simulink model "model1"  (R2024a)
settings: Solver=VariableStepAuto  StartTime=0.0  StopTime=simulation_time  RelTol=1e-3
values from neighbouring files (symbols this model uses):
  dq_0 = zeros(n, 1)    [example.m]
  path = @(t) circle_center + u_circle_plane*radius*cos((t/T) * (2*pi)) + v_circle_plane*radius*sin((t/T) * (2*pi))    [example.m]
  path_ddot = @(t) -u_circle_plane*radius*(2*pi/T)*(2*pi/T)*cos((t/T) * (2*pi)) - v_circle_plane*radius*(2*pi/T)*(2*pi/T)*sin((t/T) * (2*pi))    [example.m]
  path_dot = @(t) -u_circle_plane*radius*(2*pi/T)*sin((t/T) * (2*pi)) + v_circle_plane*radius*(2*pi/T)*cos((t/T) * (2*pi))    [example.m]
  q_0 = randn(n, 1)    [example.m]
  robot_model = importrobot("../robot_model/kuka-lwr-4plus/model1.urdf", 'DataFormat', 'column')    [example.m]
undefined symbols (not defined in the file or in its folder): torque_low_bound, torque_up_bound, X, Y, Z
libraries: sm_lib x74, nesl_utility x8, robotmaniplib x4
(part 4 of 5)

== matlab function model1/MATLAB Function5 ==
  data: currJointPos input; c_num output; currJointVel input
function c_num = c_num1(currJointPos, currJointVel)
%C_NUM1
%    C_NUM = C_NUM1(Q2,Q3,Q4,Q5,Q6,Q7,Q_DOT1,Q_DOT2,Q_DOT3,Q_DOT4,Q_DOT5,Q_DOT6,Q_DOT7)

%    This function was generated by the Symbolic Math Toolbox version 24.1.
%    01-Jul-2024 12:17:30

q_dot1 = currJointVel(1);
q2 = currJointPos(2);
q_dot2 = currJointVel(2);
q3 = currJointPos(3);
q_dot3 = currJointVel(3);
q4 = currJointPos(4);
q_dot4 = currJointVel(4);
q5 = currJointPos(5);
q_dot5 = currJointVel(5);
q6 = currJointPos(6);
q_dot6 = currJointVel(6);
q7 = currJointPos(7);
q_dot7 = currJointVel(7);


t2 = cos(q2);
t3 = cos(q3);
t4 = cos(q4);
t5 = cos(q5);
t6 = cos(q6);
t7 = cos(q7);
t8 = sin(q2);
t9 = sin(q3);
t10 = sin(q4);
t11 = sin(q5);
t12 = sin(q6);
t13 = sin(q7);
t14 = t3.^2;
t15 = t4.^2;
t16 = t5.^2;
t17 = t6.^2;
t18 = t7.^2;
t19 = t8.^2;
t20 = t9.^2;
t21 = t10.^2;
t22 = t11.^2;
t23 = t12.^2;
t24 = t13.^2;
t25 = t2.*t4;
t26 = t3.*t5;
t27 = t4.*t6;
t28 = t5.*t7;
t29 = t2.*t10;
t30 = t4.*t8;
t31 = t3.*t11;
t32 = t5.*t9;
t33 = t4.*t12;
t34 = t6.*t10;
t35 = t5.*t13;
t36 = t7.*t11;
t37 = t8.*t10;
t38 = t9.*t11;
t39 = t10.*t12;
t40 = t11.*t13;
t41 = t3.*(2.0./5.0);
t42 = t9.*(2.0./5.0);
t88 = t3.*(7.0./1.0e+2);
t89 = t9.*(7.0./1.0e+2);
t91 = t3.*t4.*(3.0./5.0e+1);
t92 = t3.*t10.*(-2.0./5.0);
t95 = t3.*t10.*(3.0./5.0e+1);
t96 = t4.*t9.*(3.0./5.0e+1);
t97 = t9.*t10.*(-2.0./5.0);
t100 = t9.*t10.*(3.0./5.0e+1);
t101 = t2.*(1.3e+1./1.0e+2);
t102 = t4.*(3.1e+1./2.5e+2);
t103 = t8.*(1.3e+1./1.0e+2);
t104 = t10.*(3.1e+1./2.5e+2);
t135 = t2.*t9.*(2.3e+1./5.0e+1);
t140 = t4.*t9.*(7.0./2.5e+2);
t142 = t8.*t9.*(2.3e+1./5.0e+1);
t145 = t3.*4.2e-3;
t146 = t2.*7.8e-3;
t147 = t9.*4.2e-3;
t148 = t8.*7.8e-3;
t182 = t4.*t11.*(3.9e+1./1.0e+2);
t194 = t10.*t11.*(3.9e+1./1.0e+2);
t198 = q_dot5.*t12.*6.0e-5;
t199 = q_dot6.*t12.*6.0e-5;
t200 = q_dot7.*t12.*6.0e-5;
t226 = t3.*t10.*(-3.1e+1./2.5e+2);
t228 = t3.*t10.*1.05e-2;
t236 = t6.*t12.*1.2e-4;
t275 = t2.*t9.*7.15e-2;
t278 = t2.*t9.*(-7.8e-3);
t279 = t2.*t9.*5.1e-3;
t282 = t3.*t10.*5.1e-3;
t283 = t3.*t10.*6.3e-3;
t285 = t9.*t10.*(-4.2e-3);
t286 = t8.*t9.*5.1e-3;
t287 = t9.*t10.*5.1e-3;
t296 = q_dot4.*t5.*t12.*6.0e-5;
t297 = q_dot4.*t6.*t11.*6.0e-5;
t299 = q_dot6.*t6.*t11.*6.0e-5;
t301 = q_dot7.*t6.*t11.*6.0e-5;
t393 = t2.*t9.*6.37e-2;
t394 = t4.*t11.*9.672e-2;
t395 = t5.*t10.*9.672e-2;
t422 = t3.*t4.*t9.*(-4.2e-3);
t752 = t2.*2.283333333335e-2;
t753 = t8.*2.283333333335e-2;
t754 = t3.*1.083333333335e-2;
t756 = t9.*1.083333333335e-2;
t867 = t11.*1.33541666666835e-3;
t868 = t9.*1.573333333335e-2;
t897 = t8.*3.973333333335e-2;
t918 = t5.*t10.*1.33541666666835e-3;
t922 = t3.*t8.*1.573333333335e-2;
t936 = t3.*t9.*7.82666666667e-2;
t951 = t2.*t8.*3.02666666667e-2;
t964 = t4.*t10.*1.133599999999999e-2;
t1081 = t5.*t11.*2.2065050000003e-1;
t1114 = t10.*3.751275000001835e-2;
t1208 = t4.*t9.*3.751275000001835e-2;
t1271 = t3.*t10.*(-3.751275000001835e-2);
t43 = t8.*t38;
t44 = t9.*t39;
t45 = t10.*t40;
t46 = t3.*t25;
t47 = t4.*t26;
t48 = t5.*t27;
t49 = t6.*t28;
t50 = t3.*t29;
t51 = t3.*t30;
t52 = t2.*t32;
t53 = t8.*t26;
t54 = t4.*t31;
t55 = t4.*t32;
t56 = t3.*t34;
t57 = t9.*t27;
t58 = t5.*t33;
t59 = t5.*t34;
t60 = t4.*t36;
t61 = t10.*t28;
t62 = t6.*t35;
t63 = t6.*t36;
t64 = t3.*t37;
t65 = t2.*t38;
t66 = t8.*t31;
t67 = t8.*t32;
t68 = t4.*t38;
t69 = t3.*t39;
t70 = t9.*t33;
t71 = t9.*t34;
t72 = t5.*t39;
t73 = t4.*t40;
t74 = t10.*t35;
t75 = t10.*t36;
t76 = t6.*t40;
t77 = t2.*t41;
t78 = t4.*t41;
t79 = t26.*(2.0./5.0);
t80 = t8.*t41;
t81 = t10.*t41;
t82 = t4.*t42;
t83 = t31.*(2.0./5.0);
t84 = t32.*(2.0./5.0);
t85 = t8.*t42;
t86 = t10.*t42;
t87 = t38.*(2.0./5.0);
t90 = t25.*(3.0./5.0e+1);
t93 = t29.*(3.0./5.0e+1);
t94 = t30.*(3.0./5.0e+1);
t99 = t37.*(3.0./5.0e+1);
t105 = t30.*t32;
t106 = t32.*t34;
t107 = t34.*t36;
t110 = t30.*t38;
t112 = t32.*t39;
t114 = t34.*t40;
t119 = t9.*t12.*t37;
t120 = t10.*t13.*t38;
t129 = t25.*(7.0./1.0e+2);
t130 = t4.*t88;
t131 = t37.*t42;
t133 = t39.*t42;
t136 = t2.*t89;
t137 = t8.*t88;
t138 = t29.*(7.0./1.0e+2);
t139 = t4.*t89;
t141 = -t100;
t143 = t8.*t89;
t144 = t37.*(7.0./1.0e+2);
t151 = t27.*t41;
t152 = t25.*t42;
t153 = t30.*t41;
t159 = t33.*t41;
t160 = t34.*t41;
t161 = t29.*t42;
t162 = t37.*t41;
t163 = t30.*t42;
t168 = t39.*t41;
t169 = t34.*t42;
t170 = t26.*(3.9e+1./1.0e+2);
t171 = t28.*(3.9e+1./1.0e+2);
t172 = t25.*(3.1e+1./2.5e+2);
t173 = t26.*(3.1e+1./2.5e+2);
t174 = t26.*1.5e-3;
t175 = t9.*t37.*(-2.0./5.0);
t178 = -t135;
t180 = t31.*(3.9e+1./1.0e+2);
t181 = t32.*(3.9e+1./1.0e+2);
t183 = t35.*(3.9e+1./1.0e+2);
t184 = t36.*(3.9e+1./1.0e+2);
t186 = t29.*(3.1e+1./2.5e+2);
t187 = t30.*(3.1e+1./2.5e+2);
t189 = t9.*t102;
t190 = t31.*(3.1e+1./2.5e+2);
t191 = t31.*1.5e-3;
t192 = t32.*1.5e-3;
t193 = t38.*(3.9e+1./1.0e+2);
t195 = t40.*(3.9e+1./1.0e+2);
t196 = t9.*t104;
t197 = t38.*(3.1e+1./2.5e+2);
t209 = t10.*t26.*(-2.0./5.0);
t213 = t9.*t29.*(-2.0./5.0);
t215 = t9.*t30.*(-2.0./5.0);
t221 = t25.*4.2e-3;
t222 = t27.*6.0e-5;
t223 = t9.*t37.*(-3.0./5.0e+1);
t224 = -t182;
t227 = t31.*(3.1e+1./6.25e+2);
t229 = t30.*8.4e-3;
t230 = t2.*t147;
t231 = t8.*t145;
t232 = t29.*4.2e-3;
t233 = t30.*4.2e-3;
t234 = t10.*t145;
t237 = t33.*6.0e-5;
t238 = t34.*6.0e-5;
t241 = t8.*t147;
t243 = t9.*t148;
t261 = t9.*t25.*(7.0./2.5e+2);
t266 = t30.*t89;
t267 = t25.*5.1e-3;
t271 = t9.*t37.*(3.1e+1./2.5e+2);
t280 = t29.*5.1e-3;
t281 = t30.*5.1e-3;
t284 = -t236;
t298 = t5.*t198;
t300 = t5.*t200;
t343 = t32.*t104;
t347 = t9.*t37.*1.05e-2;
t350 = t12.*t38.*6.0e-5;
t351 = -t275;
t352 = -t279;
t354 = -t283;
t355 = -t287;
t360 = t10.*t26.*(3.1e+1./6.25e+2);
t366 = t3.*t8.*t146;
t367 = t12.*t25.*6.0e-5;
t368 = t6.*t29.*6.0e-5;
t372 = t12.*t26.*6.0e-5;
t373 = t6.*t31.*6.0e-5;
t390 = t9.*t37.*(-4.2e-3);
t391 = t9.*t37.*5.1e-3;
t392 = t9.*t37.*6.3e-3;
t396 = t32.*4.836e-2;
t405 = q_dot3.*t11.*t39.*6.0e-5;
t406 = q_dot5.*t11.*t39.*6.0e-5;
t407 = q_dot7.*t11.*t39.*6.0e-5;
t423 = t9.*t25.*2.1e-3;
t433 = -t393;
t434 = -t394;
t449 = t28.*t34.*(-3.9e+1./1.0e+2);
t450 = t25.*t32.*(3.1e+1./6.25e+2);
t451 = t26.*t30.*(3.1e+1./6.25e+2);
t461 = t32.*t37.*(3.1e+1./6.25e+2);
t469 = t11.*t12.*t29.*6.0e-5;
t470 = t5.*t12.*t37.*6.0e-5;
t475 = t11.*t37.*4.836e-2;
t476 = t10.*t38.*4.836e-2;
t480 = t20.*t30.*2.1e-3;
t485 = t5.*t6.*t29.*(-6.0e-5);
t486 = t26.*t33.*(-6.0e-5);
t492 = t33.*t38.*(-6.0e-5);
t495 = t11.*t25.*4.836e-2;
t519 = t12.*t30.*t31.*6.0e-5;
t528 = t6.*t12.*t16.*3.042e-2;
t530 = t91+t97;
t531 = t25.*t31.*4.836e-2;
t532 = t31.*t37.*4.836e-2;
t542 = t101+t142;
t547 = t102+t194;
t564 = t4.*t10.*t17.*t22.*1.521e-1;
t565 = t5.*t11.*t17.*t21.*1.521e-1;
t568 = t4.*t10.*t22.*t23.*1.8252e-1;
t569 = t5.*t11.*t21.*t23.*1.8252e-1;
t570 = t6.*t12.*t21.*t22.*3.042e-2;
t586 = t147+t282;
t587 = t146+t286;
t779 = t29.*2.080133333335e-2;
t780 = t30.*2.080133333335e-2;
t785 = t2.*t756;
t786 = t8.*t754;
t787 = t8.*t756;
t789 = t25.*1.533333333335e-2;
t791 = t29.*1.533333333335e-2;
t794 = t37.*1.533333333335e-2;
t796 = t26.*2.170133333335e-2;
t797 = t31.*2.170133333335e-2;
t799 = t25.*2.080133333335e-2;
t800 = t38.*2.170133333335e-2;
t804 = t26.*1.302083333335e-3;
t805 = t27.*1.302083333335e-3;
t806 = t31.*1.302083333335e-3;
t807 = t32.*1.302083333335e-3;
t808 = t33.*1.302083333335e-3;
t809 = t34.*1.302083333335e-3;
t810 = t39.*1.302083333335e-3;
t870 = t28.*3.333333333335e-5;
t873 = t35.*3.333333333335e-5;
t874 = t36.*3.333333333335e-5;
t875 = t40.*3.333333333335e-5;
t890 = t3.*t9.*t21.*4.16026666667e-2;
t896 = -t868;
t900 = t3.*t9.*t15.*3.06666666667e-2;
t915 = t31.*1.33541666666835e-3;
t916 = t32.*1.33541666666835e-3;
t917 = t4.*t867;
t921 = t2.*t868;
t949 = t8.*t15.*t20.*1.533333333335e-2;
t954 = t9.*t16.*t21.*2.170133333335e-2;
t962 = t8.*t20.*t21.*2.080133333335e-2;
t963 = -t936;
t969 = t8.*t14.*3.913333333335e-2;
t972 = t8.*t20.*2.5328333333335e-1;
t975 = t25.*t867;
t976 = t5.*t29.*1.33541666666835e-3;
t979 = t9.*t21.*3.117999999999997e-3;
t982 = t37.*t867;
t983 = t10.*t38.*1.33541666666835e-3;
t984 = -t951;
t992 = t6.*t12.*t18.*6.66666666667e-5;
t997 = t6.*t12.*t24.*6.66666666667e-5;
t1007 = t9.*t15.*1.0568e-2;
t1025 = t2.*t8.*t14.*5.116666666667e-1;
t1040 = t3.*t9.*t19.*5.065666666667e-1;
t1042 = t26.*t30.*1.33541666666835e-3;
t1063 = t4.*t10.*t22.*5.60416666667e-3;
t1065 = t4.*t10.*t20.*1.603599999999999e-2;
t1089 = t10.*t17.*2.666666666665e-5;
t1090 = t11.*t17.*2.666666666665e-5;
t1091 = t11.*t23.*2.666666666665e-5;
t1094 = -t1081;
t1099 = t9.*t21.*t22.*2.802083333335e-3;
t1101 = t12.*t27.*5.33333333333e-5;
t1103 = t278+t753;
t1107 = t285+t754;
t1113 = t5.*t11.*t23.*1.7979583333333e-1;
t1125 = t5.*t11.*t17.*1.4949583333333e-1;
t1128 = t23.*t31.*2.666666666665e-5;
t1130 = t5.*t10.*t23.*2.666666666665e-5;
t1145 = t6.*t12.*t25.*5.33333333333e-5;
t1149 = t6.*t12.*t38.*2.666666666665e-5;
t1150 = t11.*t12.*t34.*5.33333333333e-5;
t1151 = t4.*t10.*t16.*5.304546666667e-1;
t1165 = t17.*t29.*2.666666666665e-5;
t1166 = t17.*t30.*2.666666666665e-5;
t1168 = t4.*t9.*t17.*2.666666666665e-5;
t1169 = t17.*t31.*2.666666666665e-5;
t1177 = t4.*t11.*t23.*(-2.666666666665e-5);
t1205 = t29.*3.751275000001835e-2;
t1206 = t30.*3.751275000001835e-2;
t1207 = t3.*t1114;
t1213 = t4.*t11.*t17.*(-2.666666666665e-5);
t1214 = t5.*t10.*t17.*(-2.666666666665e-5);
t1230 = t5.*t6.*t12.*t25.*2.666666666665e-5;
t1231 = t12.*t26.*t27.*2.666666666665e-5;
t1248 = t5.*t11.*t21.*5.2485050000003e-1;
t1266 = t5.*t23.*t29.*2.666666666665e-5;
t1268 = t9.*t17.*t37.*2.666666666665e-5;
t1284 = t10.*t16.*t17.*(-2.666666666665e-5);
t1290 = t10.*t17.*t22.*(-2.666666666665e-5);
t1291 = t10.*t16.*3.560400000001665e-2;
t1292 = t10.*t22.*3.560400000001665e-2;
t1307 = t5.*t17.*t29.*(-2.666666666665e-5);
t1313 = t9.*t37.*3.751275000001835e-2;
t1320 = t6.*t12.*t25.*t26.*2.666666666665e-5;
t1338 = t23.*t26.*t30.*2.666666666665e-5;
t98 = -t87;
t108 = -t47;
t109 = -t49;
t111 = t8.*t71;
t113 = t9.*t75;
t115 = -t50;
t116 = -t51;
t117 = -t58;
t118 = -t59;
t123 = -t68;
t128 = -t76;
t132 = t43.*(2.0./5.0);
t134 = -t94;
t150 = t47.*(2.0./5.0);
t154 = t2.*t83;
t155 = t53.*(2.0./5.0);
t156 = t54.*(2.0./5.0);
t157 = t10.*t79;
t158 = t55.*(2.0./5.0);
t164 = t66.*(2.0./5.0);
t165 = t67.*(2.0./5.0);
t166 = t10.*t83;
t167 = t68.*(2.0./5.0);
t179 = -t138;
t201 = -t106;
t203 = t46.*(3.0./5.0e+1);
t204 = -t110;
t207 = -t114;
t211 = t50.*(3.0./5.0e+1);
t212 = t51.*(3.0./5.0e+1);
t214 = t64.*(-2.0./5.0);
t219 = t64.*(3.0./5.0e+1);
t220 = t9.*t94;
t225 = -t186;
t239 = -t193;
t240 = -t197;
t244 = t25.*t84;
t245 = t30.*t79;
t246 = t25.*t87;
t247 = t30.*t83;
t248 = t30.*t84;
t251 = t27.*t85;
t252 = t46.*(7.0./1.0e+2);
t253 = t30.*t87;
t254 = t37.*t84;
t255 = t12.*t161;
t256 = t12.*t162;
t260 = t51.*(7.0./1.0e+2);
t262 = t51.*(7.0./2.5e+2);
t264 = t12.*t131;
t265 = t64.*(7.0./1.0e+2);
t268 = t43.*(3.9e+1./1.0e+2);
t269 = t10.*t193;
t270 = t45.*(3.9e+1./1.0e+2);
t272 = t43.*(3.1e+1./2.5e+2);
t273 = t43.*1.5e-3;
t274 = -t227;
t276 = -t229;
t277 = -t233;
t288 = t25+t64;
t289 = t37+t46;
t290 = t31+t55;
t291 = t32+t54;
t292 = t27+t72;
t293 = t39+t48;
t294 = t35+t63;
t295 = t36+t62;
t304 = t105.*(-2.0./5.0);
t305 = t6.*t213;
t306 = t47.*(3.9e+1./1.0e+2);
t307 = t4.*t171;
t308 = t49.*(3.9e+1./1.0e+2);
t309 = t47.*(3.1e+1./2.5e+2);
t311 = t12.*t215;
t313 = t52.*(3.9e+1./1.0e+2);
t314 = t53.*(3.9e+1./1.0e+2);
t315 = t54.*(3.9e+1./1.0e+2);
t316 = t55.*(3.9e+1./1.0e+2);
t317 = t4.*t183;
t318 = t61.*(3.9e+1./1.0e+2);
t319 = t62.*(3.9e+1./1.0e+2);
t320 = t63.*(3.9e+1./1.0e+2);
t322 = t50.*(3.1e+1./2.5e+2);
t323 = t51.*(3.1e+1./2.5e+2);
t324 = t55.*(3.1e+1./2.5e+2);
t325 = t52.*1.5e-3;
t326 = t53.*1.5e-3;
t327 = t54.*1.5e-3;
t328 = t55.*1.5e-3;
t330 = t65.*(3.9e+1./1.0e+2);
t331 = t66.*(3.9e+1./1.0e+2);
t332 = t67.*(3.9e+1./1.0e+2);
t333 = t68.*(3.9e+1./1.0e+2);
t334 = t10.*t181;
t335 = t74.*(3.9e+1./1.0e+2);
t336 = t75.*(3.9e+1./1.0e+2);
t337 = t76.*(3.9e+1./1.0e+2);
t338 = t64.*(3.1e+1./2.5e+2);
t339 = t65.*(3.1e+1./2.5e+2);
t340 = t66.*(3.1e+1./2.5e+2);
t341 = t67.*(3.1e+1./2.5e+2);
t342 = t68.*(3.1e+1./2.5e+2);
t344 = t67.*1.5e-3;
t345 = t68.*1.5e-3;
t346 = t43.*(3.1e+1./6.25e+2);
t349 = t44.*6.0e-5;
t353 = -t281;
t359 = t2.*t227;
t361 = t55.*(3.1e+1./6.25e+2);
t362 = t50.*8.4e-3;
t363 = t50.*4.2e-3;
t364 = t51.*4.2e-3;
t369 = t8.*t222;
t370 = t56.*6.0e-5;
t371 = t57.*6.0e-5;
t374 = t58.*6.0e-5;
t375 = t59.*6.0e-5;
t385 = t64.*4.2e-3;
t386 = t71.*6.0e-5;
t387 = t72.*6.0e-5;
t389 = -t347;
t408 = t27.*t184;
t410 = t105.*(3.9e+1./1.0e+2);
t411 = t27.*t195;
t412 = t34.*t183;
t413 = t107.*(3.9e+1./1.0e+2);
t414 = t105.*(3.1e+1./2.5e+2);
t415 = t110.*(3.9e+1./1.0e+2);
t416 = t114.*(3.9e+1./1.0e+2);
t417 = t110.*1.5e-3;
t418 = -t360;
t424 = t50.*5.1e-3;
t425 = t51.*5.1e-3;
t426 = -t368;
t429 = t64.*5.1e-3;
c_num = ft_1({q_dot1,q_dot2,q_dot3,q_dot4,q_dot5,q_dot6,q_dot7,t10,t1007,t102,t1025,t103,t104,t1040,t1042,t105,t106,t1063,t1065,t107,t108,t1089,t109,t1090,t1091,t1094,t1099,t11,t110,t1101,t1103,t1107,t111,t1113,t1114,t112,t1125,t1128,t113,t1130,t114,t1145,t1149,t115,t1150,t1151,t116,t1165,t1166,t1168,t1169,t117,t1177,t118,t119,t12,t120,t1205,t1206,t1207,t1208,t1213,t1214,t123,t1230,t1231,t1248,t1266,t1268,t1271,t128,t1284,t129,t1290,t1291,t1292,t13,t130,t1307,t131,t1313,t132,t1320,t133,t1338,t134,t136,t137,t139,t140,t141,t143,t144,t145,t147,t148,t150,t151,t152,t153,t154,t155,t156,t157,t158,t159,t16,t160,t161,t162,t163,t164,t165,t166,t167,t168,t169,t17,t170,t171,t172,t173,t174,t175,t178,t179,t180,t181,t183,t184,t187,t189,t190,t191,t192,t195,t196,t198,t199,t2,t200,t201,t203,t204,t207,t209,t211,t212,t213,t214,t219,t22,t220,t221,t222,t223,t224,t225,t226,t227,t228,t23,t230,t231,t232,t234,t237,t238,t239,t240,t241,t243,t244,t245,t246,t247,t248,t25,t251,t252,t253,t254,t255,t256,t26,t260,t261,t262,t264,t265,t266,t267,t268,t269,t27,t270,t271,t272,t273,t274,t276,t277,t28,t280,t284,t288,t289,t29,t290,t291,t292,t293,t294,t295,t296,t297,t298,t299,t3,t30,t300,t301,t304,t305,t306,t307,t308,t309,t31,t311,t313,t314,t315,t316,t317,t318,t319,t32,t320,t322,t323,t324,t325,t326,t327,t328,t33,t330,t331,t332,t333,t334,t335,t336,t337,t338,t339,t34,t340,t341,t342,t343,t344,t345,t346,t349,t35,t350,t351,t352,t353,t354,t355,t359,t36,t361,t362,t363,t364,t366,t367,t369,t37,t370,t371,t372,t373,t374,t375,t38,t385,t386,t387,t389,t39,t390,t391,t392,t395,t396,t4,t40,t405,t406,t407,t408,t41,t410,t411,t412,t413,t414,t415,t416,t417,t418,t42,t422,t423,t424,t425,t426,t429,t43,t433,t434,t44,t449,t45,t450,t451,t46,t461,t469,t47,t470,t475,t476,t48,t480,t485,t486,t49,t492,t495,t5,t50,t51,t519,t52,t528,t53,t530,t531,t532,t54,t542,t547,t55,t56,t564,t565,t568,t569,t57,t570,t58,t586,t587,t59,t6,t60,t61,t62,t63,t64,t65,t66,t67,t68,t69,t7,t70,t71,t72,t73,t74,t75,t752,t756,t76,t77,t779,t78,t780,t785,t786,t787,t789,t79,t791,t794,t796,t797,t799,t8,t80,t800,t804,t805,t806,t807,t808,t809,t81,t810,t82,t83,t84,t85,t86,t867,t868,t870,t873,t874,t875,t88,t89,t890,t896,t897,t9,t90,t900,t915,t916,t917,t918,t92,t921,t922,t93,t949,t95,t954,t96,t962,t963,t964,t969,t972,t975,t976,t979,t98,t982,t983,t984,t99,t992,t997});
end
function c_num = ft_1(ct)
[q_dot1,q_dot2,q_dot3,q_dot4,q_dot5,q_dot6,q_dot7,t10,t1007,t102,t1025,t103,t104,t1040,t1042,t105,t106,t1063,t1065,t107,t108,t1089,t109,t1090,t1091,t1094,t1099,t11,t110,t1101,t1103,t1107,t111,t1113,t1114,t112,t1125,t1128,t113,t1130,t114,t1145,t1149,t115,t1150,t1151,t116,t1165,t1166,t1168,t1169,t117,t1177,t118,t119,t12,t120,t1205,t1206,t1207,t1208,t1213,t1214,t123,t1230,t1231,t1248,t1266,t1268,t1271,t128,t1284,t129,t1290,t1291,t1292,t13,t130,t1307,t131,t1313,t132,t1320,t133,t1338,t134,t136,t137,t139,t140,t141,t143,t144,t145,t147,t148,t150,t151,t152,t153,t154,t155,t156,t157,t158,t159,t16,t160,t161,t162,t163,t164,t165,t166,t167,t168,t169,t17,t170,t171,t172,t173,t174,t175,t178,t179,t180,t181,t183,t184,t187,t189,t190,t191,t192,t195,t196,t198,t199,t2,t200,t201,t203,t204,t207,t209,t211,t212,t213,t214,t219,t22,t220,t221,t222,t223,t224,t225,t226,t227,t228,t23,t230,t231,t232,t234,t237,t238,t239,t240,t241,t243,t244,t245,t246,t247,t248,t25,t251,t252,t253,t254,t255,t256,t26,t260,t261,t262,t264,t265,t266,t267,t268,t269,t27,t270,t271,t272,t273,t274,t276,t277,t28,t280,t284,t288,t289,t29,t290,t291,t292,t293,t294,t295,t296,t297,t298,t299,t3,t30,t300,t301,t304,t305,t306,t307,t308,t309,t31,t311,t313,t314,t315,t316,t317,t318,t319,t32,t320,t322,t323,t324,t325,t326,t327,t328,t33,t330,t331,t332,t333,t334,t335,t336,t337,t338,t339,t34,t340,t341,t342,t343,t344,t345,t346,t349,t35,t350,t351,t352,t353,t354,t355,t359,t36,t361,t362,t363,t364,t366,t367,t369,t37,t370,t371,t372,t373,t374,t375,t38,t385,t386,t387,t389,t39,t390,t391,t392,t395,t396,t4,t40,t405,t406,t407,t408,t41,t410,t411,t412,t413,t414,t415,t416,t417,t418,t42,t422,t423,t424,t425,t426,t429,t43,t433,t434,t44,t449,t45,t450,t451,t46,t461,t469,t47,t470,t475,t476,t48,t480,t485,t486,t49,t492,t495,t5,t50,t51,t519,t52,t528,t53,t530,t531,t532,t54,t542,t547,t55,t56,t564,t565,t568,t569,t57,t570,t58,t586,t587,t59,t6,t60,t61,t62,t63,t64,t65,t66,t67,t68,t69,t7,t70,t71,t72,t73,t74,t75,t752,t756,t76,t77,t779,t78,t780,t785,t786,t787,t789,t79,t791,t794,t796,t797,t799,t8,t80,t800,t804,t805,t806,t807,t808,t809,t81,t810,t82,t83,t84,t85,t86,t867,t868,t870,t873,t874,t875,t88,t89,t890,t896,t897,t9,t90,t900,t915,t916,t917,t918,t92,t921,t922,t93,t949,t95,t954,t96,t962,t963,t964,t969,t972,t975,t976,t979,t98,t982,t983,t984,t99,t992,t997] = ct{:};
t431 = -t391;
t432 = -t392;
t435 = -t396;
t452 = t6.*t50.*6.0e-5;
t454 = t5.*t367;
t457 = t32.*t222;
t463 = t12.*t64.*6.0e-5;
t465 = t12.*t65.*6.0e-5;
t466 = t12.*t66.*6.0e-5;
t467 = t12.*t67.*6.0e-5;
t468 = t6.*t43.*6.0e-5;
t472 = t112.*6.0e-5;
t473 = -t423;
t477 = t66+t105;
t478 = t57+t112;
t479 = t74+t107;
t481 = t41+t130;
t482 = t42+t139;
t483 = -t451;
t491 = -t469;
t493 = t52.*4.836e-2;
t494 = t53.*4.836e-2;
t496 = t54.*4.836e-2;
t502 = t81+t96;
t503 = t26.*t367;
t504 = t53.*t222;
t520 = t37.*t372;
t521 = t12.*t105.*6.0e-5;
t529 = t78+t141;
t533 = t110.*4.836e-2;
t545 = t85+t266;
t546 = t103+t178;
t551 = t78+t343;
t562 = t104+t224;
t600 = t145+t355;
t601 = t148+t352;
t612 = t82+t89+t95;
t637 = t9.*t542.*(2.3e+1./5.0e+1);
t649 = t2.*t9.*t587;
t650 = t3.*t8.*t587;
t651 = t9.*t10.*t586;
t665 = t3.*t8.*t542.*(2.3e+1./2.5e+1);
t669 = (t9.*t587)./2.0;
t680 = t5.*t10.*t547.*(3.9e+1./5.0e+1);
t685 = t372+t492;
t699 = t137+t153+t223;
t824 = t46.*1.533333333335e-2;
t827 = t51.*1.533333333335e-2;
t828 = t64.*1.533333333335e-2;
t830 = t47.*2.170133333335e-2;
t831 = t55.*2.170133333335e-2;
t832 = t65.*2.170133333335e-2;
t833 = t66.*2.170133333335e-2;
t834 = t67.*2.170133333335e-2;
t835 = t68.*2.170133333335e-2;
t836 = t50.*2.080133333335e-2;
t837 = t51.*2.080133333335e-2;
t838 = t43.*2.170133333335e-2;
t839 = t64.*2.080133333335e-2;
t844 = t48.*1.302083333335e-3;
t845 = t52.*1.302083333335e-3;
t846 = t53.*1.302083333335e-3;
t847 = t54.*1.302083333335e-3;
t848 = t55.*1.302083333335e-3;
t849 = t56.*1.302083333335e-3;
t850 = t57.*1.302083333335e-3;
t851 = t58.*1.302083333335e-3;
t852 = t59.*1.302083333335e-3;
t855 = t67.*1.302083333335e-3;
t856 = t68.*1.302083333335e-3;
t857 = t69.*1.302083333335e-3;
t858 = t70.*1.302083333335e-3;
t859 = t71.*1.302083333335e-3;
t860 = t72.*1.302083333335e-3;
t861 = t43.*1.302083333335e-3;
t862 = t44.*1.302083333335e-3;
t898 = t105.*2.170133333335e-2;
t906 = t106.*1.302083333335e-3;
t908 = t110.*1.302083333335e-3;
t910 = t112.*1.302083333335e-3;
t912 = t119.*1.302083333335e-3;
t914 = -t890;
t923 = t49.*3.333333333335e-5;
t925 = t60.*3.333333333335e-5;
t926 = t61.*3.333333333335e-5;
t927 = t62.*3.333333333335e-5;
t928 = t63.*3.333333333335e-5;
t929 = t73.*3.333333333335e-5;
t930 = t74.*3.333333333335e-5;
t931 = t75.*3.333333333335e-5;
t932 = t76.*3.333333333335e-5;
t934 = t45.*3.333333333335e-5;
t938 = -t900;
t973 = t52.*1.33541666666835e-3;
t974 = t53.*1.33541666666835e-3;
t977 = t54.*1.33541666666835e-3;
t978 = t55.*1.33541666666835e-3;
t980 = -t949;
t981 = t43.*1.33541666666835e-3;
t985 = t107.*3.333333333335e-5;
t987 = t114.*3.333333333335e-5;
t988 = t120.*3.333333333335e-5;
t990 = -t962;
t1004 = -t969;
t1008 = -t972;
t1011 = -t976;
t1014 = -t979;
t1041 = t25.*t915;
t1048 = t37.*t915;
t1049 = t110.*1.33541666666835e-3;
t1053 = -t1025;
t1062 = -t1040;
t1064 = -t1042;
t1080 = -t1063;
t1086 = t243+t752;
t1087 = t234+t756;
t1115 = -t1090;
t1116 = -t1091;
t1123 = -t1101;
t1129 = t4.*t1091;
t1146 = t12.*t48.*5.33333333333e-5;
t1148 = t12.*t71.*5.33333333333e-5;
t1167 = t3.*t1089;
t1170 = t4.*t1090;
t1171 = t5.*t1089;
t1176 = -t1128;
t1178 = -t1130;
t1181 = t9.*t1107;
t1197 = -t1151;
t1209 = -t1165;
t1212 = -t1169;
t1217 = t2.*t1103;
t1236 = t16.*t1089;
t1238 = t8.*t12.*t56.*5.33333333333e-5;
t1239 = t6.*t12.*t65.*2.666666666665e-5;
t1240 = t6.*t12.*t66.*2.666666666665e-5;
t1241 = t8.*t12.*t59.*2.666666666665e-5;
t1242 = t12.*t106.*2.666666666665e-5;
t1243 = t11.*t12.*t59.*5.33333333333e-5;
t1245 = t22.*t1089;
t1251 = t390+t786;
t1260 = t17.*t50.*2.666666666665e-5;
t1261 = t17.*t51.*2.666666666665e-5;
t1263 = t17.*t55.*2.666666666665e-5;
t1267 = t23.*t55.*2.666666666665e-5;
t1269 = t17.*t43.*2.666666666665e-5;
t1270 = -t1205;
t1273 = t23.*t43.*2.666666666665e-5;
t1279 = -t1230;
t1280 = -t1231;
t1297 = t50.*3.751275000001835e-2;
t1298 = t51.*3.751275000001835e-2;
t1314 = -t1268;
t1323 = t12.*t34.*t53.*2.666666666665e-5;
t1324 = t12.*t27.*t67.*2.666666666665e-5;
t1331 = -t1291;
t1332 = -t1292;
t1336 = t26.*t1166;
t1352 = -t1313;
t1370 = -t1338;
t1378 = (t3.*t8.*t1107)./2.0;
t1980 = t284+t992+t997;
t2571 = t918+t1101+t1130+t1214;
t176 = -t132;
t208 = -t155;
t216 = -t164;
t217 = -t167;
t259 = -t212;
t356 = -t308;
t358 = -t322;
t377 = -t332;
t378 = -t333;
t379 = -t337;
t380 = -t339;
t382 = -t342;
t384 = -t345;
t388 = -t346;
t397 = t29+t116;
t398 = t30+t115;
t399 = t26+t123;
t400 = t38+t108;
t401 = t33+t118;
t402 = t34+t117;
t403 = t28+t128;
t404 = t40+t109;
t419 = -t361;
t421 = -t364;
t427 = -t374;
t428 = -t375;
t437 = t5.*t289;
t438 = t6.*t288;
t439 = t6.*t290;
t440 = t7.*t290;
t441 = t7.*t291;
t442 = t7.*t293;
t443 = t11.*t289;
t444 = t12.*t288;
t445 = t12.*t290;
t446 = t13.*t290;
t447 = t13.*t291;
t448 = t13.*t293;
t453 = t3.*t369;
t459 = -t415;
t460 = -t416;
t462 = -t417;
t464 = t111.*6.0e-5;
t474 = -t425;
t484 = -t452;
t489 = -t465;
t490 = -t468;
t500 = t36.*t288;
t501 = t40.*t288;
t522 = -t494;
t524 = -t496;
t525 = t53+t204;
t526 = t70+t201;
t527 = t61+t207;
t534 = t6.*t477;
t536 = t12.*t477;
t544 = -t533;
t548 = t162+t220;
t555 = t5.*t288.*(3.9e+1./1.0e+2);
t557 = t5.*t288.*(3.1e+1./2.5e+2);
t559 = t11.*t288.*(3.9e+1./1.0e+2);
t563 = t129+t265;
t574 = t166+t334;
t590 = t209+t269;
t591 = t183+t320;
t592 = t184+t319;
t593 = t191+t328;
t594 = t192+t327;
t602 = t4.*t482.*(7.0./1.0e+2);
t611 = t10.*t529.*(3.0./5.0e+1);
t613 = t9.*t10.*t482.*(7.0./5.0e+1);
t622 = t222+t387;
t626 = t88+t529;
t634 = -t6.*(t157-t10.*t38.*(3.9e+1./1.0e+2));
t638 = t317+t408;
t640 = t335+t413;
t641 = t336+t412;
t647 = t231+t431;
t652 = -t637;
t654 = t270+t449;
t666 = t3.*t10.*t600;
t667 = t4.*t9.*t600;
t668 = t8.*t9.*t601;
t671 = t371+t472;
t675 = t90+t163+t219;
t676 = t77+t144+t252;
t682 = -t651;
t683 = (t10.*t600)./2.0;
t684 = -t669;
t686 = t99+t203+t213;
t688 = t80+t179+t260;
t701 = t5.*t104.*t551;
t712 = t92+t190+t324;
t715 = t86+t240+t309;
t720 = q_dot2.*t685;
t721 = q_dot5.*t685;
t722 = q_dot7.*t685;
t726 = (t9.*t37.*t600)./2.0;
t736 = t481.*t482.*2.0;
t771 = t502.*t529.*2.0;
t772 = t502.*t530.*2.0;
t774 = t482.*t545;
t784 = t214+t340+t414;
t812 = (t288.*t586)./2.0;
t814 = t241+t267+t429;
t823 = t134+t136+t152+t211;
t825 = t230+t353+t424;
t863 = t83+t158+t181+t315;
t864 = t84+t156+t180+t316;
t866 = -t827;
t871 = -t830;
t876 = -t832;
t877 = -t834;
t878 = -t835;
t880 = t542.*t546.*2.0;
t881 = -t836;
t882 = -t837;
t888 = -t851;
t889 = -t852;
t891 = -t855;
t892 = -t856;
t893 = -t857;
t894 = -t859;
t904 = t349+t373+t457;
t909 = t111.*1.302083333335e-3;
t937 = t547.*t562.*2.0;
t940 = t350+t370+t486;
t941 = -t906;
t945 = -t908;
t952 = -t923;
t955 = -t929;
t956 = -t931;
t957 = -t932;
t986 = t113.*3.333333333335e-5;
t1009 = -t974;
t1016 = -t981;
t1019 = -t987;
t1068 = -t1049;
t1088 = t165+t247+t331+t410;
t1092 = t10.*t289.*7.666666666675001e-3;
t1106 = t467+t491+t519;
t1118 = t3.*t10.*t288.*1.0400666666675e-2;
t1131 = t8.*t1086;
t1132 = t3.*t1087;
t1138 = t4.*t5.*t290.*1.0850666666675e-2;
t1160 = t11.*t39.*(t151+t12.*(t157-t10.*t38.*(3.9e+1./1.0e+2))).*(-1.17e+2./5.0e+2);
t1182 = t10.*t32.*t290.*2.170133333335e-2;
t1185 = t9.*t37.*t288.*2.080133333335e-2;
t1188 = -t1146;
t1192 = -t1148;
t1201 = t10.*t16.*t288.*2.170133333335e-2;
t1233 = t11.*t477.*1.0850666666675e-2;
t1285 = -t1239;
t1286 = -t1240;
t1288 = -t1243;
t1289 = t10.*t288.*5.283999999999999e-3;
t1305 = -t1260;
t1306 = -t1261;
t1308 = -t1263;
t1311 = -t1267;
t1315 = -t1269;
t1328 = t5.*t291.*1.4010416666675e-3;
t1342 = -t1297;
t1343 = -t1298;
t1355 = (t8.*t9.*t1087)./2.0;
t1356 = -t1323;
t1357 = -t1324;
t1358 = t4.*t9.*t288.*5.283999999999999e-3;
t1364 = t5.*t290.*9.4496250000075e-3;
t1377 = t12.*t36.*t294.*(-3.333333333335e-5);
t1398 = -t1378;
t1403 = t10.*t11.*t290.*9.4496250000075e-3;
t1409 = t10.*t22.*t288.*2.802083333335e-3;
t1414 = t8.*t9.*t1251;
t1423 = (t3.*t1251)./2.0;
t1441 = t11.*t39.*t292.*1.362083333335e-3;
t1463 = t5.*t288.*t290.*1.0850666666675e-2;
t1490 = t221+t385+t787;
t1502 = t277+t363+t785;
t1671 = t797+t831;
t1673 = t799+t839;
t1677 = t789+t828;
t1678 = t794+t824;
t1693 = t806+t848;
t1694 = t807+t847;
t1695 = t805+t860;
t1696 = t810+t844;
t1719 = t833+t898;
t1735 = t873+t928;
t1736 = t874+t927;
t1741 = t850+t910;
t1828 = t930+t985;
t2005 = q_dot5.*t1980;
t2348 = t867+t1091+t1115;
t2349 = t867+t1090+t1116;
t2572 = t918+t1123+t1171+t1178;
t2577 = t917+t1170+t1177+t1243;
t2655 = t1089+t1114+t1245+t1284+t1291+t1332;
t488 = -t464;
t498 = t5.*t438;
t499 = t5.*t444;
t505 = t5.*t397;
t506 = t6.*t397;
t507 = t6.*t398;
t508 = t6.*t400;
t509 = t7.*t399;
t511 = t7.*t401;
t512 = t11.*t397;
t513 = t12.*t397;
t514 = t12.*t398;
t516 = t12.*t400;
t517 = t13.*t399;
t518 = t13.*t401;
t549 = t7.*t525;
t550 = t7.*t526;
t553 = t13.*t525;
t554 = t13.*t526;
t556 = t437.*(3.9e+1./1.0e+2);
t558 = t437.*(3.1e+1./2.5e+2);
t560 = t443.*(3.9e+1./1.0e+2);
t561 = t443.*1.5e-3;
t566 = t438.*6.0e-5;
t567 = t439.*6.0e-5;
t571 = t444.*6.0e-5;
t572 = t445.*6.0e-5;
t573 = t44+t439;
t588 = t52+t443;
t589 = t60+t448;
t606 = t171+t379;
t607 = t195+t356;
t608 = t173+t382;
t609 = t174+t384;
t614 = -t602;
t623 = t536.*6.0e-5;
t624 = t7.*t574;
t625 = t13.*t574;
t627 = -t611;
t628 = -t613;
t631 = t232+t421;
t632 = t237+t428;
t633 = t238+t427;
t643 = -t12.*(t65-t437);
t655 = t318+t460;
t656 = t326+t462;
t663 = t280+t474;
t664 = t119+t534;
t677 = (t5.*t593)./2.0;
t678 = (t5.*t594)./2.0;
t679 = t10.*t563.*(7.0./1.0e+2);
t687 = t93+t131+t259;
t696 = -t667;
t702 = (t10.*t11.*t593)./2.0;
t707 = q_dot2.*t671;
t708 = q_dot4.*t671;
t709 = q_dot7.*t671;
t710 = t10.*t626.*(3.0./5.0e+1);
t711 = t11.*t39.*t622;
t727 = t254+t559;
t730 = t12.*(t65-t437).*(-6.0e-5);
t733 = t189+t590;
t734 = t5.*t10.*t574.*(1.17e+2./2.0e+2);
t737 = -t726;
t745 = (t9.*t10.*t647)./2.0;
t746 = -t736;
t755 = t12.*t35.*t592.*(3.9e+1./5.0e+2);
t759 = t10.*t675.*(3.0./5.0e+1);
t764 = t7.*(t555-t37.*t38.*(2.0./5.0));
t765 = t6.*t11.*(t71-t445).*(-3.0e-5);
t766 = t13.*(t555-t37.*t38.*(2.0./5.0));
t776 = t10.*t686.*(3.0./5.0e+1);
t777 = t10.*t676.*(7.0./1.0e+2);
t778 = t159+t634;
t781 = t6.*t11.*(t71-t445).*3.0e-5;
t788 = -t772;
t792 = t4.*t688.*(7.0./1.0e+2);
t801 = t399.*t593;
t802 = t399.*t594;
t803 = t502.*t548;
t811 = t482.*t563;
t813 = t143+t675;
t815 = -t774;
t826 = -t812;
t829 = t10.*t89.*t688;
t842 = t401.*t622;
t843 = t402.*t622;
t854 = t288.*t647;
t869 = t9.*t10.*t688.*(-7.0./1.0e+2);
t872 = t5.*t712.*(3.1e+1./2.5e+2);
t879 = t11.*t715.*(3.1e+1./2.5e+2);
t883 = t36.*t39.*t640.*(3.9e+1./5.0e+2);
t895 = (t397.*t600)./2.0;
t919 = t79+t217+t239+t306;
t920 = t98+t150+t170+t378;
t924 = t5.*t102.*t712;
t933 = t11.*t104.*t712;
t939 = t5.*t10.*(t163-t557).*(3.1e+1./2.5e+2);
t946 = -t909;
t953 = t4.*t5.*t712.*(-3.1e+1./2.5e+2);
t958 = t6.*t863;
t959 = t7.*t864;
t960 = t12.*t863;
t961 = t13.*t864;
t989 = t502.*t626.*2.0;
t991 = (t10.*t814)./2.0;
t993 = q_dot2.*t904;
t994 = q_dot6.*t904;
t995 = q_dot7.*t904;
t998 = t5.*t10.*(t555-t37.*t38.*(2.0./5.0)).*(1.17e+2./2.0e+2);
t999 = (t12.*t399.*t622)./2.0;
t1018 = -t986;
t1021 = t9.*t37.*t814;
t1030 = (t4.*t825)./2.0;
t1034 = q_dot2.*t940;
t1035 = q_dot3.*t940;
t1036 = q_dot7.*t940;
t1037 = (t478.*t622)./2.0;
t1038 = (t292.*t671)./2.0;
t1051 = t11.*t784.*(3.1e+1./2.5e+2);
t1052 = t4.*t823.*(3.0./5.0e+1);
t1055 = (t4.*t9.*t814)./2.0;
t1071 = t502.*t675;
t1072 = t481.*t688;
t1077 = t3.*t10.*t814.*(-1.0./2.0);
t1083 = t437.*2.170133333335e-2;
t1102 = t5.*t864.*(3.9e+1./2.0e+2);
t1108 = t438.*1.302083333335e-3;
t1109 = t439.*1.302083333335e-3;
t1110 = t443.*1.302083333335e-3;
t1111 = t444.*1.302083333335e-3;
t1112 = t445.*1.302083333335e-3;
t1133 = t7.*t1088;
t1134 = t440.*3.333333333335e-5;
t1135 = t441.*3.333333333335e-5;
t1136 = t442.*3.333333333335e-5;
t1137 = t13.*t1088;
t1139 = t446.*3.333333333335e-5;
t1140 = t447.*3.333333333335e-5;
c_num = ft_2({q_dot1,q_dot2,q_dot3,q_dot4,q_dot5,q_dot6,q_dot7,t10,t1004,t1007,t1008,t1009,t1011,t1014,t1016,t1018,t1019,t1021,t1030,t1034,t1035,t1036,t1037,t1038,t104,t1041,t1042,t1048,t1049,t1051,t1052,t1053,t1055,t1062,t1064,t1065,t1068,t1071,t1072,t1077,t1080,t1083,t1088,t1089,t1092,t1094,t1099,t11,t110,t1101,t1102,t1106,t1108,t1109,t111,t1110,t1111,t1112,t1113,t1114,t1118,t1125,t1128,t1129,t113,t1131,t1132,t1133,t1134,t1135,t1136,t1137,t1138,t1139,t1140,t1145,t1148,t1149,t1150,t1160,t1165,t1166,t1167,t1168,t1169,t1176,t1181,t1182,t1185,t1188,t1192,t1197,t12,t120,t1201,t1205,t1206,t1207,t1208,t1209,t1212,t1213,t1217,t1230,t1231,t1233,t1236,t1238,t1240,t1241,t1242,t1248,t1261,t1263,t1266,t1267,t1268,t1270,t1271,t1273,t1279,t1280,t1285,t1286,t1288,t1289,t1290,t1292,t1298,t13,t1305,t1306,t1307,t1308,t1311,t1313,t1314,t1315,t1320,t1323,t1324,t1328,t133,t1331,t1336,t1342,t1343,t1352,t1355,t1356,t1357,t1358,t1364,t1370,t1377,t1378,t1398,t140,t1403,t1409,t1414,t1423,t1441,t1463,t147,t1490,t1502,t151,t154,t157,t160,t161,t163,t164,t1671,t1673,t1677,t1678,t168,t169,t1693,t1694,t1695,t1696,t17,t1719,t172,t1735,t1736,t1741,t175,t176,t1828,t187,t196,t198,t199,t2,t200,t2005,t208,t216,t22,t225,t226,t227,t228,t23,t2348,t2349,t244,t245,t246,t248,t251,t253,t255,t256,t2571,t2572,t2577,t26,t261,t262,t264,t2655,t268,t27,t271,t272,t273,t274,t276,t28,t288,t289,t29,t290,t291,t292,t293,t294,t295,t296,t297,t298,t299,t3,t30,t300,t301,t304,t305,t307,t31,t311,t313,t314,t32,t323,t325,t33,t330,t332,t338,t34,t341,t344,t346,t349,t35,t351,t354,t358,t359,t36,t361,t362,t366,t367,t369,t37,t370,t377,t38,t380,t386,t388,t389,t39,t395,t396,t397,t398,t399,t4,t40,t400,t401,t402,t403,t404,t405,t406,t407,t411,t418,t419,t421,t422,t426,t43,t432,t433,t434,t435,t437,t438,t440,t441,t442,t444,t445,t446,t447,t448,t45,t450,t451,t453,t454,t459,t461,t463,t464,t466,t470,t473,t475,t476,t477,t478,t479,t480,t481,t482,t483,t484,t485,t488,t489,t490,t493,t494,t495,t496,t498,t499,t5,t500,t501,t502,t503,t504,t505,t506,t507,t508,t509,t51,t511,t512,t513,t514,t516,t517,t518,t520,t521,t522,t524,t525,t526,t527,t528,t529,t53,t530,t531,t532,t533,t534,t536,t54,t544,t545,t546,t547,t548,t549,t55,t550,t551,t553,t554,t555,t556,t557,t558,t56,t560,t561,t562,t563,t564,t565,t566,t567,t568,t569,t570,t571,t572,t573,t574,t586,t588,t589,t59,t591,t592,t593,t594,t6,t600,t601,t606,t607,t608,t609,t612,t614,t622,t623,t624,t625,t626,t627,t628,t631,t632,t633,t637,t638,t640,t641,t643,t647,t649,t65,t650,t652,t654,t655,t656,t66,t663,t664,t665,t666,t668,t669,t67,t671,t675,t676,t677,t678,t679,t680,t682,t683,t684,t686,t687,t688,t69,t696,t699,t7,t701,t702,t707,t708,t709,t71,t710,t711,t712,t715,t72,t720,t721,t722,t726,t727,t73,t730,t733,t734,t737,t745,t746,t75,t755,t759,t764,t765,t766,t771,t774,t776,t777,t778,t779,t780,t781,t784,t788,t791,t792,t796,t8,t800,t801,t802,t803,t804,t808,t809,t811,t812,t813,t814,t815,t823,t825,t826,t829,t838,t842,t843,t845,t846,t849,t854,t858,t861,t862,t863,t864,t866,t868,t869,t870,t871,t872,t875,t876,t877,t878,t879,t880,t881,t882,t883,t888,t889,t891,t892,t893,t894,t895,t896,t897,t9,t912,t914,t915,t916,t917,t919,t920,t921,t922,t924,t925,t926,t933,t934,t937,t938,t939,t941,t945,t946,t949,t952,t953,t954,t955,t956,t957,t958,t959,t960,t961,t962,t963,t964,t969,t972,t973,t974,t975,t976,t977,t978,t980,t981,t982,t983,t984,t988,t989,t990,t991,t993,t994,t995,t998,t999});
end
function c_num = ft_2(ct)
[q_dot1,q_dot2,q_dot3,q_dot4,q_dot5,q_dot6,q_dot7,t10,t1004,t1007,t1008,t1009,t1011,t1014,t1016,t1018,t1019,t1021,t1030,t1034,t1035,t1036,t1037,t1038,t104,t1041,t1042,t1048,t1049,t1051,t1052,t1053,t1055,t1062,t1064,t1065,t1068,t1071,t1072,t1077,t1080,t1083,t1088,t1089,t1092,t1094,t1099,t11,t110,t1101,t1102,t1106,t1108,t1109,t111,t1110,t1111,t1112,t1113,t1114,t1118,t1125,t1128,t1129,t113,t1131,t1132,t1133,t1134,t1135,t1136,t1137,t1138,t1139,t1140,t1145,t1148,t1149,t1150,t1160,t1165,t1166,t1167,t1168,t1169,t1176,t1181,t1182,t1185,t1188,t1192,t1197,t12,t120,t1201,t1205,t1206,t1207,t1208,t1209,t1212,t1213,t1217,t1230,t1231,t1233,t1236,t1238,t1240,t1241,t1242,t1248,t1261,t1263,t1266,t1267,t1268,t1270,t1271,t1273,t1279,t1280,t1285,t1286,t1288,t1289,t1290,t1292,t1298,t13,t1305,t1306,t1307,t1308,t1311,t1313,t1314,t1315,t1320,t1323,t1324,t1328,t133,t1331,t1336,t1342,t1343,t1352,t1355,t1356,t1357,t1358,t1364,t1370,t1377,t1378,t1398,t140,t1403,t1409,t1414,t1423,t1441,t1463,t147,t1490,t1502,t151,t154,t157,t160,t161,t163,t164,t1671,t1673,t1677,t1678,t168,t169,t1693,t1694,t1695,t1696,t17,t1719,t172,t1735,t1736,t1741,t175,t176,t1828,t187,t196,t198,t199,t2,t200,t2005,t208,t216,t22,t225,t226,t227,t228,t23,t2348,t2349,t244,t245,t246,t248,t251,t253,t255,t256,t2571,t2572,t2577,t26,t261,t262,t264,t2655,t268,t27,t271,t272,t273,t274,t276,t28,t288,t289,t29,t290,t291,t292,t293,t294,t295,t296,t297,t298,t299,t3,t30,t300,t301,t304,t305,t307,t31,t311,t313,t314,t32,t323,t325,t33,t330,t332,t338,t34,t341,t344,t346,t349,t35,t351,t354,t358,t359,t36,t361,t362,t366,t367,t369,t37,t370,t377,t38,t380,t386,t388,t389,t39,t395,t396,t397,t398,t399,t4,t40,t400,t401,t402,t403,t404,t405,t406,t407,t411,t418,t419,t421,t422,t426,t43,t432,t433,t434,t435,t437,t438,t440,t441,t442,t444,t445,t446,t447,t448,t45,t450,t451,t453,t454,t459,t461,t463,t464,t466,t470,t473,t475,t476,t477,t478,t479,t480,t481,t482,t483,t484,t485,t488,t489,t490,t493,t494,t495,t496,t498,t499,t5,t500,t501,t502,t503,t504,t505,t506,t507,t508,t509,t51,t511,t512,t513,t514,t516,t517,t518,t520,t521,t522,t524,t525,t526,t527,t528,t529,t53,t530,t531,t532,t533,t534,t536,t54,t544,t545,t546,t547,t548,t549,t55,t550,t551,t553,t554,t555,t556,t557,t558,t56,t560,t561,t562,t563,t564,t565,t566,t567,t568,t569,t570,t571,t572,t573,t574,t586,t588,t589,t59,t591,t592,t593,t594,t6,t600,t601,t606,t607,t608,t609,t612,t614,t622,t623,t624,t625,t626,t627,t628,t631,t632,t633,t637,t638,t640,t641,t643,t647,t649,t65,t650,t652,t654,t655,t656,t66,t663,t664,t665,t666,t668,t669,t67,t671,t675,t676,t677,t678,t679,t680,t682,t683,t684,t686,t687,t688,t69,t696,t699,t7,t701,t702,t707,t708,t709,t71,t710,t711,t712,t715,t72,t720,t721,t722,t726,t727,t73,t730,t733,t734,t737,t745,t746,t75,t755,t759,t764,t765,t766,t771,t774,t776,t777,t778,t779,t780,t781,t784,t788,t791,t792,t796,t8,t800,t801,t802,t803,t804,t808,t809,t811,t812,t813,t814,t815,t823,t825,t826,t829,t838,t842,t843,t845,t846,t849,t854,t858,t861,t862,t863,t864,t866,t868,t869,t870,t871,t872,t875,t876,t877,t878,t879,t880,t881,t882,t883,t888,t889,t891,t892,t893,t894,t895,t896,t897,t9,t912,t914,t915,t916,t917,t919,t920,t921,t922,t924,t925,t926,t933,t934,t937,t938,t939,t941,t945,t946,t949,t952,t953,t954,t955,t956,t957,t958,t959,t960,t961,t962,t963,t964,t969,t972,t973,t974,t975,t976,t977,t978,t980,t981,t982,t983,t984,t988,t989,t990,t991,t993,t994,t995,t998,t999] = ct{:};
t1141 = t448.*3.333333333335e-5;
t1144 = -t1118;
t1147 = t11.*t400.*1.0850666666675e-2;
t1153 = q_dot1.*t1106;
t1155 = q_dot5.*t1106;
t1157 = q_dot7.*t1106;
t1184 = -t1138;
t1186 = t545.*t688.*2.0;
t1189 = t4.*t5.*t864.*(1.17e+2./2.0e+2);
t1191 = t226+t863;
t1195 = t10.*t11.*t864.*(1.17e+2./2.0e+2);
t1215 = t612.*t626.*2.0;
t1218 = t3.*t4.*t397.*7.666666666675001e-3;
t1219 = t500.*3.333333333335e-5;
t1223 = t501.*3.333333333335e-5;
t1225 = -t1182;
t1229 = -t12.*(t176+t314+t459+t26.*t30.*(2.0./5.0));
t1232 = t288.*t825;
t1237 = -t1185;
t1250 = -t1201;
t1253 = t534.*1.302083333335e-3;
t1254 = t536.*1.302083333335e-3;
t1265 = t9.*t10.*t397.*2.733999999999999e-3;
t1281 = t563.*t688.*2.0;
t1282 = t397.*t814;
t1283 = t398.*t814;
t1309 = t5.*t17.*t864.*(-3.9e+1./2.0e+2);
t1312 = t5.*t23.*t864.*(1.17e+2./5.0e+2);
t1316 = t9.*t30.*t397.*1.533333333335e-2;
t1322 = t11.*t17.*t399.*1.302083333335e-3;
t1326 = t551.*t712.*2.0;
t1330 = -t1289;
t1340 = t11.*t401.*t809;
t1341 = t10.*t11.*t17.*t864.*(3.9e+1./2.0e+2);
t1360 = -t1328;
t1362 = t4.*t397.*5.283999999999999e-3;
t1369 = t4.*t398.*1.2950666666675e-2;
t1375 = t10.*t11.*t23.*t864.*(1.17e+2./5.0e+2);
t1381 = t12.*t403.*t875;
t1382 = -t1355;
t1390 = t671.*(t71-t445);
t1400 = t11.*t1088.*(1.17e+2./2.0e+2);
t1404 = t11.*t399.*9.4496250000075e-3;
t1407 = t626.*t699;
t1416 = t4.*t11.*t399.*1.4010416666675e-3;
t1421 = -t1409;
t1422 = (t638.*t640)./5.0;
t1424 = t10.*t38.*t399.*2.802083333335e-3;
t1425 = t5.*t10.*t399.*9.4496250000075e-3;
t1429 = (t640.*t654)./5.0;
t1432 = -t1423;
t1437 = t5.*t525.*1.4010416666675e-3;
t1449 = t676.*t688.*2.0;
t1455 = t547.*t864;
t1457 = t12.*(t65-t437).*(-1.302083333335e-3);
t1469 = t176+t245+t271+t314+t459;
t1470 = t11.*(t65-t437).*1.0850666666675e-2;
t1479 = t426+t453+t454+t520;
t1480 = t11.*t23.*t399.*1.362083333335e-3;
t1481 = -t1463;
t1493 = t5.*t10.*(t65-t437).*(-1.0850666666675e-2);
t1507 = t574.*t864.*3.0;
t1512 = -t712.*(t163-t557);
t1526 = t6.*t399.*t401.*6.510416666674999e-4;
t1529 = t712.*t715.*2.0;
t1547 = t712.*(t163-t557);
t1559 = t2.*t9.*t1490;
t1560 = t3.*t8.*t1490;
t1569 = -t7.*(t256+t6.*(t176+t314+t459+t26.*t30.*(2.0./5.0)));
t1571 = t11.*t288.*t399.*1.4010416666675e-3;
t1572 = t8.*t9.*t1502;
t1576 = (t9.*t1490)./2.0;
t1591 = t712.*t784;
t1600 = t13.*(t256+t6.*(t176+t314+t459+t26.*t30.*(2.0./5.0)));
t1601 = t12.*t292.*t399.*6.810416666674999e-4;
t1603 = t5.*t12.*(t71-t445).*(-6.810416666674999e-4);
t1649 = t7.*t294.*(t71-t445).*(-1.6666666666675e-5);
t1653 = t7.*t294.*(t71-t445).*1.6666666666675e-5;
t1655 = t11.*t12.*(t111-t536).*(-6.810416666674999e-4);
t1663 = t13.*t403.*(t71-t445).*(-1.6666666666675e-5);
t1665 = t5.*t6.*(t256+t6.*(t176+t314+t459+t26.*t30.*(2.0./5.0))).*(3.9e+1./2.0e+2);
t1674 = t13.*t403.*(t71-t445).*1.6666666666675e-5;
t1675 = t367+t463+t485+t490+t504;
t1676 = t369+t470+t484+t489+t503;
t1680 = t864.*(t555-t37.*t38.*(2.0./5.0)).*(3.0./2.0);
t1685 = t796+t878;
t1686 = t800+t871;
t1687 = t779+t882;
t1688 = t780+t881;
t1689 = t791+t866;
t1709 = t804+t892;
t1710 = t808+t889;
t1711 = t809+t888;
t1730 = (t5.*t1671)./2.0;
t1733 = (t10.*t1673)./2.0;
t1739 = (t10.*t1677)./2.0;
t1740 = (t10.*t1678)./2.0;
t1742 = t10.*t32.*t1671;
t1748 = t9.*t37.*t1673;
t1760 = t870+t957;
t1761 = t875+t952;
t1764 = t846+t945;
t1765 = t858+t941;
t1770 = (t10.*t11.*t1671)./2.0;
t1771 = (t5.*t1693)./2.0;
t1772 = (t5.*t1694)./2.0;
t1776 = (t4.*t9.*t1673)./2.0;
t1788 = (t4.*t9.*t1677)./2.0;
t1793 = t4.*t5.*t1671.*(-1.0./2.0);
t1794 = t11.*t39.*t1695;
t1804 = t3.*t10.*t1673.*(-1.0./2.0);
t1819 = (t11.*t1719)./2.0;
t1822 = (t10.*t11.*t1693)./2.0;
t1842 = t926+t1019;
t1854 = t12.*t36.*t1735;
t1878 = t864.*t1088.*(3.0./2.0);
t1882 = t397.*t1673;
t1883 = t398.*t1673;
t1887 = t397.*t1677;
t1888 = t397.*t1678;
t1893 = t399.*t1671;
t1894 = t400.*t1671;
t1911 = t399.*t1693;
t1912 = t399.*t1694;
t1913 = t402.*t1695;
t1914 = t401.*t1696;
t1933 = t5.*t288.*t1671.*(-1.0./2.0);
t1943 = (t477.*t1671)./2.0;
t1944 = (t290.*t1719)./2.0;
t1951 = t403.*t1736;
t1952 = t404.*t1735;
t1963 = (t478.*t1695)./2.0;
t1964 = (t292.*t1741)./2.0;
t1967 = (t12.*t399.*t1695)./2.0;
t2021 = -t2005;
t2078 = t1741.*(t71-t445);
t2101 = t7.*t1735.*(t71-t445).*(-1.0./2.0);
t2109 = (t7.*t1735.*(t71-t445))./2.0;
t2359 = q_dot4.*t2349;
t2575 = q_dot3.*t2572;
t2582 = t917+t1129+t1213+t1288;
t2657 = t915+t978+t1148+t1169+t1176+t1263+t1311;
t2658 = t915+t978+t1128+t1192+t1212+t1267+t1308;
t2661 = t434+t1089+t1114+t1188+t1236+t1290+t1292+t1331;
t2667 = t976+t981+t1064+t1145+t1238+t1266+t1273+t1307+t1315+t1336+t1370;
t2668 = t1011+t1016+t1042+t1145+t1238+t1266+t1273+t1307+t1315+t1336+t1370;
t535 = t6.*t509;
t538 = t6.*t517;
t577 = t505.*(3.9e+1./1.0e+2);
t578 = t505.*(3.1e+1./2.5e+2);
t579 = t505.*1.5e-3;
t582 = t512.*(3.9e+1./1.0e+2);
t583 = t512.*(3.1e+1./2.5e+2);
t584 = t512.*1.5e-3;
t595 = t499.*6.0e-5;
t596 = t506.*6.0e-5;
t597 = t507.*6.0e-5;
t599 = t516.*6.0e-5;
t603 = t43+t505;
t605 = t45+t511;
t616 = t56+t516;
t618 = t7.*t588;
t619 = t13.*t588;
t620 = t7.*t573;
t621 = t13.*t573;
t657 = q_dot3.*t632;
t658 = q_dot3.*t633;
t659 = q_dot4.*t633;
t660 = q_dot6.*t632;
t661 = q_dot7.*t632;
t662 = q_dot7.*t633;
t670 = -t7.*(t69-t508);
t672 = -t7.*(t67-t512);
t689 = -t677;
t690 = -t678;
t691 = -t679;
t692 = (t11.*t609)./2.0;
t694 = t120+t550;
t700 = t10.*t38.*t609;
t703 = t8.*t9.*t631;
t705 = t7.*t664;
t706 = t13.*t664;
t714 = (t5.*t10.*t609)./2.0;
t717 = (t3.*t631)./2.0;
t723 = t6.*t13.*(t67-t512);
t725 = t11.*t608.*(3.1e+1./2.5e+2);
t732 = (t5.*t656)./2.0;
t735 = (t4.*t663)./2.0;
t739 = t325+t561;
t740 = t11.*t12.*t573.*3.0e-5;
t741 = t498+t513;
t743 = t5.*t104.*t608;
t748 = t349+t567;
t749 = t6.*t727;
t750 = t12.*t727;
t758 = (t9.*t10.*t663)./2.0;
t760 = -t745;
t767 = t12.*t28.*t607.*(3.9e+1./5.0e+2);
t768 = -t755;
t775 = -t759;
t782 = t290.*t609;
t783 = t291.*t609;
t816 = -t792;
t817 = t7.*t778;
t818 = t13.*t778;
t821 = t292.*t632;
t822 = t292.*t633;
t853 = -t803;
t865 = -t811;
t885 = t288.*t663;
t899 = -t879;
t905 = t39.*t40.*t655.*(3.9e+1./5.0e+2);
t967 = t5.*t12.*(t386-t572).*(-1.0./2.0);
t968 = t6.*t11.*(t386-t572).*(-1.0./2.0);
t996 = t161+t380+t558;
t1002 = (t6.*t11.*(t386-t572))./2.0;
t1005 = t507+t643;
t1017 = t6.*t959;
t1020 = t6.*t961;
t1022 = t6.*t920;
t1023 = t7.*t919;
t1024 = t7.*t920;
t1026 = t12.*t920;
t1027 = t13.*t919;
t1028 = t13.*t920;
t1031 = -t989;
t1032 = t10.*t813.*(3.0./5.0e+1);
t1033 = -t991;
t1039 = -t998;
t1054 = t3.*t991;
t1056 = -t1030;
t1058 = -t993;
t1059 = -t995;
t1060 = (t525.*t609)./2.0;
t1061 = (t399.*t656)./2.0;
t1074 = -t1021;
t1075 = -t1052;
t1093 = -t1071;
t1096 = t529.*t687;
t1097 = t530.*t687;
t1100 = -t1072;
t1104 = t11.*t34.*t778.*(3.9e+1./2.0e+2);
t1105 = t466+t488+t521;
t1119 = t505.*2.170133333335e-2;
t1120 = -t13.*(t514+t6.*(t65-t437));
t1122 = t512.*2.170133333335e-2;
t1124 = t11.*t12.*(t464-t623).*(-1.0./2.0);
t1127 = -t1111;
t1158 = t498.*1.302083333335e-3;
t1159 = t499.*1.302083333335e-3;
t1161 = t505.*1.302083333335e-3;
t1162 = t506.*1.302083333335e-3;
t1163 = t507.*1.302083333335e-3;
t1164 = t508.*1.302083333335e-3;
t1172 = t512.*1.302083333335e-3;
t1173 = t513.*1.302083333335e-3;
t1174 = t514.*1.302083333335e-3;
t1175 = t516.*1.302083333335e-3;
t1179 = (t592.*t606)./5.0;
t1180 = (t591.*t607)./5.0;
t1187 = t7.*(t514+t6.*(t65-t437));
t1190 = -t1147;
t1199 = t11.*t919.*(1.17e+2./2.0e+2);
t1200 = t11.*t920.*(1.17e+2./2.0e+2);
t1202 = (t573.*t622)./2.0;
t1222 = t548.*t687.*2.0;
t1227 = t509.*3.333333333335e-5;
t1228 = t511.*3.333333333335e-5;
t1234 = t517.*3.333333333335e-5;
t1235 = t518.*3.333333333335e-5;
t1244 = -t1186;
t1246 = -t1189;
t1247 = t196+t920;
t1264 = t17.*t1102;
t1274 = -t1218;
t1275 = t133+t958;
t1276 = -t1223;
t1293 = t5.*t10.*t920.*(1.17e+2./2.0e+2);
t1302 = t593.*(t67-t512).*(-1.0./2.0);
t1303 = t594.*(t67-t512).*(-1.0./2.0);
t1310 = -t1265;
t1325 = -t1281;
t1327 = -t1232;
t1334 = t547.*t733;
t1337 = t154+t244+t313+t560;
t1344 = (t593.*(t67-t512))./2.0;
t1345 = (t594.*(t67-t512))./2.0;
t1347 = t632.*(t71-t445).*(-1.0./2.0);
t1348 = t633.*(t71-t445).*(-1.0./2.0);
t1349 = t401.*(t386-t572).*(-1.0./2.0);
t1350 = t402.*(t386-t572).*(-1.0./2.0);
t1351 = -t1312;
t1359 = -t1326;
t1361 = -t1282;
t1367 = t478.*(t386-t572);
t1373 = (t632.*(t71-t445))./2.0;
t1374 = (t401.*(t386-t572))./2.0;
t1379 = t553.*3.333333333335e-5;
t1380 = t554.*3.333333333335e-5;
t1388 = -t1362;
t1389 = t502.*t813;
t1391 = t626.*t687;
t1394 = t225+t323+t727;
t1396 = t549.*3.333333333335e-5;
t1397 = t550.*3.333333333335e-5;
t1405 = t656.*(t67-t512);
t1420 = t608.*t712.*2.0;
t1426 = -t1407;
t1427 = -t1422;
t1430 = (t641.*t655)./5.0;
t1433 = -t13.*(t246+t330-t556-t2.*t26.*(2.0./5.0));
t1445 = (t655.*(t307-t411))./5.0;
t1446 = t5.*t1191.*(3.9e+1./1.0e+2);
t1448 = t675.*t687.*2.0;
t1467 = t7.*(t246+t330-t556-t2.*t26.*(2.0./5.0));
t1471 = t686.*t687.*2.0;
t1472 = -t1449;
t1475 = t5.*t6.*t573.*6.510416666674999e-4;
t1477 = t573.*(t386-t572);
t1496 = q_dot1.*t1479;
t1497 = q_dot4.*t1479;
t1498 = q_dot7.*t1479;
t1499 = t11.*t34.*t573.*6.510416666674999e-4;
t1503 = t612.*t813;
t1511 = t7.*(t69-t508).*(-3.333333333335e-5);
t1513 = t5.*t588.*1.4010416666675e-3;
t1515 = t7.*(t67-t512).*(-3.333333333335e-5);
t1517 = t13.*(t67-t512).*(-3.333333333335e-5);
t1521 = -t1507;
t1522 = t5.*t12.*(t169-t960).*(-1.17e+2./5.0e+2);
t1524 = t622.*(t499-t506).*(-1.0./2.0);
t1528 = t6.*t11.*(t69-t508).*(-6.510416666674999e-4);
t1537 = t5.*t12.*(t169-t960).*(1.17e+2./5.0e+2);
t1538 = (t622.*(t499-t506))./2.0;
t1540 = t6.*t11.*(t69-t508).*6.510416666674999e-4;
t1541 = -t1529;
t1546 = t10.*t11.*t588.*1.4010416666675e-3;
t1549 = t11.*(t246+t330-t556-t2.*t26.*(2.0./5.0)).*(1.17e+2./2.0e+2);
t1553 = t6.*t11.*t664.*6.510416666674999e-4;
t1558 = t5.*t10.*(t246+t330-t556-t2.*t26.*(2.0./5.0)).*(-1.17e+2./2.0e+2);
t1561 = t11.*t17.*(t67-t512).*1.302083333335e-3;
t1568 = (t12.*(t67-t512).*(t386-t572))./2.0;
t1583 = -t1559;
t1590 = -t1576;
t1592 = ((t71-t445).*(t464-t623))./2.0;
t1593 = ((t111-t536).*(t386-t572))./2.0;
t1595 = t11.*(t67-t512).*9.4496250000075e-3;
t1597 = t5.*t1469.*(3.9e+1./1.0e+2);
t1599 = t687.*t813.*2.0;
t1602 = t4.*t11.*(t67-t512).*(-1.4010416666675e-3);
t1605 = -t1572;
t1613 = t699.*t813.*2.0;
t1615 = t4.*t11.*(t67-t512).*1.4010416666675e-3;
t1619 = -t1591;
t1626 = t10.*t38.*(t67-t512).*(-1.4010416666675e-3);
t1636 = t6.*t399.*t573.*1.302083333335e-3;
t1648 = t11.*t23.*(t67-t512).*1.362083333335e-3;
t1656 = t5.*t12.*(t1229+t8.*t56.*(2.0./5.0)).*(1.17e+2./5.0e+2);
t1664 = t13.*t292.*(t75-t518).*(-3.333333333335e-5);
t1669 = ((t386-t572).*(t499-t506))./2.0;
t1682 = t6.*t401.*(t67-t512).*(-6.510416666674999e-4);
t1690 = -t1680;
t1699 = q_dot1.*t1675;
t1700 = q_dot1.*t1676;
t1701 = q_dot2.*t1676;
t1702 = q_dot6.*t1675;
t1703 = q_dot7.*t1675;
t1704 = q_dot7.*t1676;
t1705 = t813.*t823.*2.0;
t1706 = t11.*t288.*(t67-t512).*(-2.802083333335e-3);
t1744 = t864.*t919.*3.0;
t1745 = t864.*t920.*3.0;
t1749 = (t11.*t1685)./2.0;
t1750 = (t11.*t1686)./2.0;
t1752 = (t4.*t1687)./2.0;
t1753 = (t4.*t1688)./2.0;
t1756 = -t1733;
t1762 = (t4.*t1689)./2.0;
t1763 = -t1739;
t1767 = t13.*(t514+t6.*(t65-t437)).*(-3.333333333335e-5);
t1775 = t3.*t1733;
t1782 = t9.*t30.*t1689;
t1792 = -t1742;
t1795 = (t5.*t10.*t1685)./2.0;
t1796 = -t1771;
t1797 = -t1772;
t1798 = -t1748;
t1800 = (t11.*t1709)./2.0;
t1806 = (t9.*t10.*t1687)./2.0;
t1808 = t6.*t573.*(t67-t512).*(-6.510416666674999e-4);
t1814 = -t1788;
t1815 = (t9.*t10.*t1689)./2.0;
t1818 = t11.*t34.*t1710;
t1820 = t10.*t38.*t1709;
t1831 = t6.*t573.*(t67-t512).*6.510416666674999e-4;
t1832 = t3.*t4.*t1689.*(-1.0./2.0);
t1833 = t6.*t11.*(t514+t6.*(t65-t437)).*6.510416666674999e-4;
t1839 = (t5.*t10.*t1709)./2.0;
t1849 = t876+t1083;
t1850 = t13.*(t71-t445).*(t75-t518).*1.6666666666675e-5;
t1851 = (t5.*t1764)./2.0;
t1855 = t845+t1110;
t1857 = t862+t1109;
t1864 = t12.*t40.*t1760;
t1866 = t894+t1112;
t1868 = t288.*t1687;
t1869 = t288.*t1688;
t1871 = t288.*t1689;
t1872 = t289.*t1689;
t1875 = -t1854;
t1879 = t290.*t1685;
t1880 = t290.*t1686;
t1892 = -t1878;
t1898 = t925+t1141;
t1901 = t290.*t1709;
t1902 = t291.*t1709;
t1903 = t293.*t1710;
t1904 = t292.*t1711;
t1905 = -t1882;
t1907 = t955+t1136;
t1916 = t12.*(t71-t445).*(t67-t512).*6.810416666674999e-4;
t1920 = t912+t1253;
t1923 = t288.*t1730;
t1931 = t946+t1254;
t1940 = t294.*t1761;
t1941 = t295.*t1760;
t1954 = -t1943;
t1955 = -t1944;
t1972 = (t6.*t399.*t1710)./2.0;
t1994 = (t525.*t1709)./2.0;
t1995 = (t399.*t1764)./2.0;
t1996 = (t526.*t1710)./2.0;
t1997 = (t401.*t1765)./2.0;
t2027 = (t573.*t1696)./2.0;
t2043 = t573.*t1765;
t2050 = t1671.*(t67-t512).*(-1.0./2.0);
t2059 = (t1671.*(t67-t512))./2.0;
t2065 = t1711.*(t71-t445).*(-1.0./2.0);
t2074 = t1693.*(t67-t512).*(-1.0./2.0);
t2075 = t1694.*(t67-t512).*(-1.0./2.0);
t2079 = (t1693.*(t67-t512))./2.0;
t2080 = (t1694.*(t67-t512))./2.0;
t2090 = t6.*t1710.*(t67-t512).*(-1.0./2.0);
t2097 = t1764.*(t67-t512);
t2110 = t13.*t1760.*(t71-t445).*(-1.0./2.0);
t2119 = (t13.*t1760.*(t71-t445))./2.0;
t2160 = t1137+t1569;
t2167 = t1695.*(t499-t506).*(-1.0./2.0);
t2176 = (t1695.*(t499-t506))./2.0;
t2181 = t1133+t1600;
t2289 = (t1710.*(t514+t6.*(t65-t437)))./2.0;
t2319 = t1760.*(t441+t13.*(t69-t508)).*(-1.0./2.0);
t2320 = t403.*(t1135+t13.*(t69-t508).*3.333333333335e-5).*(-1.0./2.0);
t2325 = (t1760.*(t441+t13.*(t69-t508)))./2.0;
t2326 = (t403.*(t1135+t13.*(t69-t508).*3.333333333335e-5))./2.0;
t2583 = -t2575;
t2597 = q_dot3.*t2582;
t2659 = q_dot2.*t2657;
t2662 = q_dot3.*t2661;
t2669 = q_dot1.*t2668;
t552 = -t535;
t598 = -t582;
t642 = t6.*t603;
t644 = t7.*t603;
t645 = t12.*t603;
t646 = t13.*t603;
t697 = t6.*t672;
t704 = -t692;
t713 = t4.*t692;
t728 = -t706;
t742 = t440+t538;
t744 = -t735;
t747 = t273+t579;
t751 = -t740;
t773 = -t758;
t790 = t7.*t741;
t793 = t13.*t741;
t798 = t370+t599;
t819 = (t5.*t739)./2.0;
t884 = (t10.*t11.*t739)./2.0;
t902 = t288.*t692;
t913 = t11.*(t344-t584).*(-1.0./2.0);
t944 = (t11.*t12.*t748)./2.0;
t948 = t517+t620;
t966 = t5.*t10.*(t344-t584).*(-1.0./2.0);
t1000 = (t4.*t11.*(t344-t584))./2.0;
t1006 = t447+t670;
t1044 = t175+t272+t578;
t1045 = t10.*t38.*(t344-t584).*(-1.0./2.0);
t1050 = t11.*(t341-t583).*(3.1e+1./2.5e+2);
t1057 = -t1032;
t1078 = -t1060;
t1079 = -t1061;
t1082 = t251+t750;
t1095 = t311+t749;
t1142 = -t1096;
t1143 = -t1097;
t1152 = q_dot1.*t1105;
t1154 = q_dot3.*t1105;
t1156 = q_dot7.*t1105;
c_num = ft_3({q_dot1,q_dot2,q_dot3,q_dot4,q_dot5,q_dot6,q_dot7,t10,t1000,t1002,t1004,t1005,t1006,t1007,t1008,t1009,t1014,t1017,t1018,t1020,t1022,t1023,t1024,t1026,t1027,t1028,t1031,t1032,t1033,t1034,t1035,t1036,t1037,t1038,t1039,t104,t1041,t1044,t1045,t1048,t1049,t1050,t1051,t1053,t1054,t1055,t1056,t1057,t1058,t1059,t1060,t1061,t1062,t1065,t1068,t1071,t1072,t1074,t1075,t1077,t1078,t1079,t1080,t1082,t1088,t1092,t1093,t1094,t1095,t1096,t1097,t1099,t11,t110,t1100,t1101,t1102,t1104,t1108,t111,t1113,t1118,t1119,t1120,t1122,t1124,t1125,t1127,t113,t1131,t1132,t1134,t1135,t1139,t1140,t1142,t1143,t1144,t1147,t1149,t1150,t1152,t1153,t1154,t1155,t1156,t1157,t1158,t1159,t1160,t1161,t1162,t1163,t1164,t1165,t1166,t1167,t1168,t1172,t1173,t1174,t1175,t1179,t1180,t1181,t1184,t1187,t1190,t1191,t1195,t1197,t1199,t12,t1200,t1201,t1202,t1205,t1206,t1207,t1208,t1209,t1215,t1217,t1218,t1219,t1222,t1225,t1227,t1228,t1229,t1230,t1231,t1233,t1234,t1235,t1237,t1240,t1241,t1242,t1244,t1246,t1247,t1248,t1250,t1261,t1264,t1265,t1268,t1270,t1271,t1274,t1275,t1276,t1279,t1280,t1283,t1285,t1286,t1289,t1293,t1298,t13,t1302,t1303,t1305,t1306,t1309,t1310,t1312,t1313,t1314,t1316,t1320,t1322,t1323,t1324,t1325,t1327,t1328,t1330,t1334,t1337,t1340,t1341,t1342,t1343,t1344,t1345,t1347,t1348,t1349,t1350,t1351,t1352,t1355,t1356,t1357,t1358,t1359,t1360,t1361,t1362,t1364,t1367,t1369,t1373,t1374,t1375,t1377,t1378,t1379,t1380,t1381,t1382,t1388,t1389,t1390,t1391,t1394,t1396,t1397,t1398,t140,t1400,t1403,t1404,t1405,t1407,t1409,t1414,t1416,t1420,t1421,t1423,t1424,t1425,t1426,t1427,t1429,t1430,t1432,t1433,t1437,t1441,t1445,t1446,t1448,t1455,t1457,t1463,t1467,t1469,t147,t1470,t1471,t1472,t1475,t1477,t1480,t1481,t1493,t1496,t1497,t1498,t1499,t1502,t1503,t151,t1511,t1512,t1513,t1515,t1517,t1521,t1522,t1524,t1526,t1528,t1537,t1538,t1540,t1541,t1546,t1547,t1549,t1553,t1558,t1560,t1561,t1568,t157,t1571,t1576,t1583,t1590,t1591,t1592,t1593,t1595,t1597,t1599,t160,t1601,t1602,t1603,t1605,t1613,t1615,t1619,t1626,t163,t1636,t164,t1648,t1649,t1653,t1655,t1656,t1663,t1664,t1665,t1669,t1671,t1674,t1678,t168,t1680,t1682,t1685,t1686,t1688,t169,t1690,t1694,t1695,t1696,t1699,t17,t1700,t1701,t1702,t1703,t1704,t1705,t1706,t1709,t1710,t1711,t1719,t172,t1730,t1733,t1735,t1736,t1739,t1740,t1741,t1744,t1745,t1749,t1750,t1752,t1753,t1756,t176,t1760,t1761,t1762,t1763,t1764,t1765,t1767,t1770,t1771,t1772,t1775,t1776,t1782,t1788,t1792,t1793,t1794,t1795,t1796,t1797,t1798,t1800,t1804,t1806,t1808,t1814,t1815,t1818,t1819,t1820,t1822,t1828,t1831,t1832,t1833,t1839,t1842,t1849,t1850,t1851,t1855,t1857,t1864,t1866,t1868,t1869,t187,t1871,t1872,t1875,t1878,t1879,t1880,t1883,t1887,t1888,t1892,t1893,t1894,t1898,t1901,t1902,t1903,t1904,t1905,t1907,t1911,t1912,t1913,t1914,t1916,t1920,t1923,t1931,t1933,t1940,t1941,t1943,t1944,t1951,t1952,t1954,t1955,t1963,t1964,t1967,t1972,t198,t199,t1994,t1995,t1996,t1997,t2,t200,t2005,t2021,t2027,t2043,t2050,t2059,t2065,t2074,t2075,t2078,t2079,t208,t2080,t2090,t2097,t2101,t2109,t2110,t2119,t216,t2160,t2167,t2176,t2181,t22,t227,t228,t2289,t23,t2319,t2320,t2325,t2326,t2348,t2349,t2359,t246,t248,t253,t255,t256,t2571,t2572,t2577,t2582,t2583,t2597,t26,t261,t262,t264,t2655,t2657,t2658,t2659,t2661,t2662,t2667,t2668,t2669,t268,t27,t274,t276,t28,t288,t289,t29,t290,t291,t292,t293,t294,t295,t296,t297,t298,t299,t3,t30,t300,t301,t304,t305,t307,t31,t314,t32,t33,t330,t332,t338,t34,t341,t344,t346,t35,t351,t354,t358,t359,t36,t361,t362,t366,t37,t377,t38,t386,t388,t389,t39,t395,t396,t398,t399,t4,t40,t400,t401,t402,t403,t404,t405,t406,t407,t411,t418,t419,t421,t422,t43,t432,t433,t435,t437,t438,t441,t442,t444,t445,t446,t450,t451,t459,t461,t464,t473,t475,t476,t477,t478,t479,t480,t481,t482,t483,t493,t494,t495,t496,t499,t5,t500,t501,t502,t506,t508,t509,t51,t512,t514,t518,t522,t524,t525,t526,t527,t528,t53,t530,t531,t532,t533,t535,t536,t538,t54,t544,t545,t546,t547,t548,t549,t55,t551,t552,t553,t554,t555,t556,t557,t56,t562,t564,t565,t566,t568,t569,t570,t571,t572,t573,t574,t577,t582,t583,t584,t586,t588,t589,t59,t591,t592,t594,t595,t596,t597,t598,t6,t600,t601,t603,t605,t606,t607,t608,t609,t612,t614,t616,t618,t619,t620,t621,t622,t623,t624,t625,t626,t627,t628,t632,t633,t637,t638,t640,t641,t642,t644,t645,t646,t647,t649,t65,t650,t652,t654,t655,t656,t657,t658,t659,t66,t660,t661,t662,t664,t665,t666,t668,t669,t67,t671,t676,t677,t678,t679,t680,t682,t683,t684,t686,t689,t69,t690,t691,t692,t694,t696,t697,t699,t7,t700,t701,t702,t703,t704,t705,t706,t707,t708,t709,t71,t710,t711,t712,t713,t714,t715,t717,t72,t720,t721,t722,t723,t725,t726,t728,t73,t730,t732,t733,t734,t735,t737,t739,t740,t741,t742,t743,t744,t745,t746,t747,t748,t75,t751,t758,t759,t760,t764,t765,t766,t767,t768,t771,t773,t774,t775,t776,t777,t778,t781,t782,t783,t784,t788,t790,t792,t793,t798,t8,t801,t802,t803,t811,t812,t815,t816,t817,t818,t819,t821,t822,t823,t825,t826,t829,t838,t842,t843,t849,t853,t854,t861,t864,t865,t868,t869,t872,t877,t879,t880,t883,t884,t885,t891,t893,t895,t896,t897,t899,t9,t902,t905,t913,t914,t916,t919,t920,t921,t922,t924,t933,t934,t937,t938,t939,t944,t948,t949,t953,t954,t956,t959,t960,t961,t962,t963,t964,t966,t967,t968,t969,t972,t973,t974,t975,t977,t980,t982,t983,t984,t988,t990,t991,t994,t995,t996,t998,t999});
end
function c_num = ft_3(ct)
[q_dot1,q_dot2,q_dot3,q_dot4,q_dot5,q_dot6,q_dot7,t10,t1000,t1002,t1004,t1005,t1006,t1007,t1008,t1009,t1014,t1017,t1018,t1020,t1022,t1023,t1024,t1026,t1027,t1028,t1031,t1032,t1033,t1034,t1035,t1036,t1037,t1038,t1039,t104,t1041,t1044,t1045,t1048,t1049,t1050,t1051,t1053,t1054,t1055,t1056,t1057,t1058,t1059,t1060,t1061,t1062,t1065,t1068,t1071,t1072,t1074,t1075,t1077,t1078,t1079,t1080,t1082,t1088,t1092,t1093,t1094,t1095,t1096,t1097,t1099,t11,t110,t1100,t1101,t1102,t1104,t1108,t111,t1113,t1118,t1119,t1120,t1122,t1124,t1125,t1127,t113,t1131,t1132,t1134,t1135,t1139,t1140,t1142,t1143,t1144,t1147,t1149,t1150,t1152,t1153,t1154,t1155,t1156,t1157,t1158,t1159,t1160,t1161,t1162,t1163,t1164,t1165,t1166,t1167,t1168,t1172,t1173,t1174,t1175,t1179,t1180,t1181,t1184,t1187,t1190,t1191,t1195,t1197,t1199,t12,t1200,t1201,t1202,t1205,t1206,t1207,t1208,t1209,t1215,t1217,t1218,t1219,t1222,t1225,t1227,t1228,t1229,t1230,t1231,t1233,t1234,t1235,t1237,t1240,t1241,t1242,t1244,t1246,t1247,t1248,t1250,t1261,t1264,t1265,t1268,t1270,t1271,t1274,t1275,t1276,t1279,t1280,t1283,t1285,t1286,t1289,t1293,t1298,t13,t1302,t1303,t1305,t1306,t1309,t1310,t1312,t1313,t1314,t1316,t1320,t1322,t1323,t1324,t1325,t1327,t1328,t1330,t1334,t1337,t1340,t1341,t1342,t1343,t1344,t1345,t1347,t1348,t1349,t1350,t1351,t1352,t1355,t1356,t1357,t1358,t1359,t1360,t1361,t1362,t1364,t1367,t1369,t1373,t1374,t1375,t1377,t1378,t1379,t1380,t1381,t1382,t1388,t1389,t1390,t1391,t1394,t1396,t1397,t1398,t140,t1400,t1403,t1404,t1405,t1407,t1409,t1414,t1416,t1420,t1421,t1423,t1424,t1425,t1426,t1427,t1429,t1430,t1432,t1433,t1437,t1441,t1445,t1446,t1448,t1455,t1457,t1463,t1467,t1469,t147,t1470,t1471,t1472,t1475,t1477,t1480,t1481,t1493,t1496,t1497,t1498,t1499,t1502,t1503,t151,t1511,t1512,t1513,t1515,t1517,t1521,t1522,t1524,t1526,t1528,t1537,t1538,t1540,t1541,t1546,t1547,t1549,t1553,t1558,t1560,t1561,t1568,t157,t1571,t1576,t1583,t1590,t1591,t1592,t1593,t1595,t1597,t1599,t160,t1601,t1602,t1603,t1605,t1613,t1615,t1619,t1626,t163,t1636,t164,t1648,t1649,t1653,t1655,t1656,t1663,t1664,t1665,t1669,t1671,t1674,t1678,t168,t1680,t1682,t1685,t1686,t1688,t169,t1690,t1694,t1695,t1696,t1699,t17,t1700,t1701,t1702,t1703,t1704,t1705,t1706,t1709,t1710,t1711,t1719,t172,t1730,t1733,t1735,t1736,t1739,t1740,t1741,t1744,t1745,t1749,t1750,t1752,t1753,t1756,t176,t1760,t1761,t1762,t1763,t1764,t1765,t1767,t1770,t1771,t1772,t1775,t1776,t1782,t1788,t1792,t1793,t1794,t1795,t1796,t1797,t1798,t1800,t1804,t1806,t1808,t1814,t1815,t1818,t1819,t1820,t1822,t1828,t1831,t1832,t1833,t1839,t1842,t1849,t1850,t1851,t1855,t1857,t1864,t1866,t1868,t1869,t187,t1871,t1872,t1875,t1878,t1879,t1880,t1883,t1887,t1888,t1892,t1893,t1894,t1898,t1901,t1902,t1903,t1904,t1905,t1907,t1911,t1912,t1913,t1914,t1916,t1920,t1923,t1931,t1933,t1940,t1941,t1943,t1944,t1951,t1952,t1954,t1955,t1963,t1964,t1967,t1972,t198,t199,t1994,t1995,t1996,t1997,t2,t200,t2005,t2021,t2027,t2043,t2050,t2059,t2065,t2074,t2075,t2078,t2079,t208,t2080,t2090,t2097,t2101,t2109,t2110,t2119,t216,t2160,t2167,t2176,t2181,t22,t227,t228,t2289,t23,t2319,t2320,t2325,t2326,t2348,t2349,t2359,t246,t248,t253,t255,t256,t2571,t2572,t2577,t2582,t2583,t2597,t26,t261,t262,t264,t2655,t2657,t2658,t2659,t2661,t2662,t2667,t2668,t2669,t268,t27,t274,t276,t28,t288,t289,t29,t290,t291,t292,t293,t294,t295,t296,t297,t298,t299,t3,t30,t300,t301,t304,t305,t307,t31,t314,t32,t33,t330,t332,t338,t34,t341,t344,t346,t35,t351,t354,t358,t359,t36,t361,t362,t366,t37,t377,t38,t386,t388,t389,t39,t395,t396,t398,t399,t4,t40,t400,t401,t402,t403,t404,t405,t406,t407,t411,t418,t419,t421,t422,t43,t432,t433,t435,t437,t438,t441,t442,t444,t445,t446,t450,t451,t459,t461,t464,t473,t475,t476,t477,t478,t479,t480,t481,t482,t483,t493,t494,t495,t496,t499,t5,t500,t501,t502,t506,t508,t509,t51,t512,t514,t518,t522,t524,t525,t526,t527,t528,t53,t530,t531,t532,t533,t535,t536,t538,t54,t544,t545,t546,t547,t548,t549,t55,t551,t552,t553,t554,t555,t556,t557,t56,t562,t564,t565,t566,t568,t569,t570,t571,t572,t573,t574,t577,t582,t583,t584,t586,t588,t589,t59,t591,t592,t594,t595,t596,t597,t598,t6,t600,t601,t603,t605,t606,t607,t608,t609,t612,t614,t616,t618,t619,t620,t621,t622,t623,t624,t625,t626,t627,t628,t632,t633,t637,t638,t640,t641,t642,t644,t645,t646,t647,t649,t65,t650,t652,t654,t655,t656,t657,t658,t659,t66,t660,t661,t662,t664,t665,t666,t668,t669,t67,t671,t676,t677,t678,t679,t680,t682,t683,t684,t686,t689,t69,t690,t691,t692,t694,t696,t697,t699,t7,t700,t701,t702,t703,t704,t705,t706,t707,t708,t709,t71,t710,t711,t712,t713,t714,t715,t717,t72,t720,t721,t722,t723,t725,t726,t728,t73,t730,t732,t733,t734,t735,t737,t739,t740,t741,t742,t743,t744,t745,t746,t747,t748,t75,t751,t758,t759,t760,t764,t765,t766,t767,t768,t771,t773,t774,t775,t776,t777,t778,t781,t782,t783,t784,t788,t790,t792,t793,t798,t8,t801,t802,t803,t811,t812,t815,t816,t817,t818,t819,t821,t822,t823,t825,t826,t829,t838,t842,t843,t849,t853,t854,t861,t864,t865,t868,t869,t872,t877,t879,t880,t883,t884,t885,t891,t893,t895,t896,t897,t899,t9,t902,t905,t913,t914,t916,t919,t920,t921,t922,t924,t933,t934,t937,t938,t939,t944,t948,t949,t953,t954,t956,t959,t960,t961,t962,t963,t964,t966,t967,t968,t969,t972,t973,t974,t975,t977,t980,t982,t983,t984,t988,t990,t991,t994,t995,t996,t998,t999] = ct{:};
t1198 = -t11.*t288.*(t344-t584);
t1203 = (t292.*t748)./2.0;
t1220 = -t1179;
t1221 = -t1180;
t1226 = t11.*t996.*(3.1e+1./2.5e+2);
t1249 = -t1199;
t1252 = t553+t705;
t1255 = (t603.*t609)./2.0;
t1256 = t290.*(t344-t584).*(-1.0./2.0);
t1257 = t291.*(t344-t584).*(-1.0./2.0);
t1258 = -t1202;
t1278 = -t1227;
t1300 = (t290.*(t344-t584))./2.0;
t1301 = (t291.*(t344-t584))./2.0;
t1318 = t5.*t104.*t996;
t1319 = t535.*3.333333333335e-5;
t1321 = t538.*3.333333333335e-5;
t1376 = t168+t1022;
t1385 = t7.*t1275;
t1387 = t13.*t1275;
t1406 = t525.*(t344-t584);
t1411 = t208+t253+t268+t577;
t1413 = t6.*t1337;
t1415 = t12.*t1337;
t1418 = t597+t730;
t1442 = -t588.*(t344-t584);
t1450 = -t739.*(t67-t512);
t1458 = -t1445;
t1461 = -t1446;
t1462 = t618.*3.333333333335e-5;
t1464 = t619.*3.333333333335e-5;
t1465 = t620.*3.333333333335e-5;
t1466 = t11.*t1247.*(3.9e+1./1.0e+2);
t1468 = t621.*3.333333333335e-5;
t1473 = -t616.*(t386-t572);
t1476 = -t603.*(t344-t584);
t1487 = t748.*(t71-t445);
t1489 = t5.*t10.*t1247.*(3.9e+1./1.0e+2);
t1492 = t4.*t5.*t603.*1.0850666666675e-2;
t1495 = t5.*t6.*t1275.*(3.9e+1./2.0e+2);
t1508 = t292.*(t595-t596).*(-1.0./2.0);
t1514 = t10.*t32.*t603.*1.0850666666675e-2;
t1519 = t625+t817;
t1523 = (t292.*(t595-t596))./2.0;
t1531 = -t1503;
t1542 = t705.*3.333333333335e-5;
t1543 = t706.*3.333333333335e-5;
t1544 = t6.*t1515;
t1550 = t5.*t6.*(t160-t1026).*(-3.9e+1./1.0e+3);
t1554 = t5.*t603.*9.4496250000075e-3;
t1555 = t11.*t12.*(t160-t1026).*(-1.17e+2./5.0e+2);
t1557 = t723.*3.333333333335e-5;
t1565 = t5.*t6.*(t160-t1026).*(3.9e+1./1.0e+3);
t1567 = t11.*t12.*(t160-t1026).*(1.17e+2./5.0e+2);
t1578 = t10.*t11.*t603.*9.4496250000075e-3;
t1582 = -t1568;
t1585 = -t712.*(t341-t583);
t1587 = t11.*t33.*(t160-t1026).*(-1.17e+2./5.0e+2);
t1589 = t11.*t34.*(t160-t1026).*(-3.9e+1./1.0e+3);
t1604 = t11.*t12.*t616.*6.810416666674999e-4;
t1606 = t11.*t34.*(t160-t1026).*(3.9e+1./1.0e+3);
t1608 = -t1592;
t1609 = -t1593;
t1612 = -t1599;
t1618 = t712.*(t341-t583);
t1625 = t5.*t288.*t603.*2.170133333335e-2;
t1643 = t562.*t1247;
t1644 = (t622.*t1005)./2.0;
t1650 = t7.*t292.*t605.*3.333333333335e-5;
t1661 = t618+t1120;
t1662 = t547.*t1394;
t1666 = -t1656;
t1668 = ((t71-t445).*(t595-t596))./2.0;
t1679 = t187+t358+t1337;
t1683 = t619+t1187;
t1713 = -t1705;
t1717 = -t1701;
t1718 = -t1702;
t1720 = t172+t216+t304+t338+t377+t582;
t1769 = -t1744;
t1774 = -t1750;
t1778 = -t1752;
t1789 = -t1762;
t1791 = t1187.*3.333333333335e-5;
t1809 = t3.*t1762;
t1811 = t13.*t592.*(t160-t1026).*(-1.0./1.0e+1);
t1824 = -t1800;
t1827 = -t1806;
t1830 = t7.*t607.*(t160-t1026).*(-1.0./1.0e+1);
t1834 = (t13.*t592.*(t160-t1026))./1.0e+1;
t1835 = t7.*t605.*(t71-t445).*(-1.6666666666675e-5);
t1837 = t12.*t40.*(t509-t621).*(-1.6666666666675e-5);
t1838 = t4.*t1800;
t1841 = t733.*t1247.*2.0;
t1843 = (t7.*t607.*(t160-t1026))./1.0e+1;
t1844 = t7.*t605.*(t71-t445).*1.6666666666675e-5;
t1845 = t12.*t40.*(t509-t621).*1.6666666666675e-5;
t1853 = t7.*t640.*(t160-t1026).*(-1.0./1.0e+1);
t1856 = t838+t1119;
t1858 = -t1850;
t1859 = t11.*t12.*t1005.*6.810416666674999e-4;
t1861 = (t7.*t640.*(t160-t1026))./1.0e+1;
t1862 = t13.*t655.*(t160-t1026).*(-1.0./1.0e+1);
t1863 = t1017+t1028;
t1865 = t877+t1122;
t1874 = (t13.*t655.*(t160-t1026))./1.0e+1;
t1876 = t849+t1175;
t1877 = t861+t1161;
t1890 = t893+t1164;
t1891 = t891+t1172;
t1896 = -t1868;
t1908 = t864.*t1247.*2.0;
t1915 = (t11.*t1849)./2.0;
t1918 = t934+t1228;
t1922 = t13.*t292.*(t509-t621).*(-1.6666666666675e-5);
t1924 = (t5.*t1855)./2.0;
t1928 = -t1916;
t1930 = t956+t1235;
t1932 = t13.*t292.*(t509-t621).*1.6666666666675e-5;
t1934 = (t5.*t10.*t1849)./2.0;
t1939 = (t160-t1026).*(t151+t12.*(t157-t10.*t38.*(3.9e+1./1.0e+2))).*(6.0./5.0);
t1946 = (t5.*t6.*t1857)./2.0;
t1947 = (t10.*t11.*t1855)./2.0;
t1957 = t288.*t1800;
t1960 = (t5.*t12.*t1866)./2.0;
t1966 = (t11.*t34.*t1857)./2.0;
t1975 = (t11.*t39.*t1866)./2.0;
t1982 = (t655.*(t624-t818))./1.0e+1;
t1988 = t988+t1397;
t1989 = t1158+t1173;
t1998 = t12.*t864.*(t160-t1026).*(-6.0./5.0);
t2003 = t1018+t1380;
t2006 = (t6.*t11.*t1920)./2.0;
t2009 = -t1994;
t2010 = -t1995;
t2016 = (t11.*t12.*t1931)./2.0;
t2026 = t1191.*t1247.*2.0;
t2028 = (t293.*t1857)./2.0;
t2031 = t603.*t1719;
t2033 = t6.*t399.*t1857;
t2034 = (t603.*t1685)./2.0;
t2035 = (t603.*t1686)./2.0;
t2037 = -t2027;
t2042 = t13.*(t71-t445).*(t509-t621).*3.333333333335e-5;
t2044 = t478.*t1866;
t2046 = t12.*t399.*t1866;
t2058 = t526.*t1857;
t2062 = (t603.*t1709)./2.0;
t2066 = (t402.*t1866)./2.0;
t2077 = t1247.*t1394;
t2093 = t605.*t1828;
t2095 = t1163+t1457;
t2104 = (t169-t960).*(t160-t1026).*(6.0./5.0);
t2111 = t603.*t1849;
t2120 = t1247.*t1469;
t2124 = t616.*t1866;
t2129 = t1140+t1511;
t2131 = -t1855.*(t67-t512);
t2133 = -t1857.*(t69-t508);
t2151 = (t741.*t1710)./2.0;
t2152 = t292.*(t1159-t1162).*(-1.0./2.0);
t2162 = t605.*t1907;
t2166 = (t292.*(t1159-t1162))./2.0;
t2171 = t592.*(t1020-t1024).*(-1.0./1.0e+1);
t2172 = -t1898.*(t75-t518);
t2184 = (t573.*t1920)./2.0;
t2185 = (t664.*t1857)./2.0;
t2186 = t6.*t1857.*(t67-t512).*(-1.0./2.0);
t2187 = (t6.*t11.*(t1174+t6.*(t65-t437).*1.302083333335e-3))./2.0;
t2195 = (t6.*t1857.*(t67-t512))./2.0;
t2196 = t12.*t1866.*(t67-t512).*(-1.0./2.0);
t2206 = (t12.*t1866.*(t67-t512))./2.0;
t2216 = t1931.*(t71-t445).*(-1.0./2.0);
t2217 = t1866.*(t111-t536).*(-1.0./2.0);
t2219 = (t1229+t8.*t56.*(2.0./5.0)).*(t160-t1026).*(-3.0./5.0);
t2221 = t655.*(t1020-t1024).*(-1.0./1.0e+1);
t2226 = (t1931.*(t71-t445))./2.0;
t2227 = (t1866.*(t111-t536))./2.0;
t2229 = (t1229+t8.*t56.*(2.0./5.0)).*(t160-t1026).*(3.0./5.0);
t2242 = (t741.*t1857)./2.0;
t2243 = (t1005.*t1695)./2.0;
t2267 = ((t71-t445).*(t1159-t1162))./2.0;
t2268 = t1866.*(t499-t506).*(-1.0./2.0);
t2282 = t1736.*(t509-t621).*(-1.0./2.0);
t2290 = (t401.*(t1174+t6.*(t65-t437).*1.302083333335e-3))./2.0;
t2333 = t1842.*(t509-t621).*(-1.0./2.0);
t2382 = (t1898.*(t509-t621))./2.0;
t2406 = (t607.*t2160)./1.0e+1;
t2413 = (t592.*t2181)./1.0e+1;
t2466 = (t509-t621).*(t1135+t13.*(t69-t508).*3.333333333335e-5);
t2537 = t198+t297+t657+t1058+t1699;
t2599 = -t2597;
t2660 = -t2659;
t2663 = -t2662;
t2665 = q_dot4.*(t528+t767+t768+t1377+t1381+t1864+t1875+t6.*t12.*t22.*1.2e-4);
t729 = t642.*6.0e-5;
t731 = t645.*6.0e-5;
t770 = t446+t552;
t887 = (t5.*t747)./2.0;
t943 = (t10.*t11.*t747)./2.0;
t947 = t438+t645;
t965 = t4.*t913;
t971 = -t944;
t1003 = (t11.*t12.*t798)./2.0;
t1084 = -t7.*(t444-t642);
t1121 = t7.*(t444-t642);
t1194 = t7.*t1095;
t1196 = t13.*t1095;
t1259 = -t1203;
t1277 = -t1226;
t1299 = -t1255;
t1304 = (t399.*t747)./2.0;
t1329 = t5.*t1044.*(3.1e+1./2.5e+2);
t1339 = t549+t728;
t1354 = -t1319;
t1368 = t500+t793;
t1399 = t4.*t5.*t1044.*(-3.1e+1./2.5e+2);
t1402 = t11.*t12.*(t444-t642).*(-3.0e-5);
t1412 = t164+t248+t332+t598;
t1417 = t7.*t1376;
t1419 = t13.*t1376;
t1428 = t646+t697;
t1435 = t7.*t1411;
t1439 = t13.*t1411;
t1451 = t11.*t34.*t1095.*(3.9e+1./2.0e+2);
t1453 = t11.*t39.*t1082.*(1.17e+2./5.0e+2);
t1456 = t642.*1.302083333335e-3;
t1459 = t645.*1.302083333335e-3;
t1460 = t644+t723;
t1482 = -t1466;
t1485 = -t798.*(t71-t445);
t1486 = -t747.*(t67-t512);
t1491 = t644.*3.333333333335e-5;
t1494 = t646.*3.333333333335e-5;
t1504 = -t1492;
t1506 = -t1495;
t1518 = t5.*t1411.*(3.9e+1./2.0e+2);
t1520 = t6.*t11.*t1376.*(3.9e+1./2.0e+2);
t1527 = (t11.*t12.*t1418)./2.0;
t1535 = t5.*t12.*t1376.*(3.9e+1./1.0e+3);
t1556 = -t1543;
t1562 = t551.*t1044;
t1563 = t11.*t27.*t1376.*(3.9e+1./2.0e+2);
t1564 = t59.*t1376.*(3.9e+1./2.0e+2);
t1566 = t11.*t39.*t1376.*(3.9e+1./1.0e+3);
t1573 = t4.*t5.*t1411.*(1.17e+2./2.0e+2);
t1575 = t10.*t11.*t1411.*(1.17e+2./2.0e+2);
t1579 = t255+t1413;
t1594 = t305+t1415;
t1596 = t5.*t17.*t1411.*(-3.9e+1./2.0e+2);
t1598 = t5.*t23.*t1411.*(1.17e+2./5.0e+2);
t1610 = t10.*t11.*t17.*t1411.*(3.9e+1./2.0e+2);
t1616 = -t1604;
t1617 = t608.*t1044;
t1621 = t10.*t11.*t23.*t1411.*(1.17e+2./5.0e+2);
t1632 = t790.*3.333333333335e-5;
t1633 = t793.*3.333333333335e-5;
t1645 = (t292.*t1418)./2.0;
t1657 = -t1643;
t1681 = t547.*t1411;
t1684 = -t1662;
t1692 = t715.*t1044;
t1707 = t1044.*(t163-t557).*-2.0;
t1734 = t574.*t1411.*(3.0./2.0);
t1759 = t5.*t6.*(t444-t642).*(-6.510416666674999e-4);
t1779 = t1044.*(t341-t583).*2.0;
t1785 = t784.*t1044.*2.0;
t1787 = ((t386-t572).*(t444-t642))./2.0;
t1790 = t12.*t36.*t948.*1.6666666666675e-5;
t1817 = t5.*t1679.*(3.9e+1./1.0e+2);
t1852 = t11.*t1720.*(3.9e+1./1.0e+2);
t1870 = -t1859;
t1873 = t996.*t1044.*2.0;
t1881 = t5.*t10.*t1720.*(3.9e+1./1.0e+2);
t1885 = t1411.*(t555-t37.*t38.*(2.0./5.0)).*3.0;
t1886 = t778.*t1376;
t1900 = t7.*t292.*t948.*1.6666666666675e-5;
t1926 = -t1915;
t1927 = (t5.*t1856)./2.0;
t1929 = t6.*t399.*(t444-t642).*(-6.510416666674999e-4);
t1937 = (t11.*t1865)./2.0;
t1938 = t6.*t399.*(t444-t642).*6.510416666674999e-4;
t1942 = (t640.*t1519)./1.0e+1;
t1948 = (t10.*t11.*t1856)./2.0;
t1949 = (t5.*t1877)./2.0;
t1953 = t6.*t864.*t1376;
t1956 = t4.*t5.*t1856.*(-1.0./2.0);
t1958 = t547.*t1679;
t1959 = (t5.*t10.*t1865)./2.0;
t1962 = (t11.*t1891)./2.0;
t1965 = (t10.*t32.*t1856)./2.0;
t1968 = (t11.*t12.*t1876)./2.0;
t1969 = (t10.*t11.*t1877)./2.0;
t1973 = (t6.*t11.*t1890)./2.0;
t1977 = (t5.*t10.*t1891)./2.0;
t1985 = t4.*t11.*t1891.*(-1.0./2.0);
t1991 = t1027+t1385;
t1999 = (t10.*t38.*t1891)./2.0;
t2007 = t919.*t1411.*(3.0./2.0);
t2008 = t920.*t1411.*(3.0./2.0);
t2012 = t562.*t1720;
t2022 = t5.*t288.*t1856;
t2025 = t7.*t948.*(t71-t445).*(-3.333333333335e-5);
t2029 = t1134+t1321;
t2030 = t1088.*t1411.*3.0;
t2032 = t477.*t1856;
t2036 = (t290.*t1865)./2.0;
t2038 = -t2028;
t2045 = t11.*t288.*t1891;
t2047 = -t2034;
t2048 = -t2035;
t2051 = (t399.*t1856)./2.0;
t2052 = (t400.*t1856)./2.0;
t2053 = (t1095.*t1376)./2.0;
t2054 = t1082.*(t160-t1026).*(-3.0./5.0);
t2056 = t6.*(t67-t512).*(t444-t642).*1.302083333335e-3;
t2063 = (t290.*t1891)./2.0;
t2064 = (t291.*t1891)./2.0;
t2069 = -t2044;
t2070 = t1275.*t1376;
t2071 = -t2062;
t2076 = (t399.*t1877)./2.0;
t2082 = t1247.*t1411;
t2083 = t7.*t292.*t1918;
t2086 = t525.*t1891;
t2088 = t13.*t292.*t1930;
t2094 = t479.*t1918;
t2105 = t1234+t1465;
t2114 = t1278+t1468;
t2117 = t527.*t1930;
t2118 = t1411.*(t246+t330-t556-t2.*t26.*(2.0./5.0)).*-3.0;
t2121 = -t1856.*(t65-t437);
t2122 = t588.*t1891;
t2123 = t573.*t1890;
t2126 = t603.*t1865;
t2128 = (t1376.*(t160-t1026))./5.0;
t2130 = t733.*t1720;
t2132 = -t1876.*(t71-t445);
t2138 = -t2120;
t2141 = t603.*t1891;
t2145 = (t6.*t1376.*t1411)./2.0;
t2147 = t12.*t1411.*(t160-t1026).*(-3.0./5.0);
t2148 = t1856.*(t67-t512);
t2149 = -t1877.*(t67-t512);
t2156 = (t11.*t12.*t2095)./2.0;
t2158 = t12.*t1411.*(t160-t1026).*(3.0./5.0);
t2161 = (t607.*t1863)./1.0e+1;
t2163 = t589.*t1930;
t2164 = t12.*t40.*(t7.*(t67-t512)+t13.*(t444-t642)).*(-1.6666666666675e-5);
t2165 = -t2151;
t2168 = (t401.*t1989)./2.0;
t2173 = -t1918.*(t73-t442);
t2175 = t12.*t40.*(t7.*(t67-t512)+t13.*(t444-t642)).*1.6666666666675e-5;
t2188 = (t640.*t1863)./1.0e+1;
t2191 = (t742.*t1760)./2.0;
t2192 = t864.*t1720;
t2193 = -t2184;
t2194 = -t2185;
t2205 = t1379+t1542;
t2218 = t1376.*(t256+t6.*(t176+t314+t459+t26.*t30.*(2.0./5.0))).*(-1.0./2.0);
t2224 = t7.*t1918.*(t71-t445).*(-1.0./2.0);
t2228 = (t1376.*(t256+t6.*(t176+t314+t459+t26.*t30.*(2.0./5.0))))./2.0;
t2232 = (t7.*t1918.*(t71-t445))./2.0;
t2233 = t13.*t1930.*(t71-t445).*(-1.0./2.0);
t2236 = (t13.*t1930.*(t71-t445))./2.0;
t2240 = t13.*t292.*(t7.*(t67-t512)+t13.*(t444-t642)).*(-1.6666666666675e-5);
t2241 = (t573.*t1989)./2.0;
t2244 = (t292.*t2095)./2.0;
t2247 = t1696.*(t444-t642).*(-1.0./2.0);
t2249 = (t605.*t1988)./2.0;
t2250 = (t694.*t1918)./2.0;
t2253 = -t2242;
t2254 = (t1696.*(t444-t642))./2.0;
t2264 = (t948.*t1761)./2.0;
t2276 = t592.*(t1023-t1387).*(-1.0./1.0e+1);
t2279 = (t1006.*t1735)./2.0;
t2280 = (t294.*t2129)./2.0;
t2284 = t2003.*(t75-t518).*(-1.0./2.0);
t2285 = t1930.*(t113-t554).*(-1.0./2.0);
t2293 = (t592.*(t1023-t1387))./1.0e+1;
t2302 = t1765.*(t444-t642).*(-1.0./2.0);
t2307 = (t948.*t1828)./2.0;
t2311 = (t1765.*(t444-t642))./2.0;
t2315 = t1191.*t1720;
t2318 = (t742.*t1930)./2.0;
t2344 = t1394.*t1720.*2.0;
t2351 = (t1252.*t1735)./2.0;
t2352 = t13.*(t7.*(t67-t512)+t13.*(t444-t642)).*(t71-t445).*1.6666666666675e-5;
t2353 = t1411.*t1720.*2.0;
t2362 = t1890.*(t444-t642).*(-1.0./2.0);
t2365 = (t948.*t1907)./2.0;
t2367 = -t1920.*(t444-t642);
t2371 = (t1890.*(t444-t642))./2.0;
t2387 = t1469.*t1720.*2.0;
t2388 = t948.*t1988;
t2394 = t1462+t1767;
t2400 = t1464+t1791;
t2401 = -t2003.*(t509-t621);
t2403 = -t1989.*(t444-t642);
t2438 = t1918.*(t501-t790).*(-1.0./2.0);
t2442 = (t1918.*(t501-t790))./2.0;
t2446 = t12.*t40.*(t7.*(t67-t512).*3.333333333335e-5+t13.*(t444-t642).*3.333333333335e-5).*(-1.0./2.0);
t2452 = (t12.*t40.*(t7.*(t67-t512).*3.333333333335e-5+t13.*(t444-t642).*3.333333333335e-5))./2.0;
t2454 = (t1174+t6.*(t65-t437).*1.302083333335e-3).*(t444-t642);
t2456 = t948.*t2129;
t2462 = t1679.*t1720.*2.0;
t2473 = (t1661.*t1760)./2.0;
t2475 = t1736.*(t7.*(t67-t512)+t13.*(t444-t642)).*(-1.0./2.0);
t2476 = t295.*(t7.*(t67-t512).*3.333333333335e-5+t13.*(t444-t642).*3.333333333335e-5).*(-1.0./2.0);
t2481 = (t1683.*t1735)./2.0;
t2488 = t13.*t292.*(t7.*(t67-t512).*3.333333333335e-5+t13.*(t444-t642).*3.333333333335e-5).*(-1.0./2.0);
t2498 = t1842.*(t7.*(t67-t512)+t13.*(t444-t642)).*(-1.0./2.0);
t2507 = t527.*(t7.*(t67-t512).*3.333333333335e-5+t13.*(t444-t642).*3.333333333335e-5).*(-1.0./2.0);
t2524 = t1898.*(t7.*(t67-t512)+t13.*(t444-t642)).*(-1.0./2.0);
t2525 = t589.*(t7.*(t67-t512).*3.333333333335e-5+t13.*(t444-t642).*3.333333333335e-5).*(-1.0./2.0);
t2529 = (t1661.*t1930)./2.0;
t2530 = (t1898.*(t7.*(t67-t512)+t13.*(t444-t642)))./2.0;
t2531 = (t589.*(t7.*(t67-t512).*3.333333333335e-5+t13.*(t444-t642).*3.333333333335e-5))./2.0;
t2536 = (t1683.*t1918)./2.0;
t2543 = (t13.*(t7.*(t67-t512).*3.333333333335e-5+t13.*(t444-t642).*3.333333333335e-5).*(t71-t445))./2.0;
t2555 = t2003.*(t7.*(t67-t512)+t13.*(t444-t642)).*(-1.0./2.0);
t2558 = (t2003.*(t7.*(t67-t512)+t13.*(t444-t642)))./2.0;
t2560 = ((t7.*(t67-t512).*3.333333333335e-5+t13.*(t444-t642).*3.333333333335e-5).*(t113-t554))./2.0;
t2564 = t742.*(t7.*(t67-t512).*3.333333333335e-5+t13.*(t444-t642).*3.333333333335e-5).*(-1.0./2.0);
t2566 = (t742.*(t7.*(t67-t512).*3.333333333335e-5+t13.*(t444-t642).*3.333333333335e-5))./2.0;
t2586 = ((t7.*(t67-t512)+t13.*(t444-t642)).*(t1135+t13.*(t69-t508).*3.333333333335e-5))./2.0;
t2593 = ((t441+t13.*(t69-t508)).*(t7.*(t67-t512).*3.333333333335e-5+t13.*(t444-t642).*3.333333333335e-5))./2.0;
t2627 = -t1661.*(t7.*(t67-t512).*3.333333333335e-5+t13.*(t444-t642).*3.333333333335e-5);
t2656 = t1154+t1155+t1497+t1717+t1718;
t2666 = -t2665;
t2672 = t1094+t1113+t1125+t1220+t1221+t1940+t1941+t1951+t1952;
t2680 = t200+t2021+t2359+t2583+t2660+t2669;
t911 = -t887;
t1047 = -t1003;
t1295 = -t1196;
t1346 = -t1304;
t1363 = t6.*t11.*t947.*3.0e-5;
t1386 = t566+t731;
t1434 = t6.*t1412;
t1436 = t7.*t1412;
t1438 = t12.*t1412;
t1440 = t13.*t1412;
t1474 = -t1451;
t1478 = -t1453;
t1483 = t6.*t1435;
t1484 = t6.*t1439;
t1509 = t11.*t12.*(t571-t729).*(-1.0./2.0);
t1534 = -t1520;
t1536 = t11.*t1412.*(1.17e+2./2.0e+2);
t1539 = -t1527;
t1552 = -t1535;
t1574 = t5.*t10.*t1412.*(1.17e+2./2.0e+2);
t1577 = -t1566;
t1584 = -t1573;
t1611 = -t1598;
t1622 = t7.*t1579;
t1624 = t13.*t1579;
t1628 = (t632.*t947)./2.0;
t1629 = (t633.*t947)./2.0;
t1635 = -t1617;
t1659 = (t671.*t947)./2.0;
t1698 = t5.*t6.*t1579.*(3.9e+1./2.0e+2);
t1714 = -t1692;
t1715 = t11.*t34.*t1579.*(3.9e+1./2.0e+2);
t1716 = t5.*t12.*t1594.*(1.17e+2./5.0e+2);
t1726 = (t748.*t947)./2.0;
t1729 = t11.*t39.*t1594.*(1.17e+2./5.0e+2);
t1743 = t1121.*3.333333333335e-5;
t1757 = (t798.*t947)./2.0;
t1786 = ((t71-t445).*(t571-t729))./2.0;
t1799 = -t947.*(t464-t623);
t1813 = -t1787;
t1816 = -t1790;
t1846 = t5.*t12.*t947.*6.810416666674999e-4;
t1848 = t766+t1194;
t1867 = t11.*t39.*t947.*6.810416666674999e-4;
t1899 = t7.*t294.*t947.*1.6666666666675e-5;
t1906 = t947.*(t595-t596);
t1910 = -t1900;
t1921 = t13.*t403.*t947.*1.6666666666675e-5;
t1945 = t4.*t1927;
t1950 = -t1937;
t1961 = -t1949;
t1976 = t4.*t1962;
t1978 = -t1968;
t1981 = t12.*t399.*t947.*6.810416666674999e-4;
t1983 = t864.*t1412.*(3.0./2.0);
t1984 = -t1973;
t1990 = t959+t1419;
t2001 = t947.*t1418;
t2017 = -t2007;
t2018 = -t2008;
t2023 = -t2012;
t2024 = t7.*t605.*t947.*1.6666666666675e-5;
t2039 = t1139+t1354;
t2049 = -t2036;
t2060 = -t2051;
t2061 = -t2052;
t2068 = -t2056;
t2072 = -t2063;
c_num = ft_4({q_dot1,q_dot2,q_dot3,q_dot4,q_dot5,q_dot6,q_dot7,t10,t1000,t1002,t1003,t1004,t1005,t1006,t1007,t1008,t1009,t1014,t1020,t1023,t1024,t1026,t1031,t1032,t1033,t1034,t1035,t1036,t1037,t1038,t1039,t104,t1041,t1044,t1045,t1047,t1048,t1049,t1050,t1051,t1053,t1054,t1055,t1056,t1057,t1059,t1060,t1061,t1062,t1065,t1068,t1071,t1072,t1074,t1075,t1077,t1078,t1079,t1080,t1082,t1084,t1088,t1092,t1093,t1095,t1096,t1097,t1099,t11,t110,t1100,t1101,t1102,t1104,t1108,t111,t1118,t1124,t1127,t113,t1131,t1132,t1135,t1142,t1143,t1144,t1147,t1149,t1150,t1152,t1153,t1156,t1157,t1159,t1160,t1162,t1165,t1166,t1167,t1168,t1174,t1181,t1184,t1190,t1191,t1195,t1197,t1198,t1199,t12,t1200,t1201,t1202,t1203,t1205,t1206,t1207,t1208,t1209,t1215,t1217,t1218,t1219,t1222,t1225,t1229,t1230,t1231,t1233,t1237,t1240,t1241,t1242,t1244,t1246,t1247,t1248,t1249,t1250,t1252,t1255,t1256,t1257,t1258,t1259,t1261,t1264,t1265,t1268,t1270,t1271,t1274,t1275,t1276,t1277,t1279,t1280,t1283,t1285,t1286,t1289,t1293,t1295,t1298,t1299,t13,t1300,t1301,t1302,t1303,t1304,t1305,t1306,t1309,t1310,t1312,t1313,t1314,t1316,t1318,t1320,t1322,t1323,t1324,t1325,t1327,t1328,t1329,t1330,t1334,t1339,t1340,t1341,t1342,t1343,t1344,t1345,t1346,t1347,t1348,t1349,t1350,t1351,t1352,t1355,t1356,t1357,t1358,t1359,t1360,t1361,t1362,t1363,t1364,t1367,t1368,t1369,t1373,t1374,t1375,t1376,t1377,t1378,t1381,t1382,t1386,t1387,t1388,t1389,t1390,t1391,t1394,t1396,t1398,t1399,t140,t1400,t1402,t1403,t1404,t1405,t1406,t1407,t1409,t1411,t1412,t1414,t1416,t1417,t1418,t1420,t1421,t1423,t1424,t1425,t1426,t1427,t1428,t1429,t1430,t1432,t1433,t1434,t1435,t1436,t1437,t1438,t1439,t1440,t1441,t1442,t1446,t1448,t1450,t1451,t1453,t1455,t1456,t1458,t1459,t1460,t1461,t1463,t1466,t1467,t1469,t147,t1470,t1471,t1472,t1473,t1474,t1475,t1476,t1477,t1478,t1480,t1481,t1482,t1483,t1484,t1485,t1486,t1487,t1489,t1491,t1492,t1493,t1494,t1495,t1496,t1498,t1499,t1502,t1503,t1504,t1506,t1508,t1509,t151,t1512,t1513,t1514,t1517,t1518,t1519,t1520,t1521,t1522,t1523,t1524,t1526,t1528,t1531,t1534,t1535,t1536,t1537,t1538,t1539,t1540,t1541,t1544,t1546,t1547,t1549,t1550,t1552,t1553,t1554,t1555,t1556,t1557,t1558,t1560,t1561,t1562,t1563,t1564,t1565,t1566,t1567,t1568,t157,t1571,t1573,t1574,t1575,t1576,t1577,t1578,t1579,t1582,t1583,t1584,t1585,t1587,t1589,t1590,t1591,t1592,t1593,t1594,t1595,t1596,t1597,t160,t1601,t1602,t1603,t1604,t1605,t1606,t1608,t1609,t1610,t1611,t1612,t1613,t1615,t1616,t1617,t1618,t1619,t1621,t1622,t1624,t1625,t1626,t1628,t1629,t163,t1632,t1633,t1635,t1636,t1644,t1645,t1648,t1649,t1650,t1653,t1655,t1657,t1659,t1661,t1662,t1663,t1664,t1665,t1666,t1668,t1669,t1671,t1674,t1678,t1679,t1680,t1681,t1682,t1683,t1684,t1686,t1688,t169,t1690,t1692,t1694,t1695,t1698,t17,t1700,t1703,t1704,t1706,t1707,t1709,t1710,t1711,t1713,t1714,t1715,t1716,t1719,t1726,t1729,t1730,t1733,t1734,t1735,t1736,t1739,t1740,t1741,t1743,t1745,t1749,t1750,t1752,t1753,t1756,t1757,t1759,t176,t1760,t1761,t1762,t1763,t1764,t1765,t1769,t1770,t1771,t1772,t1774,t1775,t1776,t1778,t1779,t1782,t1785,t1786,t1787,t1788,t1789,t1790,t1792,t1793,t1794,t1795,t1796,t1797,t1798,t1799,t1800,t1804,t1806,t1808,t1809,t1811,t1813,t1814,t1815,t1816,t1817,t1818,t1819,t1820,t1822,t1824,t1827,t1828,t1830,t1831,t1832,t1833,t1834,t1835,t1837,t1838,t1839,t1841,t1842,t1843,t1844,t1845,t1846,t1848,t1849,t1850,t1851,t1852,t1853,t1855,t1857,t1858,t1861,t1862,t1863,t1864,t1866,t1867,t1869,t1870,t1871,t1872,t1873,t1874,t1875,t1876,t1878,t1879,t1880,t1881,t1883,t1885,t1886,t1887,t1888,t1890,t1892,t1893,t1894,t1896,t1899,t1900,t1901,t1902,t1903,t1904,t1905,t1906,t1907,t1908,t1910,t1911,t1912,t1913,t1914,t1916,t1918,t1920,t1921,t1922,t1923,t1924,t1926,t1927,t1928,t1929,t1930,t1931,t1932,t1933,t1934,t1938,t1939,t1942,t1943,t1944,t1945,t1946,t1947,t1948,t1950,t1953,t1954,t1955,t1956,t1957,t1958,t1959,t1960,t1961,t1962,t1963,t1964,t1965,t1966,t1967,t1968,t1969,t1972,t1973,t1975,t1976,t1977,t1978,t1981,t1982,t1983,t1984,t1985,t1988,t1989,t199,t1990,t1991,t1994,t1995,t1996,t1997,t1998,t1999,t2,t2001,t2003,t2005,t2006,t2007,t2008,t2009,t2010,t2012,t2016,t2017,t2018,t2022,t2023,t2024,t2025,t2026,t2029,t2030,t2031,t2032,t2033,t2034,t2035,t2036,t2037,t2038,t2039,t2042,t2043,t2045,t2046,t2047,t2048,t2049,t2050,t2051,t2052,t2053,t2054,t2058,t2059,t2060,t2061,t2062,t2063,t2064,t2065,t2066,t2068,t2069,t2070,t2071,t2072,t2074,t2075,t2076,t2077,t2078,t2079,t2080,t2082,t2083,t2086,t2088,t2090,t2093,t2094,t2095,t2097,t2101,t2104,t2105,t2109,t2110,t2111,t2114,t2117,t2118,t2119,t2120,t2121,t2122,t2123,t2124,t2126,t2128,t2129,t2130,t2131,t2132,t2133,t2138,t2141,t2145,t2147,t2148,t2149,t2151,t2152,t2156,t2158,t2160,t2161,t2162,t2163,t2164,t2165,t2166,t2167,t2168,t2171,t2172,t2173,t2175,t2176,t2181,t2184,t2185,t2186,t2187,t2188,t2191,t2192,t2193,t2194,t2195,t2196,t22,t2205,t2206,t2216,t2217,t2218,t2219,t2221,t2224,t2226,t2227,t2228,t2229,t2232,t2233,t2236,t2240,t2241,t2242,t2243,t2244,t2247,t2249,t2250,t2253,t2254,t2264,t2267,t2268,t227,t2276,t2279,t228,t2280,t2282,t2284,t2285,t2289,t2290,t2293,t2302,t2307,t2311,t2315,t2318,t2319,t2320,t2325,t2326,t2333,t2344,t2348,t2349,t2351,t2352,t2353,t2362,t2365,t2367,t2371,t2382,t2387,t2388,t2394,t2400,t2401,t2403,t2406,t2413,t2438,t2442,t2446,t2452,t2454,t2456,t246,t2462,t2466,t2473,t2475,t2476,t2481,t2488,t2498,t2507,t2524,t2525,t2529,t2530,t2531,t2536,t2537,t2543,t2555,t2558,t256,t2560,t2564,t2566,t2571,t2572,t2577,t2582,t2586,t2593,t2597,t2599,t26,t261,t262,t2627,t264,t2655,t2656,t2657,t2658,t2661,t2662,t2663,t2665,t2666,t2667,t2668,t2672,t2680,t27,t274,t276,t28,t288,t289,t29,t290,t291,t292,t293,t294,t295,t296,t298,t299,t3,t30,t300,t301,t307,t31,t314,t32,t33,t330,t34,t341,t344,t346,t35,t351,t354,t359,t36,t361,t362,t366,t37,t38,t386,t388,t389,t39,t395,t396,t398,t399,t4,t40,t400,t401,t402,t403,t404,t405,t406,t407,t411,t418,t419,t421,t422,t43,t432,t433,t435,t437,t441,t442,t444,t445,t450,t451,t459,t461,t464,t473,t475,t476,t477,t478,t479,t480,t481,t482,t483,t493,t494,t495,t496,t499,t5,t501,t502,t506,t508,t509,t51,t512,t514,t518,t522,t524,t525,t526,t527,t528,t53,t530,t531,t532,t533,t536,t54,t544,t545,t546,t547,t548,t55,t551,t554,t555,t556,t557,t56,t564,t565,t568,t569,t570,t571,t572,t573,t574,t583,t584,t586,t588,t589,t59,t591,t592,t594,t595,t596,t6,t600,t601,t605,t606,t607,t608,t609,t612,t614,t616,t621,t622,t623,t624,t626,t627,t628,t637,t638,t640,t641,t642,t647,t649,t65,t650,t652,t654,t655,t656,t658,t659,t66,t660,t661,t662,t664,t665,t666,t668,t669,t67,t671,t676,t677,t678,t679,t680,t682,t683,t684,t686,t689,t69,t690,t691,t692,t694,t696,t699,t7,t700,t701,t702,t703,t704,t707,t708,t709,t71,t710,t711,t712,t713,t714,t715,t717,t72,t720,t721,t722,t725,t726,t729,t73,t732,t733,t734,t735,t737,t739,t740,t741,t742,t743,t744,t745,t746,t75,t751,t758,t759,t760,t764,t765,t767,t768,t770,t771,t773,t774,t775,t776,t777,t778,t781,t782,t783,t784,t788,t790,t792,t798,t8,t801,t802,t803,t811,t812,t815,t816,t818,t819,t821,t822,t823,t825,t826,t829,t842,t843,t853,t854,t864,t865,t868,t869,t872,t879,t880,t883,t884,t885,t895,t896,t897,t899,t9,t902,t905,t911,t913,t914,t916,t919,t921,t922,t924,t933,t937,t938,t939,t943,t944,t947,t948,t949,t953,t954,t960,t961,t962,t963,t964,t965,t966,t967,t968,t969,t971,t972,t973,t974,t975,t977,t980,t982,t983,t984,t990,t991,t994,t995,t996,t998,t999});
end
function c_num = ft_4(ct)
[q_dot1,q_dot2,q_dot3,q_dot4,q_dot5,q_dot6,q_dot7,t10,t1000,t1002,t1003,t1004,t1005,t1006,t1007,t1008,t1009,t1014,t1020,t1023,t1024,t1026,t1031,t1032,t1033,t1034,t1035,t1036,t1037,t1038,t1039,t104,t1041,t1044,t1045,t1047,t1048,t1049,t1050,t1051,t1053,t1054,t1055,t1056,t1057,t1059,t1060,t1061,t1062,t1065,t1068,t1071,t1072,t1074,t1075,t1077,t1078,t1079,t1080,t1082,t1084,t1088,t1092,t1093,t1095,t1096,t1097,t1099,t11,t110,t1100,t1101,t1102,t1104,t1108,t111,t1118,t1124,t1127,t113,t1131,t1132,t1135,t1142,t1143,t1144,t1147,t1149,t1150,t1152,t1153,t1156,t1157,t1159,t1160,t1162,t1165,t1166,t1167,t1168,t1174,t1181,t1184,t1190,t1191,t1195,t1197,t1198,t1199,t12,t1200,t1201,t1202,t1203,t1205,t1206,t1207,t1208,t1209,t1215,t1217,t1218,t1219,t1222,t1225,t1229,t1230,t1231,t1233,t1237,t1240,t1241,t1242,t1244,t1246,t1247,t1248,t1249,t1250,t1252,t1255,t1256,t1257,t1258,t1259,t1261,t1264,t1265,t1268,t1270,t1271,t1274,t1275,t1276,t1277,t1279,t1280,t1283,t1285,t1286,t1289,t1293,t1295,t1298,t1299,t13,t1300,t1301,t1302,t1303,t1304,t1305,t1306,t1309,t1310,t1312,t1313,t1314,t1316,t1318,t1320,t1322,t1323,t1324,t1325,t1327,t1328,t1329,t1330,t1334,t1339,t1340,t1341,t1342,t1343,t1344,t1345,t1346,t1347,t1348,t1349,t1350,t1351,t1352,t1355,t1356,t1357,t1358,t1359,t1360,t1361,t1362,t1363,t1364,t1367,t1368,t1369,t1373,t1374,t1375,t1376,t1377,t1378,t1381,t1382,t1386,t1387,t1388,t1389,t1390,t1391,t1394,t1396,t1398,t1399,t140,t1400,t1402,t1403,t1404,t1405,t1406,t1407,t1409,t1411,t1412,t1414,t1416,t1417,t1418,t1420,t1421,t1423,t1424,t1425,t1426,t1427,t1428,t1429,t1430,t1432,t1433,t1434,t1435,t1436,t1437,t1438,t1439,t1440,t1441,t1442,t1446,t1448,t1450,t1451,t1453,t1455,t1456,t1458,t1459,t1460,t1461,t1463,t1466,t1467,t1469,t147,t1470,t1471,t1472,t1473,t1474,t1475,t1476,t1477,t1478,t1480,t1481,t1482,t1483,t1484,t1485,t1486,t1487,t1489,t1491,t1492,t1493,t1494,t1495,t1496,t1498,t1499,t1502,t1503,t1504,t1506,t1508,t1509,t151,t1512,t1513,t1514,t1517,t1518,t1519,t1520,t1521,t1522,t1523,t1524,t1526,t1528,t1531,t1534,t1535,t1536,t1537,t1538,t1539,t1540,t1541,t1544,t1546,t1547,t1549,t1550,t1552,t1553,t1554,t1555,t1556,t1557,t1558,t1560,t1561,t1562,t1563,t1564,t1565,t1566,t1567,t1568,t157,t1571,t1573,t1574,t1575,t1576,t1577,t1578,t1579,t1582,t1583,t1584,t1585,t1587,t1589,t1590,t1591,t1592,t1593,t1594,t1595,t1596,t1597,t160,t1601,t1602,t1603,t1604,t1605,t1606,t1608,t1609,t1610,t1611,t1612,t1613,t1615,t1616,t1617,t1618,t1619,t1621,t1622,t1624,t1625,t1626,t1628,t1629,t163,t1632,t1633,t1635,t1636,t1644,t1645,t1648,t1649,t1650,t1653,t1655,t1657,t1659,t1661,t1662,t1663,t1664,t1665,t1666,t1668,t1669,t1671,t1674,t1678,t1679,t1680,t1681,t1682,t1683,t1684,t1686,t1688,t169,t1690,t1692,t1694,t1695,t1698,t17,t1700,t1703,t1704,t1706,t1707,t1709,t1710,t1711,t1713,t1714,t1715,t1716,t1719,t1726,t1729,t1730,t1733,t1734,t1735,t1736,t1739,t1740,t1741,t1743,t1745,t1749,t1750,t1752,t1753,t1756,t1757,t1759,t176,t1760,t1761,t1762,t1763,t1764,t1765,t1769,t1770,t1771,t1772,t1774,t1775,t1776,t1778,t1779,t1782,t1785,t1786,t1787,t1788,t1789,t1790,t1792,t1793,t1794,t1795,t1796,t1797,t1798,t1799,t1800,t1804,t1806,t1808,t1809,t1811,t1813,t1814,t1815,t1816,t1817,t1818,t1819,t1820,t1822,t1824,t1827,t1828,t1830,t1831,t1832,t1833,t1834,t1835,t1837,t1838,t1839,t1841,t1842,t1843,t1844,t1845,t1846,t1848,t1849,t1850,t1851,t1852,t1853,t1855,t1857,t1858,t1861,t1862,t1863,t1864,t1866,t1867,t1869,t1870,t1871,t1872,t1873,t1874,t1875,t1876,t1878,t1879,t1880,t1881,t1883,t1885,t1886,t1887,t1888,t1890,t1892,t1893,t1894,t1896,t1899,t1900,t1901,t1902,t1903,t1904,t1905,t1906,t1907,t1908,t1910,t1911,t1912,t1913,t1914,t1916,t1918,t1920,t1921,t1922,t1923,t1924,t1926,t1927,t1928,t1929,t1930,t1931,t1932,t1933,t1934,t1938,t1939,t1942,t1943,t1944,t1945,t1946,t1947,t1948,t1950,t1953,t1954,t1955,t1956,t1957,t1958,t1959,t1960,t1961,t1962,t1963,t1964,t1965,t1966,t1967,t1968,t1969,t1972,t1973,t1975,t1976,t1977,t1978,t1981,t1982,t1983,t1984,t1985,t1988,t1989,t199,t1990,t1991,t1994,t1995,t1996,t1997,t1998,t1999,t2,t2001,t2003,t2005,t2006,t2007,t2008,t2009,t2010,t2012,t2016,t2017,t2018,t2022,t2023,t2024,t2025,t2026,t2029,t2030,t2031,t2032,t2033,t2034,t2035,t2036,t2037,t2038,t2039,t2042,t2043,t2045,t2046,t2047,t2048,t2049,t2050,t2051,t2052,t2053,t2054,t2058,t2059,t2060,t2061,t2062,t2063,t2064,t2065,t2066,t2068,t2069,t2070,t2071,t2072,t2074,t2075,t2076,t2077,t2078,t2079,t2080,t2082,t2083,t2086,t2088,t2090,t2093,t2094,t2095,t2097,t2101,t2104,t2105,t2109,t2110,t2111,t2114,t2117,t2118,t2119,t2120,t2121,t2122,t2123,t2124,t2126,t2128,t2129,t2130,t2131,t2132,t2133,t2138,t2141,t2145,t2147,t2148,t2149,t2151,t2152,t2156,t2158,t2160,t2161,t2162,t2163,t2164,t2165,t2166,t2167,t2168,t2171,t2172,t2173,t2175,t2176,t2181,t2184,t2185,t2186,t2187,t2188,t2191,t2192,t2193,t2194,t2195,t2196,t22,t2205,t2206,t2216,t2217,t2218,t2219,t2221,t2224,t2226,t2227,t2228,t2229,t2232,t2233,t2236,t2240,t2241,t2242,t2243,t2244,t2247,t2249,t2250,t2253,t2254,t2264,t2267,t2268,t227,t2276,t2279,t228,t2280,t2282,t2284,t2285,t2289,t2290,t2293,t2302,t2307,t2311,t2315,t2318,t2319,t2320,t2325,t2326,t2333,t2344,t2348,t2349,t2351,t2352,t2353,t2362,t2365,t2367,t2371,t2382,t2387,t2388,t2394,t2400,t2401,t2403,t2406,t2413,t2438,t2442,t2446,t2452,t2454,t2456,t246,t2462,t2466,t2473,t2475,t2476,t2481,t2488,t2498,t2507,t2524,t2525,t2529,t2530,t2531,t2536,t2537,t2543,t2555,t2558,t256,t2560,t2564,t2566,t2571,t2572,t2577,t2582,t2586,t2593,t2597,t2599,t26,t261,t262,t2627,t264,t2655,t2656,t2657,t2658,t2661,t2662,t2663,t2665,t2666,t2667,t2668,t2672,t2680,t27,t274,t276,t28,t288,t289,t29,t290,t291,t292,t293,t294,t295,t296,t298,t299,t3,t30,t300,t301,t307,t31,t314,t32,t33,t330,t34,t341,t344,t346,t35,t351,t354,t359,t36,t361,t362,t366,t37,t38,t386,t388,t389,t39,t395,t396,t398,t399,t4,t40,t400,t401,t402,t403,t404,t405,t406,t407,t411,t418,t419,t421,t422,t43,t432,t433,t435,t437,t441,t442,t444,t445,t450,t451,t459,t461,t464,t473,t475,t476,t477,t478,t479,t480,t481,t482,t483,t493,t494,t495,t496,t499,t5,t501,t502,t506,t508,t509,t51,t512,t514,t518,t522,t524,t525,t526,t527,t528,t53,t530,t531,t532,t533,t536,t54,t544,t545,t546,t547,t548,t55,t551,t554,t555,t556,t557,t56,t564,t565,t568,t569,t570,t571,t572,t573,t574,t583,t584,t586,t588,t589,t59,t591,t592,t594,t595,t596,t6,t600,t601,t605,t606,t607,t608,t609,t612,t614,t616,t621,t622,t623,t624,t626,t627,t628,t637,t638,t640,t641,t642,t647,t649,t65,t650,t652,t654,t655,t656,t658,t659,t66,t660,t661,t662,t664,t665,t666,t668,t669,t67,t671,t676,t677,t678,t679,t680,t682,t683,t684,t686,t689,t69,t690,t691,t692,t694,t696,t699,t7,t700,t701,t702,t703,t704,t707,t708,t709,t71,t710,t711,t712,t713,t714,t715,t717,t72,t720,t721,t722,t725,t726,t729,t73,t732,t733,t734,t735,t737,t739,t740,t741,t742,t743,t744,t745,t746,t75,t751,t758,t759,t760,t764,t765,t767,t768,t770,t771,t773,t774,t775,t776,t777,t778,t781,t782,t783,t784,t788,t790,t792,t798,t8,t801,t802,t803,t811,t812,t815,t816,t818,t819,t821,t822,t823,t825,t826,t829,t842,t843,t853,t854,t864,t865,t868,t869,t872,t879,t880,t883,t884,t885,t895,t896,t897,t899,t9,t902,t905,t911,t913,t914,t916,t919,t921,t922,t924,t933,t937,t938,t939,t943,t944,t947,t948,t949,t953,t954,t960,t961,t962,t963,t964,t965,t966,t967,t968,t969,t971,t972,t973,t974,t975,t977,t980,t982,t983,t984,t990,t991,t994,t995,t996,t998,t999] = ct{:};
t2073 = -t2064;
t2081 = -t2076;
t2084 = t1108+t1459;
t2089 = t1127+t1456;
t2092 = -t2082;
t2098 = -t2086;
t2103 = t12.*t947.*(t67-t512).*1.362083333335e-3;
t2125 = t1411.*t1412.*3.0;
t2135 = t12.*t28.*(t961-t1417).*(-3.9e+1./1.0e+3);
t2140 = -t2126;
t2142 = t12.*t28.*(t961-t1417).*(3.9e+1./1.0e+3);
t2150 = t36.*t39.*(t961-t1417).*(-3.9e+1./1.0e+3);
t2155 = -t2145;
t2159 = t36.*t39.*(t961-t1417).*(3.9e+1./1.0e+3);
t2170 = -t2156;
t2177 = -t2168;
t2183 = t12.*t36.*(t1084+t13.*(t67-t512)).*(-1.6666666666675e-5);
t2200 = -t2191;
t2201 = (t403.*t2029)./2.0;
t2202 = (t770.*t1735)./2.0;
t2203 = (t12.*t36.*t2105)./2.0;
t2209 = t7.*t947.*t948.*1.6666666666675e-5;
t2213 = (t12.*t40.*t2114)./2.0;
t2214 = -t2192;
t2220 = t1396+t1556;
t2231 = t13.*t947.*(t509-t621).*(-1.6666666666675e-5);
t2234 = t1219+t1633;
t2235 = t13.*t947.*(t509-t621).*1.6666666666675e-5;
t2237 = (t947.*t1711)./2.0;
t2239 = t1276+t1632;
t2252 = -t2241;
t2259 = (t947.*t1741)./2.0;
t2262 = t1494+t1544;
t2263 = (t607.*t1991)./1.0e+1;
t2265 = (t295.*t2114)./2.0;
t2273 = t1491+t1557;
t2277 = (t7.*t947.*t1735)./2.0;
t2278 = (t7.*t292.*t2105)./2.0;
t2281 = -t2264;
t2283 = (t404.*t2105)./2.0;
t2292 = t591.*(t961-t1417).*(-1.0./1.0e+1);
t2296 = (t13.*t947.*t1760)./2.0;
t2297 = (t13.*t292.*t2114)./2.0;
t2298 = -t2279;
t2299 = -t2280;
t2305 = (t591.*(t961-t1417))./1.0e+1;
t2306 = (t479.*t2105)./2.0;
t2324 = (t770.*t1918)./2.0;
t2329 = t638.*(t961-t1417).*(-1.0./1.0e+1);
t2330 = -t2315;
t2332 = (t527.*t2114)./2.0;
t2336 = t654.*(t961-t1417).*(-1.0./1.0e+1);
t2342 = (t947.*t1876)./2.0;
t2350 = (t294.*t2205)./2.0;
t2356 = t947.*t1931;
t2358 = -t2352;
t2364 = -t7.*t2105.*(t71-t445);
t2366 = (t589.*t2114)./2.0;
t2374 = (t1339.*t1760)./2.0;
t2375 = -t13.*t2114.*(t71-t445);
t2377 = -t2365;
t2381 = t7.*(t1084+t13.*(t67-t512)).*(t71-t445).*1.6666666666675e-5;
t2383 = (t2105.*(t73-t442))./2.0;
t2385 = (t7.*t947.*t1918)./2.0;
t2389 = t694.*t2105;
t2390 = (t13.*t947.*t1930)./2.0;
t2391 = -t2387;
t2393 = (t1428.*t1735)./2.0;
t2402 = -t2114.*(t113-t554);
t2410 = (t1460.*t1760)./2.0;
t2411 = t947.*(t1159-t1162);
t2420 = t742.*t2114;
t2425 = t770.*t2105;
t2433 = (t1368.*t1930)./2.0;
t2440 = t947.*t2095;
t2445 = (t1428.*t1918)./2.0;
t2448 = t13.*t947.*(t7.*(t67-t512)+t13.*(t444-t642)).*(-3.333333333335e-5);
t2455 = t1006.*t2105;
t2460 = (t1460.*t1930)./2.0;
t2465 = -t2114.*(t441+t13.*(t69-t508));
t2468 = (t7.*t947.*t2105)./2.0;
t2472 = (t294.*t2400)./2.0;
t2474 = (t13.*t947.*t2114)./2.0;
t2480 = (t403.*t2394)./2.0;
t2483 = (t7.*(t160-t1026).*(t961-t1417))./5.0;
t2489 = t1761.*(t1084+t13.*(t67-t512)).*(-1.0./2.0);
t2502 = (t948.*t2205)./2.0;
t2503 = (t1252.*t2105)./2.0;
t2506 = t1828.*(t1084+t13.*(t67-t512)).*(-1.0./2.0);
t2513 = (t1339.*t2114)./2.0;
t2514 = t1519.*(t961-t1417).*(-1.0./5.0);
t2517 = (t1368.*t2114)./2.0;
t2523 = t2105.*(t501-t790).*(-1.0./2.0);
t2527 = (t2105.*(t501-t790))./2.0;
t2528 = (t605.*t2400)./2.0;
t2533 = (t1428.*t2105)./2.0;
t2534 = -t2529;
t2540 = (t2394.*(t75-t518))./2.0;
t2541 = t1907.*(t1084+t13.*(t67-t512)).*(-1.0./2.0);
t2544 = (t1907.*(t1084+t13.*(t67-t512)))./2.0;
t2548 = (t1460.*t2114)./2.0;
t2549 = -t2543;
t2559 = t1988.*(t1084+t13.*(t67-t512)).*(-1.0./2.0);
t2562 = -t2560;
t2563 = t2029.*(t7.*(t67-t512)+t13.*(t444-t642)).*(-1.0./2.0);
t2565 = (t2029.*(t7.*(t67-t512)+t13.*(t444-t642)))./2.0;
t2573 = -t13.*t947.*(t7.*(t67-t512).*3.333333333335e-5+t13.*(t444-t642).*3.333333333335e-5);
t2581 = t1863.*(t961-t1417).*(-1.0./5.0);
t2590 = -t2586;
t2592 = t2129.*(t1084+t13.*(t67-t512)).*(-1.0./2.0);
t2595 = (t2129.*(t1084+t13.*(t67-t512)))./2.0;
t2596 = -t2593;
t2605 = -t1368.*(t7.*(t67-t512).*3.333333333335e-5+t13.*(t444-t642).*3.333333333335e-5);
t2608 = t2205.*(t1084+t13.*(t67-t512));
t2609 = t1339.*(t7.*(t67-t512).*3.333333333335e-5+t13.*(t444-t642).*3.333333333335e-5);
t2620 = t1991.*(t961-t1417).*(-1.0./5.0);
t2622 = -t1460.*(t7.*(t67-t512).*3.333333333335e-5+t13.*(t444-t642).*3.333333333335e-5);
t2626 = -t2394.*(t7.*(t67-t512)+t13.*(t444-t642));
t2628 = -t2400.*(t1084+t13.*(t67-t512));
t2631 = t2160.*(t961-t1417).*(-1.0./1.0e+1);
t2633 = (t2160.*(t961-t1417))./1.0e+1;
t2671 = q_dot3.*(t570-t821-t842-t883+t905+t1650+t1664+t2083+t2088);
t2673 = q_dot4.*t2672;
t2679 = q_dot3.*(-t564-t568+t822+t843+t937+t964+t1080+t1197+t1427+t1458+t1903+t1904+t1913+t1914+t2162+t2163+t2172+t2173);
t1500 = (t5.*t12.*t1386)./2.0;
t1501 = (t6.*t11.*t1386)./2.0;
t1505 = -t1484;
t1525 = (t11.*t39.*t1386)./2.0;
t1623 = t264+t1434;
t1638 = -t1629;
t1640 = (t401.*t1386)./2.0;
t1641 = (t402.*t1386)./2.0;
t1658 = (t478.*t1386)./2.0;
t1660 = (t12.*t399.*t1386)./2.0;
t1725 = (t573.*t1386)./2.0;
t1738 = -t1726;
t1751 = t5.*t6.*(t111.*(2.0./5.0)-t1438).*(-3.9e+1./1.0e+3);
t1758 = (t616.*t1386)./2.0;
t1780 = t11.*t12.*(t111.*(2.0./5.0)-t1438).*(1.17e+2./5.0e+2);
t1783 = -t1757;
t1801 = t11.*t33.*(t111.*(2.0./5.0)-t1438).*(-1.17e+2./5.0e+2);
t1803 = t11.*t34.*(t111.*(2.0./5.0)-t1438).*(-3.9e+1./1.0e+3);
t1812 = -t1786;
t1823 = -t1386.*(t111-t536);
t1825 = t11.*t33.*(t111.*(2.0./5.0)-t1438).*(1.17e+2./5.0e+2);
t1829 = t12.*t1386.*(t67-t512);
t1860 = t764+t1295;
t1909 = -t1899;
t1917 = t1386.*(t499-t506);
t1992 = -t1981;
t1993 = -t1983;
t2000 = t1005.*t1386;
t2013 = t13.*t592.*(t111.*(2.0./5.0)-t1438).*(-1.0./1.0e+1);
t2019 = t7.*t607.*(t111.*(2.0./5.0)-t1438).*(-1.0./1.0e+1);
t2020 = (t13.*t592.*(t111.*(2.0./5.0)-t1438))./1.0e+1;
t2055 = t13.*t655.*(t111.*(2.0./5.0)-t1438).*(-1.0./1.0e+1);
t2106 = (t111.*(2.0./5.0)-t1438).*(t151+t12.*(t157-t10.*t38.*(3.9e+1./1.0e+2))).*(3.0./5.0);
t2112 = t12.*t35.*t1990.*(3.9e+1./1.0e+3);
t2136 = t39.*t40.*t1990.*(3.9e+1./1.0e+3);
t2139 = (t5.*t12.*t2084)./2.0;
t2146 = t12.*t864.*(t111.*(2.0./5.0)-t1438).*(-3.0./5.0);
t2153 = (t5.*t6.*t2089)./2.0;
t2157 = t12.*t864.*(t111.*(2.0./5.0)-t1438).*(3.0./5.0);
t2169 = (t11.*t39.*t2084)./2.0;
t2174 = (t640.*t1848)./1.0e+1;
t2178 = (t11.*t34.*t2089)./2.0;
t2189 = t1440+t1483;
t2190 = (t294.*t2039)./2.0;
t2210 = -t2201;
t2211 = -t2202;
t2212 = -t2203;
t2222 = t1082.*(t111.*(2.0./5.0)-t1438).*(6.0./5.0);
t2223 = -t2209;
t2225 = -t2213;
t2238 = (t293.*t2089)./2.0;
t2245 = -t2237;
t2248 = (t402.*t2084)./2.0;
t2258 = (t478.*t2084)./2.0;
t2260 = (t12.*t399.*t2084)./2.0;
t2266 = (t6.*t399.*t2089)./2.0;
t2272 = (t111.*(2.0./5.0)-t1438).*(t169-t960).*(3.0./5.0);
t2274 = (t606.*t1990)./1.0e+1;
t2275 = -t2263;
t2288 = t1433+t1622;
t2294 = -t2277;
t2295 = -t2278;
t2300 = -t2283;
t2301 = (t526.*t2089)./2.0;
t2304 = t1376.*(t111.*(2.0./5.0)-t1438).*(-1.0./1.0e+1);
t2308 = -t2297;
t2312 = t1467+t1624;
t2314 = (t1376.*(t111.*(2.0./5.0)-t1438))./1.0e+1;
t2316 = (t641.*t1990)./1.0e+1;
t2317 = (t605.*t2039)./2.0;
t2321 = (t1990.*(t307-t411))./1.0e+1;
t2335 = t12.*t1411.*(t111.*(2.0./5.0)-t1438).*(6.0./5.0);
t2343 = (t616.*t2084)./2.0;
t2346 = -t2342;
t2357 = t664.*t2089;
t2361 = t12.*t2084.*(t67-t512);
t2363 = t2089.*(t69-t508).*(-1.0./2.0);
t2368 = -t2084.*(t111-t536);
t2369 = t6.*t2089.*(t67-t512);
t2370 = (t111.*(2.0./5.0)-t1438).*(t1229+t8.*t56.*(2.0./5.0)).*(6.0./5.0);
t2372 = (t2089.*(t69-t508))./2.0;
t2373 = (t403.*t2220)./2.0;
t2378 = -t2366;
t2384 = -t2381;
t2392 = (t294.*t2262)./2.0;
t2396 = -t2393;
t2398 = t741.*t2089;
t2405 = t1594.*(t111.*(2.0./5.0)-t1438).*(6.0./5.0);
t2409 = (t403.*t2273)./2.0;
t2414 = t1517+t1743;
t2416 = -t2410;
t2417 = t2084.*(t499-t506);
t2419 = t948.*t2039;
t2432 = (t605.*t2239)./2.0;
t2436 = -t2433;
t2437 = t2234.*(t75-t518).*(-1.0./2.0);
t2439 = t1005.*t2084;
t2441 = (t2234.*(t75-t518))./2.0;
t2444 = (t605.*t2262)./2.0;
t2453 = -t2089.*(t514+t6.*(t65-t437));
t2470 = t13.*t1990.*(t160-t1026).*(-1.0./5.0);
t2471 = -t2468;
t2482 = -t2474;
t2508 = -t2502;
t2509 = -t2503;
t2512 = t2220.*(t509-t621).*(-1.0./2.0);
t2515 = t1990.*(t624-t818).*(-1.0./5.0);
t2516 = (t948.*t2239)./2.0;
t2518 = (t2220.*(t509-t621))./2.0;
t2519 = -t2513;
t2521 = -t2517;
t2522 = t2234.*(t509-t621).*(-1.0./2.0);
t2526 = (t2234.*(t509-t621))./2.0;
t2532 = (t948.*t2262)./2.0;
t2539 = -t2533;
t2547 = t2273.*(t509-t621).*(-1.0./2.0);
t2551 = (t2273.*(t509-t621))./2.0;
t2552 = -t2548;
t2553 = t13.*t1990.*(t111.*(2.0./5.0)-t1438).*(-1.0./1.0e+1);
t2554 = (t13.*t1990.*(t111.*(2.0./5.0)-t1438))./1.0e+1;
t2557 = (t7.*(t111.*(2.0./5.0)-t1438).*(t961-t1417))./1.0e+1;
t2567 = t2039.*(t1084+t13.*(t67-t512)).*(-1.0./2.0);
t2569 = (t2039.*(t1084+t13.*(t67-t512)))./2.0;
t2578 = t1848.*(t961-t1417).*(-1.0./1.0e+1);
t2604 = -t2234.*(t7.*(t67-t512)+t13.*(t444-t642));
t2606 = t2220.*(t7.*(t67-t512)+t13.*(t444-t642));
t2615 = t2239.*(t1084+t13.*(t67-t512));
t2617 = -t2273.*(t7.*(t67-t512)+t13.*(t444-t642));
t2619 = t1990.*(t1023-t1387).*(-1.0./5.0);
t2621 = -t2262.*(t1084+t13.*(t67-t512));
t2630 = (t1990.*t2181)./1.0e+1;
t1647 = -t1641;
t1651 = t7.*t1623;
t1652 = t13.*t1623;
t1670 = -t1660;
t1724 = t6.*t11.*t1623.*(3.9e+1./2.0e+2);
t1732 = t5.*t12.*t1623.*(3.9e+1./1.0e+3);
t1737 = -t1725;
t1746 = t11.*t27.*t1623.*(3.9e+1./2.0e+2);
t1747 = t59.*t1623.*(3.9e+1./2.0e+2);
t1777 = t11.*t39.*t1623.*(3.9e+1./1.0e+3);
t1784 = -t1758;
t2091 = (t778.*t1623)./2.0;
t2115 = -t2106;
t2127 = -t2112;
t2143 = -t2136;
t2144 = (t6.*t864.*t1623)./2.0;
t2180 = t1095.*t1623;
t2182 = -t2174;
t2199 = -t2190;
t2204 = (t655.*t1860)./1.0e+1;
t2208 = t1436+t1505;
t2246 = -t2238;
t2255 = -t2248;
t2256 = (t1275.*t1623)./2.0;
t2269 = -t2260;
t2286 = t6.*t1411.*t1623;
t2287 = -t2266;
t2291 = -t2272;
t2303 = t1623.*(t160-t1026).*(-1.0./1.0e+1);
t2310 = -t2301;
t2313 = (t1623.*(t160-t1026))./1.0e+1;
t2328 = -t2321;
t2347 = -t2343;
t2355 = t1623.*(t256+t6.*(t176+t314+t459+t26.*t30.*(2.0./5.0)));
t2376 = t1579.*t1623;
t2395 = -t2392;
t2415 = -t2409;
t2423 = (t607.*t2189)./1.0e+1;
t2431 = (t640.*t2189)./1.0e+1;
t2435 = -t2432;
t2449 = (t12.*t36.*t2414)./2.0;
t2461 = (t607.*t2288)./1.0e+1;
t2464 = (t592.*t2312)./1.0e+1;
t2469 = (t640.*t2288)./1.0e+1;
t2487 = (t655.*t2312)./1.0e+1;
t2490 = (t404.*t2414)./2.0;
t2493 = (t7.*t292.*t2414)./2.0;
t2499 = (t479.*t2414)./2.0;
t2520 = -t2516;
t2538 = -t2532;
t2542 = t2414.*(t73-t442).*(-1.0./2.0);
t2545 = (t2414.*(t73-t442))./2.0;
t2546 = t7.*t2414.*(t71-t445).*(-1.0./2.0);
t2550 = (t7.*t2414.*(t71-t445))./2.0;
t2556 = (t694.*t2414)./2.0;
t2561 = -t2557;
t2568 = (t770.*t2414)./2.0;
t2574 = t7.*t947.*t2414;
t2579 = (t1860.*t1990)./1.0e+1;
t2587 = (t1006.*t2414)./2.0;
t2601 = t1252.*t2414;
t2616 = t2414.*(t501-t790);
t2618 = t1428.*t2414;
t2629 = t1683.*t2414;
t2632 = -t2630;
t2637 = t2189.*(t961-t1417).*(-1.0./1.0e+1);
t2639 = (t2189.*(t961-t1417))./1.0e+1;
t2676 = t1477+t1487+t2025+t2042+t2128+t2364+t2375+t2470+t2483;
t2684 = t751+t781+t971+t983+t1002+t1552+t1565+t1649+t1674+t1790+t1811+t1837+t1843+t2101+t2112+t2119+t2135+t2203+t2213;
t2688 = t916+t977+t1202+t1203+t1373+t1374+t1577+t1606+t1835+t1850+t1853+t1874+t1910+t1932+t2136+t2150+t2224+t2233+t2295+t2308;
t2697 = -q_dot2.*(t782+t801-t1420-t1636-t1745-t1879-t1893+t1901+t1908+t1911+t1953+t1998-t2033-t2046+t2419-t2420+t2425+t2581+t2029.*(t509-t621)+(t1990.*(t1020-t1024))./5.0+t12.*t399.*(t71-t445).*1.362083333335e-3+t12.*t399.*(t386-t572));
t2698 = t422+t628+t696+t700+t771+t1031+t1065+t1225+t1359+t1367+t1390+t1424+t1521+t1792+t1820+t1841+t1886+t1939+t2043+t2058+t2069+t2078+t2388+t2389+t2401+t2402+t2514+t2515;
t2703 = t666+t682+t746+t783+t788+t802+t914+t938+t963+t1132+t1181+t1215+t1473+t1485+t1541+t1769+t1880+t1894+t1902+t1912+t2026+t2070+t2104+t2123+t2124+t2132+t2133+t2455+t2456+t2465+t2466+t2619+t2620;
t2709 = -q_dot2.*(t418+t476+t677+t692-t725-t872-t1102+t1168-t1200+t1208+t1242+t1264+t1312-t1322-t1364-t1404+t1466-t1475-t1480+t1520+t1555-t1730-t1749+t1771+t1800-t1946-t1960-t2161+t2190+t2191+t2201+t2202+t2264-t2265-t2274+t2283+t2292+(t592.*(t1020-t1024))./1.0e+1+(t1736.*(t509-t621))./2.0+t5.*t12.*(t71-t445).*6.810416666674999e-4+(t5.*t12.*(t386-t572))./2.0);
t1667 = -t1651;
t1731 = -t1724;
t1773 = -t1746;
t2100 = -t2091;
t2154 = -t2144;
t2198 = -t2180;
t2215 = -t2204;
t2261 = -t2256;
t2309 = -t2286;
t2331 = t1435+t1652;
t2386 = -t2376;
t2426 = (t592.*t2208)./1.0e+1;
t2443 = (t655.*t2208)./1.0e+1;
t2463 = -t2461;
t2491 = -t2487;
t2570 = -t2568;
t2585 = -t2579;
t2591 = -t2587;
t2607 = -t2601;
t2636 = (t1990.*t2208)./1.0e+1;
t2677 = q_dot2.*t2676;
t2685 = t740+t765+t944+t968+t983+t1535+t1550+t1653+t1663+t1816+t1830+t1834+t1845+t2109+t2110+t2127+t2142+t2212+t2225;
t2687 = t916+t977+t1258+t1259+t1347+t1349+t1566+t1589+t1844+t1858+t1861+t1862+t1900+t1922+t2143+t2159+t2232+t2236+t2278+t2297;
t2689 = q_dot2.*t2688;
t2699 = q_dot2.*t2698;
t2704 = q_dot2.*t2703;
t2707 = t418+t476+t689+t704+t725+t872+t967+t1102+t1168+t1200+t1208+t1242+t1309+t1322+t1351+t1364+t1404+t1475+t1480+t1482+t1534+t1567+t1603+t1730+t1749+t1796+t1824+t1946+t1960+t2161+t2171+t2199+t2200+t2210+t2211+t2265+t2274+t2281+t2282+t2300+t2305;
t2725 = t140+t228+t614+t627+t678+t683+t701+t710+t713+t734+t868+t899+t953+t954+t1003+t1007+t1014+t1037+t1038+t1099+t1104+t1147+t1160+t1184+t1246+t1249+t1328+t1334+t1348+t1350+t1416+t1446+t1495+t1522+t1528+t1563+t1587+t1604+t1657+t1750+t1772+t1793+t1838+t1942+t1963+t1964+t1968+t1973+t1982+t1996+t1997+t2037+t2038+t2065+t2066+t2249+t2250+t2275+t2276+t2279+t2280+t2284+t2285+t2325+t2326+t2328+t2329+t2377+t2378+t2382+t2383;
t2340 = t1439+t1667;
t2412 = t12.*t35.*t2331.*(3.9e+1./1.0e+3);
t2422 = t39.*t40.*t2331.*(3.9e+1./1.0e+3);
t2477 = (t606.*t2331)./1.0e+1;
t2492 = (t641.*t2331)./1.0e+1;
t2495 = (t2331.*(t307-t411))./1.0e+1;
t2584 = t13.*t2331.*(t160-t1026).*(-1.0./1.0e+1);
t2589 = (t13.*t2331.*(t160-t1026))./1.0e+1;
t2613 = t2331.*(t624-t818).*(-1.0./1.0e+1);
t2614 = (t2331.*(t624-t818))./1.0e+1;
t2623 = t13.*t2331.*(t111.*(2.0./5.0)-t1438).*(-1.0./5.0);
t2635 = (t1860.*t2331)./5.0;
t2638 = -t2636;
t2641 = t2331.*(t1020-t1024).*(-1.0./1.0e+1);
t2643 = (t2331.*(t1020-t1024))./1.0e+1;
t2645 = t2331.*(t1023-t1387).*(-1.0./1.0e+1);
t2647 = (t2331.*(t1023-t1387))./1.0e+1;
t2649 = (t2181.*t2331)./5.0;
t2651 = (t2208.*t2331)./5.0;
t2653 = (t2312.*t2331)./5.0;
t2686 = q_dot2.*t2685;
t2726 = q_dot2.*t2725;
t2418 = -t2412;
t2421 = t12.*t28.*t2340.*(3.9e+1./1.0e+3);
t2428 = t36.*t39.*t2340.*(3.9e+1./1.0e+3);
t2484 = (t591.*t2340)./1.0e+1;
t2496 = -t2495;
t2497 = (t638.*t2340)./1.0e+1;
t2501 = (t654.*t2340)./1.0e+1;
t2594 = t7.*t2340.*(t160-t1026).*(-1.0./1.0e+1);
t2598 = (t7.*t2340.*(t160-t1026))./1.0e+1;
t2612 = (t1519.*t2340)./1.0e+1;
t2634 = (t1848.*t2340)./5.0;
t2640 = (t1863.*t2340)./1.0e+1;
t2644 = (t1991.*t2340)./1.0e+1;
t2648 = (t2160.*t2340)./5.0;
t2650 = (t2189.*t2340)./5.0;
t2652 = (t2288.*t2340)./5.0;
t2654 = -t2653;
t2683 = q_dot1.*(t2448+t2573-t2574+t2623+t947.*(t571-t729)+t1386.*(t444-t642)+(t1623.*(t111.*(2.0./5.0)-t1438))./5.0+(t7.*t2340.*(t111.*(2.0./5.0)-t1438))./5.0+t7.*t947.*(t1084+t13.*(t67-t512)).*3.333333333335e-5);
t2500 = -t2497;
t2642 = -t2640;
t2646 = -t2644;
t2690 = t975+t1048+t1363+t1402+t1501+t1509+t1732+t1751+t1909+t1921+t2019+t2020+t2175+t2183+t2294+t2296+t2418+t2421+t2449+t2452;
t2692 = -q_dot1.*(t975+t1048-t1363-t1501-t1732+t1899-t1921+t2013+t2164+t2277-t2296+t2412-t2421+t2446-t2449+t5.*t6.*(t111.*(2.0./5.0)-t1438).*(3.9e+1./1.0e+3)+(t7.*t607.*(t111.*(2.0./5.0)-t1438))./1.0e+1+t12.*t36.*(t1084+t13.*(t67-t512)).*1.6666666666675e-5+t11.*t12.*(t444-t642).*3.0e-5+(t11.*t12.*(t571-t729))./2.0);
t2695 = -q_dot1.*(t974+t1068+t1628+t1640+t1777+t1803-t2024+t2055+t2240-t2385-t2390-t2422+t2428+t2488-t2493+(t292.*(t571-t729))./2.0+(t622.*(t444-t642))./2.0+(t7.*t640.*(t111.*(2.0./5.0)-t1438))./1.0e+1+t7.*t292.*(t1084+t13.*(t67-t512)).*1.6666666666675e-5+t13.*t947.*(t75-t518).*1.6666666666675e-5);
t2700 = t973+t982+t1041+t1737+t1738+t1812+t1813+t2209+t2231+t2313+t2314+t2352+t2384+t2468+t2474+t2543+t2550+t2553+t2557+t2584+t2598;
t2701 = t973+t982+t1041+t1725+t1726+t1786+t1787+t2223+t2235+t2303+t2304+t2358+t2381+t2471+t2482+t2546+t2549+t2554+t2561+t2589+t2594;
t2705 = t1476+t1486+t1779+t1829+t2068+t2103+t2125+t2140+t2141+t2148+t2149+t2309+t2335+t2353+t2361+t2369+t2617+t2618+t2621+t2622+t2650+t2651;
t2714 = q_dot1.*(-t703-t885+t1198+t1325+t1361+t1448+t1612+t1625+t1706+t1707+t1871+t1885+t1887+t1896+t1905+t1906+t1917+t2022+t2045+t2198+t2222+t2344+t2398+t2403+t2411+t2417+t2604+t2605+t2615+t2616+t2634+t2635);
t2715 = t366+t650+t665+t854+t1062+t1074+t1222+t1237+t1244+t1316+t1405+t1406+t1414+t1560+t1613+t1782+t1785+t1798+t1799+t1823+t2030+t2031+t2032+t2097+t2098+t2355+t2356+t2357+t2367+t2368+t2370+t2391+t2606+t2607+t2608+t2609+t2648+t2649;
t2717 = t461+t495+t532+t911+t913+t1050+t1209+t1230+t1261+t1270+t1298+t1323+t1329+t1500+t1518+t1536+t1554+t1561+t1595+t1596+t1611+t1648+t1731+t1759+t1780+t1846+t1852+t1927+t1950+t1961+t1962+t2139+t2153+t2395+t2396+t2415+t2416+t2423+t2426+t2475+t2476+t2477+t2484+t2489+t2490;
t2724 = q_dot1.*(-t649+t668+t880+t984+t1053+t1131+t1217+t1283+t1327+t1442+t1450+t1471+t1472+t1583+t1605+t1713+t1869+t1872+t1873+t1883+t1888+t2000+t2001+t2111+t2118+t2121+t2122+t2131+t2386+t2405+t2439+t2440+t2453+t2454+t2462+t2626+t2627+t2628+t2629+t2652+t2654);
t2728 = t359+t450+t475+t493+t531+t1166+t1206+t1241+t1256+t1285+t1299+t1302+t1305+t1320+t1342+t1346+t1582+t1617+t1618+t1660+t1831+t1928+t1929+t1981+t1983+t2008+t2034+t2049+t2051+t2059+t2063+t2071+t2074+t2081+t2092+t2154+t2155+t2157+t2158+t2192+t2195+t2206+t2260+t2266+t2538+t2539+t2547+t2548+t2563+t2564+t2567+t2568+t2636+t2639+t2640+t2641;
t2733 = q_dot1.*(t262+t389+t679+t732+t744+t759+t816+t922-t939+t965+t998+t1033+t1051+t1057+t1124+t1201+t1233+t1330+t1388+t1400+t1409+t1437+t1451+t1453+t1492+t1523+t1538+t1553+t1573+t1597+t1602+t1638+t1647+t1655+t1662+t1665+t1666+t1739+t1756+t1762+t1773+t1778+t1819+t1825+t1851+t1945+t1976+t2006+t2016+t2023+t2165+t2166+t2174+t2176+t2177+t2204+t2238+t2245+t2247+t2255+t2350+t2351+t2373+t2374+t2406+t2413+t2435+t2436+t2441+t2442+t2495+t2497+t2524+t2525+t2544+t2545+t4.*t1329);
t2735 = t261+t276+t362+t480+t717+t773+t819+t865+t869+t895+t902+t921+t1045+t1055+t1093+t1142+t1277+t1310+t1358+t1389+t1391+t1470+t1481+t1513+t1514+t1539+t1547+t1549+t1562+t1571+t1626+t1658+t1659+t1668+t1669+t1690+t1698+t1716+t1734+t1776+t1814+t1815+t1817+t1827+t1833+t1870+t1924+t1926+t1933+t1957+t1965+t1999+t2053+t2054+t2077+t2100+t2115+t2130+t2170+t2187+t2252+t2253+t2258+t2259+t2267+t2268+t2310+t2311+t2463+t2464+t2472+t2473+t2480+t2481+t2520+t2521+t2526+t2527+t2556+t2558+t2559+t2562+t2578+t2585+t2612+t2614;
et1 = t261+t276+t362-t480-t717+t758+t811+t819+t829-t895+t921-t1055+t1071+t1096+t1265+t1277-t1358-t1389-t1391+t1463+t1470+t1512+t1513-t1514+t1539+t1549-t1562-t1571-t1658-t1659-t1668-t1669+t1680+t1698+t1716-t1734-t1776+t1788+t1806-t1815+t1817+t1833+t1870+t1923+t1924+t1926-t1965-t1999-t2053-t2077+t2091+t2106-t2130+t2170+t2187+t2241+t2242-t2258-t2259-t2267+t2301+t2302+t2463+t2464+t2472+t2473+t2480+t2481+t2516+t2517+t2522+t2523+t2555-t2556+t2560+t2579-t2612+t2613+(t1988.*(t1084+t13.*(t67-t512)))./2.0+t1082.*(t160-t1026).*(3.0./5.0)+(t1866.*(t499-t506))./2.0;
et2 = (t1848.*(t961-t1417))./1.0e+1-(t11.*t288.*t609)./2.0-(t11.*t288.*t1709)./2.0+t10.*t38.*(t67-t512).*1.4010416666675e-3+(t10.*t38.*(t344-t584))./2.0;
t2737 = -q_dot1.*(et1+et2);
t2738 = t351+t473+t652+t684+t737+t760+t774+t776+t777+t803+t826+t884+t897+t949+t962+t972+t1004+t1056+t1060+t1061+t1075+t1077+t1092+t1097+t1100+t1144+t1218+t1257+t1303+t1318+t1369+t1378+t1382+t1407+t1423+t1493+t1531+t1546+t1558+t1590+t1591+t1592+t1593+t1644+t1645+t1692+t1715+t1729+t1740+t1753+t1783+t1784+t1804+t1809+t1878+t1934+t1943+t1944+t1947+t1958+t1994+t1995+t2007+t2048+t2061+t2064+t2075+t2120+t2184+t2185+t2216+t2217+t2228+t2229+t2243+t2244+t2261+t2289+t2290+t2291+t2315+t2346+t2347+t2371+t2372+t2469+t2491+t2502+t2503+t2518+t2519+t2528+t2534+t2536+t2540+t2587+t2590+t2592+t2596+t2630+t2633+t2644+t2647;
t2702 = q_dot1.*t2700;
t2706 = q_dot1.*t2705;
t2716 = q_dot1.*t2715;
t2718 = q_dot1.*t2717;
t2729 = q_dot1.*t2728;
t2730 = t359+t450+t475+t493+t531+t1166+t1206+t1241+t1255+t1285+t1300+t1304+t1305+t1320+t1342+t1344+t1568+t1585+t1635+t1670+t1808+t1916+t1938+t1992+t1993+t2018+t2036+t2047+t2050+t2060+t2062+t2072+t2076+t2079+t2082+t2144+t2145+t2146+t2147+t2186+t2196+t2214+t2269+t2287+t2532+t2533+t2551+t2552+t2565+t2566+t2569+t2570+t2637+t2638+t2642+t2643;
t2732 = t262+t432+t691+t732+t735+t775+t792+t922+t939+t991+t1000+t1032+t1039+t1051+t1124+t1233+t1250+t1289+t1362+t1399+t1400+t1421+t1437+t1474+t1478+t1504+t1508+t1524+t1553+t1584+t1597+t1615+t1629+t1641+t1655+t1665+t1666+t1684+t1733+t1746+t1752+t1763+t1789+t1801+t1819+t1851+t1956+t1985+t2006+t2012+t2016+t2151+t2152+t2167+t2168+t2182+t2215+t2237+t2246+t2248+t2254+t2350+t2351+t2373+t2374+t2406+t2413+t2432+t2433+t2437+t2438+t2496+t2500+t2530+t2531+t2541+t2542;
t2734 = -t2733;
t2739 = q_dot1.*t2738;
t2741 = t433+t473+t637+t669+t726+t745+t776+t777+t812+t815+t853+t884+t897+t969+t980+t990+t1008+t1054+t1056+t1072+t1075+t1078+t1079+t1092+t1118+t1143+t1274+t1301+t1318+t1345+t1355+t1369+t1398+t1426+t1432+t1493+t1503+t1546+t1558+t1576+t1608+t1609+t1619+t1644+t1645+t1714+t1715+t1729+t1740+t1753+t1757+t1758+t1775+t1832+t1892+t1934+t1947+t1954+t1955+t1958+t2009+t2010+t2017+t2035+t2052+t2073+t2080+t2138+t2193+t2194+t2218+t2219+t2226+t2227+t2243+t2244+t2256+t2272+t2289+t2290+t2330+t2342+t2343+t2362+t2363+t2469+t2491+t2508+t2509+t2512+t2513+t2528+t2534+t2536+t2540+t2586+t2591+t2593+t2595+t2631+t2632+t2645+t2646;
t2740 = -t2739;
et3 = t8.*1.68e-2+t1857.*(t514+t6.*(t65-t437))+t864.*(t246+t330-t556-t2.*t26.*(2.0./5.0)).*3.0-t3.*t8.*7.8e-3-t3.*t546.*(2.3e+1./2.5e+1)-t3.*t601-t398.*t600+t399.*t739-t482.*t676.*2.0+t2.*t1181-t502.*t686.*2.0+t588.*t609+t626.*t823.*2.0+t3.*t1502-t712.*t996.*2.0-t290.*t1849+t399.*t1855+t588.*t1709-t1005.*t1866+t1247.*t1679.*2.0+t1376.*t1579+t948.*t2400-t1661.*t2114+t1683.*t2105+(t1990.*t2312)./5.0+t573.*(t1174+t6.*(t65-t437).*1.302083333335e-3)+t1418.*(t71-t445);
et4 = t1005.*(t386-t572)+t1671.*(t65-t437)+t2095.*(t71-t445)-t1594.*(t160-t1026).*(6.0./5.0)+t2394.*(t509-t621)-(t2288.*(t961-t1417))./5.0-t2.*t3.*t9.*5.065666666667e-1-t4.*t9.*t289.*1.533333333335e-2+t9.*t10.*t398.*2.080133333335e-2-t9.*t10.*t825-t4.*t9.*t1678+t9.*t10.*t1688;
et5 = t29.*(-1.68e-2)+t51.*1.68e-2-t9.*t37.*(7.0./1.25e+2)-t5.*t1394.*(3.9e+1./5.0e+1)+(t592.*t1860)./5.0+(t607.*t1848)./5.0+t294.*t2239-t403.*t2234-t1368.*t1760-t11.*(t163-t557).*(3.1e+1./1.25e+2)-t1735.*(t501-t790)+t11.*(t555-t37.*t38.*(2.0./5.0)).*(1.17e+2./1.0e+2)+t5.*t11.*t288.*3.779850000003e-2+t6.*t11.*t741.*1.302083333335e-3;
et6 = t5.*t12.*t1082.*(-1.17e+2./2.5e+2)-t5.*t6.*t1095.*(3.9e+1./1.0e+2)+t6.*t11.*t1989+t11.*t12.*(t499-t506).*1.362083333335e-3+t11.*t12.*(t595-t596)+t11.*t12.*(t1159-t1162);
et7 = t421-t3.*t8.*1.352e-1-t10.*t545.*(7.0./5.0e+1)-t10.*t548.*(3.0./2.5e+1)-t4.*t647-t4.*t699.*(3.0./2.5e+1)+t547.*t1469.*2.0-t292.*t1931+t401.*t1920+t664.*t1710-(t640.*t2160)./5.0+t605.*t2205-(t655.*t2181)./5.0+t1252.*t1918-t1339.*t1930+t622.*(t111-t536)+t292.*(t464-t623)+t1695.*(t111-t536)+t2220.*(t75-t518)-t11.*t39.*(t1229+t8.*t56.*(2.0./5.0)).*(1.17e+2./2.5e+2)+t9.*t10.*t30.*1.603599999999999e-2;
et8 = t5.*t10.*t477.*(-2.170133333335e-2)+t10.*t11.*t525.*2.802083333335e-3+t10.*t11.*t656-t5.*t10.*t784.*(3.1e+1./1.25e+2)-t5.*t10.*t1088.*(1.17e+2./1.0e+2)-t5.*t10.*t1719+t10.*t11.*t1764+t11.*t34.*(t256+t6.*(t176+t314+t459+t26.*t30.*(2.0./5.0))).*(3.9e+1./1.0e+2);
et9 = t346+t483+t522+t533+t943+t966+t1240+t1314+t1324+t1352-t1525+t1574-t1575-t1578+t1610+t1621+t1681+t1682-t1747-t1867+t1881-t1948-t1959+t1969+t1977+t2090-t2169-t2178+t2431+t2443+t2444+t2445-t2460-t2492+t2498+t2499-t2501+t2506+t2507+(t2273.*(t75-t518))./2.0+t72.*(t111.*(2.0./5.0)-t1438).*(1.17e+2./5.0e+2)-t10.*t11.*t1044.*(3.1e+1./2.5e+2)+t5.*t10.*(t67-t512).*9.4496250000075e-3;
et10 = t12.*t292.*(t67-t512).*6.810416666674999e-4+t5.*t104.*(t341-t583)+t11.*t34.*(t444-t642).*6.510416666674999e-4+(t12.*t622.*(t67-t512))./2.0+(t12.*t1695.*(t67-t512))./2.0;
et11 = t346+t483+t522+t533+t943+t966+t1240+t1314+t1324+t1352-t1525+t1574-t1575-t1578+t1610+t1621+t1681+t1682-t1747-t1867+t1881-t1948-t1959+t1969+t1977+t2090-t2169-t2178+t2431+t2443+t2444+t2445-t2460-t2492+t2498+t2499-t2501+t2506+t2507+(t2273.*(t75-t518))./2.0+t72.*(t111.*(2.0./5.0)-t1438).*(1.17e+2./5.0e+2)-t10.*t11.*t1044.*(3.1e+1./2.5e+2)+t5.*t10.*(t67-t512).*9.4496250000075e-3;
et12 = t12.*t292.*(t67-t512).*6.810416666674999e-4+t5.*t104.*(t341-t583)+t11.*t34.*(t444-t642).*6.510416666674999e-4+(t12.*t622.*(t67-t512))./2.0+(t12.*t1695.*(t67-t512))./2.0;
et13 = t1157+t2706-q_dot6.*t2667-q_dot2.*t2730-q_dot4.*(-t461-t495-t532+t911+t913+t1050+t1165+t1205+t1279+t1306+t1329+t1343+t1356+t1500+t1518+t1536+t1554+t1561+t1595+t1596+t1611+t1648+t1731+t1759+t1780+t1846+t1852+t1927+t1950+t1961+t1962+t2139+t2153+t2395+t2396+t2415+t2416+t2423+t2426+t2475+t2476+t2477+t2484+t2489+t2490);
et14 = q_dot5.*(t43.*9.672e-2-t53.*(6.2e+1./6.25e+2)+t110.*(6.2e+1./6.25e+2)+t5.*t29.*9.672e-2-t26.*t30.*9.672e-2+t66.*t1101+t6.*t12.*t67.*5.33333333333e-5-t6.*t11.*t12.*t29.*5.33333333333e-5)+q_dot3.*(et11+et12);
et15 = -q_dot2.*(-t649+t668+t880+t984+t1053+t1131+t1217+t1283+t1327+t1442+t1450+t1471+t1472+t1583+t1605+t1713+t1869+t1872+t1873+t1883+t1888+t2000+t2001+t2111+t2118+t2121+t2122+t2131+t2386+t2405+t2439+t2440+t2453+t2454+t2462+t2626+t2627+t2628+t2629+t2652+t2654)+q_dot5.*t2705+q_dot3.*t2715+q_dot4.*(-t703-t885+t1198+t1325+t1361+t1448+t1612+t1625+t1706+t1707+t1871+t1885+t1887+t1896+t1905+t1906+t1917+t2022+t2045+t2198+t2222+t2344+t2398+t2403+t2411+t2417+t2604+t2605+t2615+t2616+t2634+t2635);
et16 = -q_dot6.*(t2448+t2573-t2574+t2623+t947.*(t571-t729)+t1386.*(t444-t642)+(t1623.*(t111.*(2.0./5.0)-t1438))./5.0+(t7.*t2340.*(t111.*(2.0./5.0)-t1438))./5.0+t7.*t947.*(t1084+t13.*(t67-t512)).*3.333333333335e-5);
et17 = -q_dot2.*(t1704+t2724-q_dot6.*t2701+q_dot5.*t2730+q_dot4.*t2735+q_dot3.*t2741-q_dot2.*(et3+et4))+q_dot7.*t2656-q_dot4.*(-t1498-t2714+q_dot4.*(et5+et6)+q_dot6.*t2690+q_dot3.*t2732+q_dot2.*t2735+q_dot5.*(-t461-t495-t532+t911+t913+t1050+t1165+t1205+t1279+t1306+t1329+t1343+t1356+t1500+t1518+t1536+t1554+t1561+t1595+t1596+t1611+t1648+t1731+t1759+t1780+t1846+t1852+t1927+t1950+t1961+t1962+t2139+t2153+t2395+t2396+t2415+t2416+t2423+t2426+t2475+t2476+t2477+t2484+t2489+t2490));
et18 = -q_dot6.*(t1703+t2683+q_dot5.*t2667+q_dot4.*t2690-q_dot2.*t2701+q_dot3.*(t1009+t1049+t1628+t1640+t1777+t1803-t2024+t2055+t2240-t2385-t2390-t2422+t2428+t2488-t2493+(t292.*(t571-t729))./2.0+(t622.*(t444-t642))./2.0+(t7.*t640.*(t111.*(2.0./5.0)-t1438))./1.0e+1+t7.*t292.*(t1084+t13.*(t67-t512)).*1.6666666666675e-5+t13.*t947.*(t75-t518).*1.6666666666675e-5));
et19 = -q_dot3.*(-t1156-t2716+q_dot4.*t2732+q_dot2.*t2741+q_dot6.*(t1009+t1049+t1628+t1640+t1777+t1803-t2024+t2055+t2240-t2385-t2390-t2422+t2428+t2488-t2493+(t292.*(t571-t729))./2.0+(t622.*(t444-t642))./2.0+(t7.*t640.*(t111.*(2.0./5.0)-t1438))./1.0e+1+t7.*t292.*(t1084+t13.*(t67-t512)).*1.6666666666675e-5+t13.*t947.*(t75-t518).*1.6666666666675e-5)+q_dot3.*(et7+et8)-q_dot5.*(et9+et10));
et20 = q_dot5.*(et13+et14)+q_dot1.*(et15+et16);
et21 = t261+t276+t362-t480-t717+t758+t811+t819+t829-t895+t921-t1055+t1071+t1096+t1265+t1277-t1358-t1389-t1391+t1463+t1470+t1512+t1513-t1514+t1539+t1549-t1562-t1571-t1658-t1659-t1668-t1669+t1680+t1698+t1716-t1734-t1776+t1788+t1806-t1815+t1817+t1833+t1870+t1923+t1924+t1926-t1965-t1999-t2053-t2077+t2091+t2106-t2130+t2170+t2187+t2241+t2242-t2258-t2259-t2267+t2301+t2302+t2463+t2464+t2472+t2473+t2480+t2481+t2516+t2517+t2522+t2523+t2555-t2556+t2560+t2579-t2612+t2613+(t1988.*(t1084+t13.*(t67-t512)))./2.0+t1082.*(t160-t1026).*(3.0./5.0)+(t1866.*(t499-t506))./2.0;
et22 = (t1848.*(t961-t1417))./1.0e+1-(t11.*t288.*t609)./2.0-(t11.*t288.*t1709)./2.0+t10.*t38.*(t67-t512).*1.4010416666675e-3+(t10.*t38.*(t344-t584))./2.0;
et23 = t227+t361+t396+t496+t702-t714+t743+t999-t1149-t1195+t1231+t1271+t1293+t1341+t1375-t1403+t1425+t1455-t1489-t1499-t1526-t1564+t1601-t1770+t1795+t1822-t1839-t1966+t1967-t1972-t1975+t2188+t2221-t2306-t2307-t2316+t2317-t2318+t2324+t2332+t2333+t2336+t72.*(t160-t1026).*(1.17e+2./5.0e+2)+(t2029.*(t75-t518))./2.0-t3.*t10.*t17.*2.666666666665e-5-t10.*t11.*t712.*(3.1e+1./2.5e+2);
et24 = t11.*t39.*(t71-t445).*6.810416666674999e-4+(t11.*t39.*(t386-t572))./2.0;
et25 = t9.*(-1.352e-1)-t1930.*(t441+t13.*(t69-t508))-t4.*t147+t10.*t481.*(7.0./5.0e+1)+t10.*t530.*(3.0./2.5e+1)-t4.*t586-t4.*t612.*(3.0./2.5e+1)-t292.*t798-t616.*t622+t547.*t1191.*2.0-t292.*t1876+t401.*t1890-t616.*t1695+(t640.*t1991)./5.0+t605.*t2129+t1006.*t1918-t1710.*(t69-t508)+(t655.*(t1023-t1387))./5.0+(t75-t518).*(t1135+t13.*(t69-t508).*3.333333333335e-5);
et26 = t3.*t4.*t10.*(-1.603599999999999e-2)+t10.*t11.*t291.*2.802083333335e-3-t5.*t10.*t400.*2.170133333335e-2+t10.*t11.*t594+t5.*t10.*t715.*(3.1e+1./1.25e+2)+t5.*t10.*t919.*(1.17e+2./1.0e+2)+t11.*t34.*t1275.*(3.9e+1./1.0e+2)-t5.*t10.*t1686+t10.*t11.*t1694-t11.*t39.*(t169-t960).*(1.17e+2./2.5e+2);
et27 = t261+t276+t362-t480-t717+t758+t811+t819+t829-t895+t921-t1055+t1071+t1096+t1265+t1277-t1358-t1389-t1391+t1463+t1470+t1512+t1513-t1514+t1539+t1549-t1562-t1571-t1658-t1659-t1668-t1669+t1680+t1698+t1716-t1734-t1776+t1788+t1806-t1815+t1817+t1833+t1870+t1923+t1924+t1926-t1965-t1999-t2053-t2077+t2091+t2106-t2130+t2170+t2187+t2241+t2242-t2258-t2259-t2267+t2301+t2302+t2463+t2464+t2472+t2473+t2480+t2481+t2516+t2517+t2522+t2523+t2555-t2556+t2560+t2579-t2612+t2613+(t1988.*(t1084+t13.*(t67-t512)))./2.0+t1082.*(t160-t1026).*(3.0./5.0)+(t1866.*(t499-t506))./2.0;
et28 = (t1848.*(t961-t1417))./1.0e+1-(t11.*t288.*t609)./2.0-(t11.*t288.*t1709)./2.0+t10.*t38.*(t67-t512).*1.4010416666675e-3+(t10.*t38.*(t344-t584))./2.0;
et29 = t3.*t10.*(7.0./1.25e+2)+t4.*t9.*1.68e-2+t11.*t551.*(3.1e+1./1.25e+2)+t11.*t574.*(1.17e+2./1.0e+2)-t5.*t733.*(3.9e+1./5.0e+1)+(t607.*t1519)./5.0-t294.*t1988+t403.*t2003-t694.*t1735+(t592.*(t624-t818))./5.0-t1760.*(t113-t554)+t5.*t12.*(t151+t12.*(t157-t10.*t38.*(3.9e+1./1.0e+2))).*(1.17e+2./2.5e+2)+t10.*t11.*t32.*3.779850000003e-2;
et30 = t11.*t12.*t478.*1.362083333335e-3-t6.*t11.*t526.*1.302083333335e-3+t11.*t12.*t671-t5.*t6.*t778.*(3.9e+1./1.0e+2)+t11.*t12.*t1741-t6.*t11.*t1765;
et31 = t227+t361+t396+t496+t702-t714+t743+t999-t1149-t1195+t1231+t1271+t1293+t1341+t1375-t1403+t1425+t1455-t1489-t1499-t1526-t1564+t1601-t1770+t1795+t1822-t1839-t1966+t1967-t1972-t1975+t2188+t2221-t2306-t2307-t2316+t2317-t2318+t2324+t2332+t2333+t2336+t72.*(t160-t1026).*(1.17e+2./5.0e+2)+(t2029.*(t75-t518))./2.0-t3.*t10.*t17.*2.666666666665e-5-t10.*t11.*t712.*(3.1e+1./2.5e+2);
et32 = t11.*t39.*(t71-t445).*6.810416666674999e-4+(t11.*t39.*(t386-t572))./2.0;
et33 = q_dot1.*(t1704+t2724+q_dot4.*(et21+et22)-q_dot6.*t2700+q_dot5.*t2728+q_dot3.*t2738)-q_dot3.*(t1036+t2704+t2740-q_dot5.*(et23+et24)+q_dot6.*t2687+q_dot4.*(-t140+t354+t614+t627+t683+t690+t710+t713+t734+t879+t896-t924+t954+t1007+t1014+t1037+t1038+t1047+t1099+t1104+t1160+t1184+t1190+t1199+t1246+t1334+t1348+t1350+t1360+t1416+t1461+t1506+t1537+t1540+t1563+t1587+t1616+t1657+t1774+t1793+t1797+t1838+t1942+t1963+t1964+t1978+t1982+t1984+t1996+t1997+t2037+t2038+t2065+t2066+t2249+t2250+t2263+t2284+t2285+t2293+t2298+t2299+t2319+t2320+t2328+t2329+t2377+t2378+t2382+t2383+t5.*t10.*t551.*(3.1e+1./2.5e+2))-q_dot3.*(et25+et26))+q_dot7.*(-t708+t721+t994-t1035+t1700);
et34 = q_dot4.*(-t709+t2699+q_dot1.*(et27+et28)+q_dot6.*t2684-q_dot5.*t2707-q_dot3.*(-t140+t354+t614+t627+t683+t690+t710+t713+t734+t879+t896-t924+t954+t1007+t1014+t1037+t1038+t1047+t1099+t1104+t1160+t1184+t1190+t1199+t1246+t1334+t1348+t1350+t1360+t1416+t1461+t1506+t1537+t1540+t1563+t1587+t1616+t1657+t1774+t1793+t1797+t1838+t1942+t1963+t1964+t1978+t1982+t1984+t1996+t1997+t2037+t2038+t2065+t2066+t2249+t2250+t2263+t2284+t2285+t2293+t2298+t2299+t2319+t2320+t2328+t2329+t2377+t2378+t2382+t2383+t5.*t10.*t551.*(3.1e+1./2.5e+2))+q_dot4.*(et29+et30))-q_dot6.*(t1059+t2677+t2702+q_dot5.*t2658-q_dot4.*t2684+q_dot3.*t2687);
et35 = q_dot5.*(t722+t2697+t2729+q_dot3.*(et31+et32)-q_dot6.*t2658-q_dot4.*t2707+q_dot5.*(t31.*9.672e-2+t32.*(6.2e+1./6.25e+2)+t54.*(6.2e+1./6.25e+2)+t55.*9.672e-2+t6.*t12.*t26.*5.33333333333e-5-t12.*t27.*t38.*5.33333333333e-5));
et36 = -q_dot2.*(q_dot6.*t2676-q_dot4.*t2698+q_dot3.*t2703+q_dot5.*(t782+t801-t1420-t1636-t1745-t1879-t1893+t1901+t1908+t1911+t1953+t1998-t2033-t2046+t2419-t2420+t2425+t2581+t2029.*(t509-t621)+(t1990.*(t1020-t1024))./5.0+t12.*t399.*(t71-t445).*1.362083333335e-3+t12.*t399.*(t386-t572)));
et37 = t1036+t2704+t2740;
et38 = q_dot5.*(t274+t419+t435+t524+t702-t714-t933+t999+t1149+t1167-t1195+t1207+t1280+t1293+t1341+t1375-t1403+t1425+t1455-t1489-t1499-t1526-t1564+t1601-t1770+t1795+t1822-t1839-t1966+t1967-t1972-t1975+t2188+t2221-t2306-t2307-t2316+t2317-t2318+t2324+t2332+t2333+t2336+t72.*(t160-t1026).*(1.17e+2./5.0e+2)+(t2029.*(t75-t518))./2.0+t5.*t10.*t608.*(3.1e+1./2.5e+2)+t11.*t39.*(t71-t445).*6.810416666674999e-4+(t11.*t39.*(t386-t572))./2.0);
et39 = q_dot6.*t2688-q_dot4.*t2725;
et40 = t388+t451+t494+t544+t943+t966+t1268+t1286+t1313+t1357-t1525+t1574-t1575-t1578+t1610+t1621+t1681+t1682-t1747-t1867+t1881-t1948-t1959+t1969+t1977+t2090-t2169-t2178+t2431+t2443+t2444+t2445-t2460-t2492+t2498+t2499-t2501+t2506+t2507+(t2273.*(t75-t518))./2.0+t72.*(t111.*(2.0./5.0)-t1438).*(1.17e+2./5.0e+2)-t10.*t11.*t1044.*(3.1e+1./2.5e+2)+t5.*t10.*(t67-t512).*9.4496250000075e-3;
et41 = t12.*t292.*(t67-t512).*6.810416666674999e-4+t5.*t104.*(t341-t583)+t11.*t34.*(t444-t642).*6.510416666674999e-4+(t12.*t622.*(t67-t512))./2.0+(t12.*t1695.*(t67-t512))./2.0;
et42 = t1156+t2716+q_dot2.*t2738-q_dot4.*(t262+t389+t679+t732+t744+t759+t816+t922-t939+t965+t998+t1033+t1051+t1057+t1124+t1201+t1233+t1330+t1388+t1400+t1409+t1437+t1451+t1453+t1492+t1523+t1538+t1553+t1573+t1597+t1602+t1638+t1647+t1655+t1662+t1665+t1666+t1739+t1756+t1762+t1773+t1778+t1819+t1825+t1851+t1945+t1976+t2006+t2016+t2023+t2165+t2166+t2174+t2176+t2177+t2204+t2238+t2245+t2247+t2255+t2350+t2351+t2373+t2374+t2406+t2413+t2435+t2436+t2441+t2442+t2495+t2497+t2524+t2525+t2544+t2545+t4.*t1329);
et43 = q_dot6.*(t974+t1068+t1628+t1640+t1777+t1803-t2024+t2055+t2240-t2385-t2390-t2422+t2428+t2488-t2493+(t292.*(t571-t729))./2.0+(t622.*(t444-t642))./2.0+(t7.*t640.*(t111.*(2.0./5.0)-t1438))./1.0e+1+t7.*t292.*(t1084+t13.*(t67-t512)).*1.6666666666675e-5+t13.*t947.*(t75-t518).*1.6666666666675e-5)-q_dot5.*(et40+et41);
et44 = t388+t451+t494+t544+t943+t966+t1268+t1286+t1313+t1357-t1525+t1574-t1575-t1578+t1610+t1621+t1681+t1682-t1747-t1867+t1881-t1948-t1959+t1969+t1977+t2090-t2169-t2178+t2431+t2443+t2444+t2445-t2460-t2492+t2498+t2499-t2501+t2506+t2507+(t2273.*(t75-t518))./2.0+t72.*(t111.*(2.0./5.0)-t1438).*(1.17e+2./5.0e+2)-t10.*t11.*t1044.*(3.1e+1./2.5e+2)+t5.*t10.*(t67-t512).*9.4496250000075e-3;
et45 = t12.*t292.*(t67-t512).*6.810416666674999e-4+t5.*t104.*(t341-t583)+t11.*t34.*(t444-t642).*6.510416666674999e-4+(t12.*t622.*(t67-t512))./2.0+(t12.*t1695.*(t67-t512))./2.0;
et46 = -t407;
et47 = q_dot2.*(t274+t419+t435+t524+t702-t714-t933+t999+t1149+t1167-t1195+t1207+t1280+t1293+t1341+t1375-t1403+t1425+t1455-t1489-t1499-t1526-t1564+t1601-t1770+t1795+t1822-t1839-t1966+t1967-t1972-t1975+t2188+t2221-t2306-t2307-t2316+t2317-t2318+t2324+t2332+t2333+t2336+t72.*(t160-t1026).*(1.17e+2./5.0e+2)+(t2029.*(t75-t518))./2.0+t5.*t10.*t608.*(3.1e+1./2.5e+2)+t11.*t39.*(t71-t445).*6.810416666674999e-4+(t11.*t39.*(t386-t572))./2.0);
et48 = -q_dot6.*t2571-q_dot4.*t2655+q_dot5.*(t395-t1150)+q_dot3.*(t565+t569+t680-t711-t1248+t1340-t1429-t1430-t1441-t1794+t1818+t2093+t2094-t2117+t1842.*(t75-t518))+q_dot1.*(et44+et45);
et49 = q_dot3.*(-q_dot4.*(-t564-t568+t822+t843+t937+t964+t1080+t1197+t1427+t1458+t1903+t1904+t1913+t1914+t2162+t2163+t2172+t2173)+q_dot6.*(t570-t821-t842-t883+t905+t1650+t1664+t2083+t2088)+q_dot5.*(t565+t569+t680-t711-t1248+t1340-t1429-t1430-t1441-t1794+t1818+t2093+t2094-t2117+t1842.*(t75-t518)))+q_dot2.*(et37+et38+et39);
et50 = -q_dot4.*(t662+t2679+t2726+t2734+q_dot6.*t2577+q_dot5.*t2655-q_dot4.*(t10.*1.68e-2-t395+t1150-t4.*t5.*t11.*7.12080000000333e-2+t4.*t5.*t11.*t17.*5.33333333333e-5))-q_dot1.*(et42+et43);
et51 = -q_dot6.*(t661-t2671-t2689+q_dot5.*t2571+q_dot4.*t2577+q_dot1.*(t974+t1068+t1628+t1640+t1777+t1803-t2024+t2055+t2240-t2385-t2390-t2422+t2428+t2488-t2493+(t292.*(t571-t729))./2.0+(t622.*(t444-t642))./2.0+(t7.*t640.*(t111.*(2.0./5.0)-t1438))./1.0e+1+t7.*t292.*(t1084+t13.*(t67-t512)).*1.6666666666675e-5+t13.*t947.*(t75-t518).*1.6666666666675e-5))+q_dot5.*(et46+et47+et48);
et52 = -q_dot7.*(t406+t659+t660-t1034+t1152);
et53 = t261+t276+t362-t480-t717+t758+t811+t819+t829-t895+t921-t1055+t1071+t1096+t1265+t1277-t1358-t1389-t1391+t1463+t1470+t1512+t1513-t1514+t1539+t1549-t1562-t1571-t1658-t1659-t1668-t1669+t1680+t1698+t1716-t1734-t1776+t1788+t1806-t1815+t1817+t1833+t1870+t1923+t1924+t1926-t1965-t1999-t2053-t2077+t2091+t2106-t2130+t2170+t2187+t2241+t2242-t2258-t2259-t2267+t2301+t2302+t2463+t2464+t2472+t2473+t2480+t2481+t2516+t2517+t2522+t2523+t2555-t2556+t2560+t2579-t2612+t2613+(t1988.*(t1084+t13.*(t67-t512)))./2.0+t1082.*(t160-t1026).*(3.0./5.0)+(t1866.*(t499-t506))./2.0;
et54 = (t1848.*(t961-t1417))./1.0e+1-(t11.*t288.*t609)./2.0-(t11.*t288.*t1709)./2.0+t10.*t38.*(t67-t512).*1.4010416666675e-3+(t10.*t38.*(t344-t584))./2.0;
et55 = t1498+t2714+q_dot2.*(et53+et54)-q_dot6.*(t975+t1048-t1363-t1501-t1732+t1899-t1921+t2013+t2164+t2277-t2296+t2412-t2421+t2446-t2449+t5.*t6.*(t111.*(2.0./5.0)-t1438).*(3.9e+1./1.0e+3)+(t7.*t607.*(t111.*(2.0./5.0)-t1438))./1.0e+1+t12.*t36.*(t1084+t13.*(t67-t512)).*1.6666666666675e-5+t11.*t12.*(t444-t642).*3.0e-5+(t11.*t12.*(t571-t729))./2.0)+q_dot5.*t2717;
et56 = q_dot3.*(t262+t389+t679+t732+t744+t759+t816+t922-t939+t965+t998+t1033+t1051+t1057+t1124+t1201+t1233+t1330+t1388+t1400+t1409+t1437+t1451+t1453+t1492+t1523+t1538+t1553+t1573+t1597+t1602+t1638+t1647+t1655+t1662+t1665+t1666+t1739+t1756+t1762+t1773+t1778+t1819+t1825+t1851+t1945+t1976+t2006+t2016+t2023+t2165+t2166+t2174+t2176+t2177+t2204+t2238+t2245+t2247+t2255+t2350+t2351+t2373+t2374+t2406+t2413+t2435+t2436+t2441+t2442+t2495+t2497+t2524+t2525+t2544+t2545+t4.*t1329);
et57 = -q_dot1.*(et55+et56)-q_dot5.*(t300+t2663+t2673+t2709+t2718-q_dot6.*t2348+q_dot5.*(t11.*9.672e-2+t5.*t6.*t12.*5.33333333333e-5))-q_dot7.*(t298+t299-t658-t707+t1496);
et58 = q_dot6.*(-t301+t2597+t2665-t2686+q_dot1.*(t975+t1048-t1363-t1501-t1732+t1899-t1921+t2013+t2164+t2277-t2296+t2412-t2421+t2446-t2449+t5.*t6.*(t111.*(2.0./5.0)-t1438).*(3.9e+1./1.0e+3)+(t7.*t607.*(t111.*(2.0./5.0)-t1438))./1.0e+1+t12.*t36.*(t1084+t13.*(t67-t512)).*1.6666666666675e-5+t11.*t12.*(t444-t642).*3.0e-5+(t11.*t12.*(t571-t729))./2.0)+q_dot5.*t2348)+q_dot3.*(t662+t2679+t2726+t2734+q_dot6.*t2582+q_dot5.*t2661);
et59 = q_dot4.*(q_dot6.*(t528+t767+t768+t1377+t1381+t1864+t1875+t6.*t12.*t22.*1.2e-4)-q_dot5.*t2672);
et60 = q_dot2.*(t709-t2699+t2737-q_dot6.*t2685+q_dot3.*t2725+q_dot5.*(t418+t476+t677+t692-t725-t872-t1102+t1168-t1200+t1208+t1242+t1264+t1312-t1322-t1364-t1404+t1466-t1475-t1480+t1520+t1555-t1730-t1749+t1771+t1800-t1946-t1960-t2161+t2190+t2191+t2201+t2202+t2264-t2265-t2274+t2283+t2292+(t592.*(t1020-t1024))./1.0e+1+(t1736.*(t509-t621))./2.0+t5.*t12.*(t71-t445).*6.810416666674999e-4+(t5.*t12.*(t386-t572))./2.0));
et61 = t388+t451+t494+t544+t943+t966+t1268+t1286+t1313+t1357-t1525+t1574-t1575-t1578+t1610+t1621+t1681+t1682-t1747-t1867+t1881-t1948-t1959+t1969+t1977+t2090-t2169-t2178+t2431+t2443+t2444+t2445-t2460-t2492+t2498+t2499-t2501+t2506+t2507+(t2273.*(t75-t518))./2.0+t72.*(t111.*(2.0./5.0)-t1438).*(1.17e+2./5.0e+2)-t10.*t11.*t1044.*(3.1e+1./2.5e+2)+t5.*t10.*(t67-t512).*9.4496250000075e-3;
et62 = t12.*t292.*(t67-t512).*6.810416666674999e-4+t5.*t104.*(t341-t583)+t11.*t34.*(t444-t642).*6.510416666674999e-4+(t12.*t622.*(t67-t512))./2.0+(t12.*t1695.*(t67-t512))./2.0;
et63 = -t407;
et64 = q_dot2.*(t274+t419+t435+t524+t702-t714-t933+t999+t1149+t1167-t1195+t1207+t1280+t1293+t1341+t1375-t1403+t1425+t1455-t1489-t1499-t1526-t1564+t1601-t1770+t1795+t1822-t1839-t1966+t1967-t1972-t1975+t2188+t2221-t2306-t2307-t2316+t2317-t2318+t2324+t2332+t2333+t2336+t72.*(t160-t1026).*(1.17e+2./5.0e+2)+(t2029.*(t75-t518))./2.0+t5.*t10.*t608.*(3.1e+1./2.5e+2)+t11.*t39.*(t71-t445).*6.810416666674999e-4+(t11.*t39.*(t386-t572))./2.0);
et65 = -q_dot6.*t2572+q_dot4.*t2661+q_dot3.*(t565+t569+t680-t711-t1248+t1340-t1429-t1430-t1441-t1794+t1818+t2093+t2094-t2117+t1842.*(t75-t518))+q_dot1.*(et61+et62);
et66 = t722+t2697+t2729;
et67 = q_dot3.*(t274+t419+t435+t524+t702-t714-t933+t999+t1149+t1167-t1195+t1207+t1280+t1293+t1341+t1375-t1403+t1425+t1455-t1489-t1499-t1526-t1564+t1601-t1770+t1795+t1822-t1839-t1966+t1967-t1972-t1975+t2188+t2221-t2306-t2307-t2316+t2317-t2318+t2324+t2332+t2333+t2336+t72.*(t160-t1026).*(1.17e+2./5.0e+2)+(t2029.*(t75-t518))./2.0+t5.*t10.*t608.*(3.1e+1./2.5e+2)+t11.*t39.*(t71-t445).*6.810416666674999e-4+(t11.*t39.*(t386-t572))./2.0);
et68 = -q_dot6.*t2657+q_dot4.*(t418+t476+t677+t692-t725-t872-t1102+t1168-t1200+t1208+t1242+t1264+t1312-t1322-t1364-t1404+t1466-t1475-t1480+t1520+t1555-t1730-t1749+t1771+t1800-t1946-t1960-t2161+t2190+t2191+t2201+t2202+t2264-t2265-t2274+t2283+t2292+(t592.*(t1020-t1024))./1.0e+1+(t1736.*(t509-t621))./2.0+t5.*t12.*(t71-t445).*6.810416666674999e-4+(t5.*t12.*(t386-t572))./2.0);
et69 = q_dot4;
et70 = t2662-t2673-t2718+q_dot6.*t2349+q_dot2.*(t418+t476+t677+t692-t725-t872-t1102+t1168-t1200+t1208+t1242+t1264+t1312-t1322-t1364-t1404+t1466-t1475-t1480+t1520+t1555-t1730-t1749+t1771+t1800-t1946-t1960-t2161+t2190+t2191+t2201+t2202+t2264-t2265-t2274+t2283+t2292+(t592.*(t1020-t1024))./1.0e+1+(t1736.*(t509-t621))./2.0+t5.*t12.*(t71-t445).*6.810416666674999e-4+(t5.*t12.*(t386-t572))./2.0)-q_dot7.*t5.*t12.*6.0e-5;
et71 = -1.0;
et72 = t388+t451+t494+t544+t943+t966+t1268+t1286+t1313+t1357-t1525+t1574-t1575-t1578+t1610+t1621+t1681+t1682-t1747-t1867+t1881-t1948-t1959+t1969+t1977+t2090-t2169-t2178+t2431+t2443+t2444+t2445-t2460-t2492+t2498+t2499-t2501+t2506+t2507+(t2273.*(t75-t518))./2.0+t72.*(t111.*(2.0./5.0)-t1438).*(1.17e+2./5.0e+2)-t10.*t11.*t1044.*(3.1e+1./2.5e+2)+t5.*t10.*(t67-t512).*9.4496250000075e-3;
et73 = t12.*t292.*(t67-t512).*6.810416666674999e-4+t5.*t104.*(t341-t583)+t11.*t34.*(t444-t642).*6.510416666674999e-4+(t12.*t622.*(t67-t512))./2.0+(t12.*t1695.*(t67-t512))./2.0;
et74 = t1703+t2683-q_dot4.*(t975+t1048-t1363-t1501-t1732+t1899-t1921+t2013+t2164+t2277-t2296+t2412-t2421+t2446-t2449+t5.*t6.*(t111.*(2.0./5.0)-t1438).*(3.9e+1./1.0e+3)+(t7.*t607.*(t111.*(2.0./5.0)-t1438))./1.0e+1+t12.*t36.*(t1084+t13.*(t67-t512)).*1.6666666666675e-5+t11.*t12.*(t444-t642).*3.0e-5+(t11.*t12.*(t571-t729))./2.0)+q_dot5.*t2668+q_dot2.*t2700;
c_num = ft_5({et17,et18,et19,et20,et33,et34,et35,et36,et49,et50,et51,et52,et57,et58,et59,et60,et63,et64,et65,et66,et67,et68,et69,et70,et71,et72,et73,et74,q_dot1,q_dot2,q_dot3,q_dot4,q_dot5,q_dot6,q_dot7,t1034,t1035,t1068,t1084,t111,t1152,t1153,t1157,t13,t1438,t1496,t1628,t1640,t1700,t1777,t1803,t199,t2005,t2024,t2055,t2240,t2349,t2385,t2390,t2422,t2428,t2488,t2493,t2537,t2572,t2582,t2599,t2656,t2657,t2666,t2668,t2671,t2677,t2680,t2685,t2686,t2688,t2689,t2692,t2695,t2702,t2706,t2717,t2728,t292,t296,t298,t299,t301,t405,t406,t444,t512,t518,t571,t622,t640,t642,t658,t659,t660,t661,t67,t7,t707,t708,t720,t721,t729,t75,t947,t974,t994,t995});
end
function c_num = ft_5(ct)
[et17,et18,et19,et20,et33,et34,et35,et36,et49,et50,et51,et52,et57,et58,et59,et60,et63,et64,et65,et66,et67,et68,et69,et70,et71,et72,et73,et74,q_dot1,q_dot2,q_dot3,q_dot4,q_dot5,q_dot6,q_dot7,t1034,t1035,t1068,t1084,t111,t1152,t1153,t1157,t13,t1438,t1496,t1628,t1640,t1700,t1777,t1803,t199,t2005,t2024,t2055,t2240,t2349,t2385,t2390,t2422,t2428,t2488,t2493,t2537,t2572,t2582,t2599,t2656,t2657,t2666,t2668,t2671,t2677,t2680,t2685,t2686,t2688,t2689,t2692,t2695,t2702,t2706,t2717,t2728,t292,t296,t298,t299,t301,t405,t406,t444,t512,t518,t571,t622,t640,t642,t658,t659,t660,t661,t67,t7,t707,t708,t720,t721,t729,t75,t947,t974,t994,t995] = ct{:};
et75 = q_dot3.*(t974+t1068+t1628+t1640+t1777+t1803-t2024+t2055+t2240-t2385-t2390-t2422+t2428+t2488-t2493+(t292.*(t571-t729))./2.0+(t622.*(t444-t642))./2.0+(t7.*t640.*(t111.*(2.0./5.0)-t1438))./1.0e+1+t7.*t292.*(t1084+t13.*(t67-t512)).*1.6666666666675e-5+t13.*t947.*(t75-t518).*1.6666666666675e-5);
mt1 = [et17+et18+et19+et20;et33+et34+et35+et36;et49+et50+et51+et52;et57+et58+et59+et60;-q_dot7.*(t199-t296-t405+t720+t1153)+q_dot6.*t2005-q_dot6.*t2680-q_dot3.*(et63+et64+et65)-q_dot2.*(et66+et67+et68)+et69.*et70.*et71-q_dot1.*(t1157+t2706+q_dot6.*t2668-q_dot4.*t2717+q_dot2.*t2728+q_dot3.*(et72+et73));-q_dot2.*(t995-t2677-t2702+q_dot5.*t2657-q_dot4.*t2685+q_dot3.*t2688)+q_dot7.*t2537+q_dot5.*t2680+q_dot4.*(t301+t2599+t2666+t2686+t2692+q_dot5.*t2349)+q_dot1.*(et74+et75)-q_dot3.*(-t661+t2671+t2689+t2695+q_dot5.*t2572+q_dot4.*t2582)];
mt2 = [-q_dot5.*(t199+t296+t405-t720-t1153)-q_dot2.*(t708-t721-t994+t1035+t1700)-q_dot6.*t2537+q_dot1.*t2656-q_dot4.*(t298+t299+t658+t707-t1496)-q_dot3.*(t406+t659+t660+t1034-t1152)];
c_num = [mt1;mt2];
end
